simulink model "kinovaMicoSimscapeModel"  (R2021b)
settings: Solver=VariableStepAuto  StartTime=0.0  StopTime=0.3  FixedStep=0.01  RelTol=1e-3
PostLoadFcn:
  | micoRigidBodyTreeCreation;
  | IC=deg2rad([-90,180,180,0,0,0]);
  | interactiveHomePosition=deg2rad([-90 90 177.5 90 0 0]');
  | load("./KinovaMicoSimscapeVariantConfigurations.mat");
values from neighbouring files (symbols this model uses):
  micoCandlePosition = deg2rad([0,180,180,0,0,0])    [KinovaMicoSimscapeInitializeScript.m]    (also in generatingRandomTrajectory.m)
  ViaPointsTaskSpace = [ViaPointsTaskSpace;[[pi;0;pi],[pi;0;pi],[pi;0;pi],[pi;0;pi],[0;0;0],[0;0;0],[pi;0;pi]]]    [KinovaMicoSimscapeInitializeScript.m]    (also in generatingRandomTrajectory.m = [ViaPointsTaskSpace;zeros(3,7)])
undefined symbols (not defined in the file or in its folder): Mico, ViaPointsJointSpace, X, Y, Z
libraries: sm_lib x26, nesl_utility x19, robotcorelib x4, robotmaniplib x3, pid_lib x2
(part 35 of 50)

== matlab function kinovaMicoSimscapeModel/Variant Subsystem/TaskSpaceController/Sliding Adaptive Control/RegressorComputation ==
  data: dqr input; ddqr input; Y output; dq input; q input
function Y = RegressorComputation(dqr,ddqr,dq,q)
%% Unpacking terms
ddqr1=ddqr(1);
ddqr2=ddqr(2);
ddqr3=ddqr(3);
ddqr4=ddqr(4);
ddqr5=ddqr(5);
ddqr6=ddqr(6);

dqr1=dqr(1);
dqr2=dqr(2);
dqr3=dqr(3);
dqr4=dqr(4);
dqr5=dqr(5);
dqr6=dqr(6);

dq1=dq(1);
dq2=dq(2);
dq3=dq(3);
dq4=dq(4);
dq5=dq(5);
dq6=dq(6);

q1=q(1);
q2=q(2);
q3=q(3);
q4=q(4);
q5=q(5);
q6=q(6);

%% All the terms are below
Y1_1_1=ddqr1/390625;
Y1_2_1=(525657*ddqr1)/12500000 + (29*ddqr2*cos(q2))/62500 - (841*ddqr1*cos(2*q2))/20000 - (29*dq2*dqr2*sin(q2))/62500 + (841*dq1*dqr2*sin(2*q2))/20000 + (841*dq2*dqr1*sin(2*q2))/20000;
Y1_3_1=(9935161*ddqr1)/200000000 - (35699*ddqr1*cos(q3))/1000000 - (203*ddqr2*cos(q2))/100000 - (841*ddqr1*cos(2*q2))/20000 + (203*dq2*dqr2*sin(q2))/100000 + (35699*dq1*dqr3*sin(q3))/2000000 + (35699*dq3*dqr1*sin(q3))/2000000 - (1515361*ddqr1*cos(2*q2)*cos(2*q3))/200000000 - (1515361*ddqr1*sin(2*q2)*sin(2*q3))/200000000 + (841*dq1*dqr2*sin(2*q2))/20000 + (841*dq2*dqr1*sin(2*q2))/20000 + (8617*ddqr2*cos(q2)*cos(q3))/10000000 - (8617*ddqr3*cos(q2)*cos(q3))/10000000 + (8617*ddqr2*sin(q2)*sin(q3))/10000000 - (8617*ddqr3*sin(q2)*sin(q3))/10000000 + (35699*ddqr1*cos(2*q2)*cos(q3))/1000000 + (35699*ddqr1*sin(2*q2)*sin(q3))/1000000 + (35699*dq1*dqr2*cos(2*q2)*sin(q3))/1000000 - (35699*dq1*dqr2*sin(2*q2)*cos(q3))/1000000 + (35699*dq2*dqr1*cos(2*q2)*sin(q3))/1000000 - (35699*dq2*dqr1*sin(2*q2)*cos(q3))/1000000 - (35699*dq1*dqr3*cos(2*q2)*sin(q3))/2000000 + (35699*dq1*dqr3*sin(2*q2)*cos(q3))/2000000 - (35699*dq3*dqr1*cos(2*q2)*sin(q3))/2000000 + (35699*dq3*dqr1*sin(2*q2)*cos(q3))/2000000 - (1515361*dq1*dqr2*cos(2*q2)*sin(2*q3))/200000000 + (1515361*dq1*dqr2*cos(2*q3)*sin(2*q2))/200000000 - (1515361*dq2*dqr1*cos(2*q2)*sin(2*q3))/200000000 + (1515361*dq2*dqr1*cos(2*q3)*sin(2*q2))/200000000 + (1515361*dq1*dqr3*cos(2*q2)*sin(2*q3))/200000000 - (1515361*dq1*dqr3*cos(2*q3)*sin(2*q2))/200000000 + (1515361*dq3*dqr1*cos(2*q2)*sin(2*q3))/200000000 - (1515361*dq3*dqr1*cos(2*q3)*sin(2*q2))/200000000 + (8617*dq2*dqr2*cos(q2)*sin(q3))/10000000 - (8617*dq2*dqr2*cos(q3)*sin(q2))/10000000 - (8617*dq2*dqr3*cos(q2)*sin(q3))/10000000 + (8617*dq2*dqr3*cos(q3)*sin(q2))/10000000 - (8617*dq3*dqr2*cos(q2)*sin(q3))/10000000 + (8617*dq3*dqr2*cos(q3)*sin(q2))/10000000 + (8617*dq3*dqr3*cos(q2)*sin(q3))/10000000 - (8617*dq3*dqr3*cos(q3)*sin(q2))/10000000;
Y1_4_1=(203*dq2*dqr2*sin(q2))/100000 + (3393*dq1*dqr3*sin(q3))/125000 + (3393*dq3*dqr1*sin(q3))/125000 + (259*dq4*dqr1*sin(q4))/1000000 + (841*dq1*dqr2*sin(2*q2))/20000 + (841*dq2*dqr1*sin(2*q2))/20000 - (1369*dq4*dqr1*sin(2*q4))/4000000 + (3393*dq1*dqr2*cos(2*q2)*sin(q3))/62500 - (3393*dq1*dqr2*sin(2*q2)*cos(q3))/62500 + (3393*dq2*dqr1*cos(2*q2)*sin(q3))/62500 - (3393*dq2*dqr1*sin(2*q2)*cos(q3))/62500 - (3393*dq1*dqr3*cos(2*q2)*sin(q3))/125000 + (3393*dq1*dqr3*sin(2*q2)*cos(q3))/125000 - (3393*dq3*dqr1*cos(2*q2)*sin(q3))/125000 + (3393*dq3*dqr1*sin(2*q2)*cos(q3))/125000 - (1717967*dq1*dqr2*cos(2*q2)*sin(2*q3))/100000000 + (1717967*dq1*dqr2*cos(2*q3)*sin(2*q2))/100000000 - (1717967*dq2*dqr1*cos(2*q2)*sin(2*q3))/100000000 + (1717967*dq2*dqr1*cos(2*q3)*sin(2*q2))/100000000 - (1717967*dq1*dqr3*cos(2*q3)*sin(2*q2))/100000000 + (1717967*dq3*dqr1*cos(2*q2)*sin(2*q3))/100000000 - (1717967*dq3*dqr1*cos(2*q3)*sin(2*q2))/100000000 + (819*dq2*dqr2*cos(q2)*sin(q3))/625000 - (819*dq2*dqr2*cos(q3)*sin(q2))/625000 - (1073*dq2*dqr2*cos(q4)*sin(q2))/100000 - (819*dq2*dqr3*cos(q2)*sin(q3))/625000 + (819*dq2*dqr3*cos(q3)*sin(q2))/625000 - (819*dq3*dqr2*cos(q2)*sin(q3))/625000 + (819*dq3*dqr2*cos(q3)*sin(q2))/625000 + (1073*dq1*dqr3*cos(q3)*sin(q4))/200000 + (1073*dq3*dqr1*cos(q3)*sin(q4))/200000 + (819*dq3*dqr3*cos(q2)*sin(q3))/625000 - (819*dq3*dqr3*cos(q3)*sin(q2))/625000 + (1369*dq4*dqr2*cos(q2)*sin(q3))/2000000 - (1369*dq4*dqr2*cos(q3)*sin(q2))/2000000 + (1073*dq4*dqr1*cos(q4)*sin(q3))/200000 - (1369*dq4*dqr3*cos(q2)*sin(q3))/2000000 + (1369*dq4*dqr3*cos(q3)*sin(q2))/2000000 + (1073*dq1*dqr2*cos(2*q2)*cos(q3)*sin(q4))/100000 + (1073*dq2*dqr1*cos(2*q2)*cos(q3)*sin(q4))/100000 - (1073*dq1*dqr3*cos(2*q2)*cos(q3)*sin(q4))/200000 - (1369*dq2*dqr2*sin(2*q4)*cos(q2)*cos(q3))/2000000 - (1073*dq3*dqr1*cos(2*q2)*cos(q3)*sin(q4))/200000 + (1369*dq2*dqr3*sin(2*q4)*cos(q2)*cos(q3))/2000000 + (1369*dq3*dqr2*sin(2*q4)*cos(q2)*cos(q3))/2000000 - (1073*dq4*dqr1*cos(2*q2)*cos(q4)*sin(q3))/200000 + (1073*dq4*dqr1*sin(2*q2)*cos(q3)*cos(q4))/200000 - (1369*dq3*dqr3*sin(2*q4)*cos(q2)*cos(q3))/2000000 + (1369*dq4*dqr2*cos(2*q4)*cos(q2)*sin(q3))/2000000 - (1369*dq4*dqr2*cos(2*q4)*cos(q3)*sin(q2))/2000000 - (1369*dq4*dqr3*cos(2*q4)*cos(q2)*sin(q3))/2000000 + (1369*dq4*dqr3*cos(2*q4)*cos(q3)*sin(q2))/2000000 + (1073*dq1*dqr2*sin(2*q2)*sin(q3)*sin(q4))/100000 + (1073*dq2*dqr1*sin(2*q2)*sin(q3)*sin(q4))/100000 - (1073*dq1*dqr3*sin(2*q2)*sin(q3)*sin(q4))/200000 - (1369*dq2*dqr2*sin(2*q4)*sin(q2)*sin(q3))/2000000 - (1073*dq3*dqr1*sin(2*q2)*sin(q3)*sin(q4))/200000 + (1369*dq2*dqr3*sin(2*q4)*sin(q2)*sin(q3))/2000000 + (1369*dq3*dqr2*sin(2*q4)*sin(q2)*sin(q3))/2000000 - (1369*dq3*dqr3*sin(2*q4)*sin(q2)*sin(q3))/2000000 - (4329*dq1*dqr2*cos(2*q2)*cos(2*q3)*sin(q4))/625000 - (4329*dq2*dqr1*cos(2*q2)*cos(2*q3)*sin(q4))/625000 + (4329*dq1*dqr3*cos(2*q2)*cos(2*q3)*sin(q4))/625000 + (4329*dq3*dqr1*cos(2*q2)*cos(2*q3)*sin(q4))/625000 + (4329*dq4*dqr1*cos(2*q2)*sin(2*q3)*cos(q4))/1250000 - (4329*dq4*dqr1*cos(2*q3)*sin(2*q2)*cos(q4))/1250000 - (4329*dq1*dqr2*sin(2*q2)*sin(2*q3)*sin(q4))/625000 - (4329*dq2*dqr1*sin(2*q2)*sin(2*q3)*sin(q4))/625000 + (4329*dq1*dqr3*sin(2*q2)*sin(2*q3)*sin(q4))/625000 + (4329*dq3*dqr1*sin(2*q2)*sin(2*q3)*sin(q4))/625000 + (259*dq2*dqr2*cos(q2)*cos(q3)*sin(q4))/1000000 - (4329*dq2*dqr2*cos(q2)*cos(q4)*sin(q3))/625000 + (4329*dq2*dqr2*cos(q3)*cos(q4)*sin(q2))/625000 - (259*dq2*dqr3*cos(q2)*cos(q3)*sin(q4))/1000000 + (4329*dq2*dqr3*cos(q2)*cos(q4)*sin(q3))/625000 - (4329*dq2*dqr3*cos(q3)*cos(q4)*sin(q2))/625000 - (259*dq3*dqr2*cos(q2)*cos(q3)*sin(q4))/1000000 + (4329*dq3*dqr2*cos(q2)*cos(q4)*sin(q3))/625000 - (4329*dq3*dqr2*cos(q3)*cos(q4)*sin(q2))/625000 + (259*dq3*dqr3*cos(q2)*cos(q3)*sin(q4))/1000000 - (4329*dq3*dqr3*cos(q2)*cos(q4)*sin(q3))/625000 + (4329*dq3*dqr3*cos(q3)*cos(q4)*sin(q2))/625000 - (259*dq4*dqr2*cos(q2)*cos(q4)*sin(q3))/1000000 + (259*dq4*dqr2*cos(q3)*cos(q4)*sin(q2))/1000000 + (259*dq4*dqr3*cos(q2)*cos(q4)*sin(q3))/1000000 - (259*dq4*dqr3*cos(q3)*cos(q4)*sin(q2))/1000000 - (1369*dq1*dqr2*cos(2*q2)*cos(2*q4)*sin(2*q3))/4000000 + (1369*dq1*dqr2*cos(2*q3)*cos(2*q4)*sin(2*q2))/4000000 - (1369*dq2*dqr1*cos(2*q2)*cos(2*q4)*sin(2*q3))/4000000 + (1369*dq2*dqr1*cos(2*q3)*cos(2*q4)*sin(2*q2))/4000000 + (1369*dq1*dqr3*cos(2*q2)*cos(2*q4)*sin(2*q3))/4000000 - (1369*dq1*dqr3*cos(2*q3)*cos(2*q4)*sin(2*q2))/4000000 + (1369*dq3*dqr1*cos(2*q2)*cos(2*q4)*sin(2*q3))/4000000 - (1369*dq3*dqr1*cos(2*q3)*cos(2*q4)*sin(2*q2))/4000000 + (1369*dq4*dqr1*cos(2*q2)*cos(2*q3)*sin(2*q4))/4000000 + (259*dq2*dqr2*sin(q2)*sin(q3)*sin(q4))/1000000 - (259*dq2*dqr3*sin(q2)*sin(q3)*sin(q4))/1000000 - (259*dq3*dqr2*sin(q2)*sin(q3)*sin(q4))/1000000 + (259*dq3*dqr3*sin(q2)*sin(q3)*sin(q4))/1000000 + (1369*dq4*dqr1*sin(2*q2)*sin(2*q3)*sin(2*q4))/4000000;
Y1_4_2=(6064767*ddqr1)/100000000 - (3393*ddqr1*cos(q3))/62500 - (203*ddqr2*cos(q2))/100000 - (259*ddqr1*cos(q4))/500000 - (841*ddqr1*cos(2*q2))/20000 + (1369*ddqr1*cos(2*q4))/4000000 + (259*dq1*dqr4*sin(q4))/1000000 - (1717967*ddqr1*cos(2*q2)*cos(2*q3))/100000000 - (1717967*ddqr1*sin(2*q2)*sin(2*q3))/100000000 - (1369*dq1*dqr4*sin(2*q4))/4000000 + (819*ddqr2*cos(q2)*cos(q3))/625000 + (1073*ddqr2*cos(q2)*cos(q4))/100000 - (819*ddqr3*cos(q2)*cos(q3))/625000 + (1369*ddqr4*cos(q2)*cos(q3))/1000000 + (819*ddqr2*sin(q2)*sin(q3))/625000 + (1073*ddqr1*sin(q3)*sin(q4))/100000 - (819*ddqr3*sin(q2)*sin(q3))/625000 + (1369*ddqr4*sin(q2)*sin(q3))/1000000 + (1073*ddqr4*sin(q2)*sin(q4))/100000 + (3393*ddqr1*cos(2*q2)*cos(q3))/62500 + (3393*ddqr1*sin(2*q2)*sin(q3))/62500 + (4329*ddqr1*cos(2*q2)*sin(2*q3)*sin(q4))/625000 - (4329*ddqr1*cos(2*q3)*sin(2*q2)*sin(q4))/625000 - (4329*ddqr2*cos(q2)*cos(q3)*cos(q4))/625000 + (4329*ddqr3*cos(q2)*cos(q3)*cos(q4))/625000 - (259*ddqr4*cos(q2)*cos(q3)*cos(q4))/1000000 - (1369*ddqr1*cos(2*q2)*cos(2*q3)*cos(2*q4))/4000000 - (259*ddqr2*cos(q2)*sin(q3)*sin(q4))/1000000 + (259*ddqr2*cos(q3)*sin(q2)*sin(q4))/1000000 - (4329*ddqr2*cos(q4)*sin(q2)*sin(q3))/625000 + (259*ddqr3*cos(q2)*sin(q3)*sin(q4))/1000000 - (259*ddqr3*cos(q3)*sin(q2)*sin(q4))/1000000 + (4329*ddqr3*cos(q4)*sin(q2)*sin(q3))/625000 + (4329*ddqr4*cos(q2)*sin(q3)*sin(q4))/625000 - (4329*ddqr4*cos(q3)*sin(q2)*sin(q4))/625000 - (259*ddqr4*cos(q4)*sin(q2)*sin(q3))/1000000 - (1369*ddqr1*cos(2*q4)*sin(2*q2)*sin(2*q3))/4000000 + (1717967*dq1*dqr3*cos(2*q2)*sin(2*q3))/100000000 - (1073*ddqr1*cos(2*q2)*sin(q3)*sin(q4))/100000 + (1073*ddqr1*sin(2*q2)*cos(q3)*sin(q4))/100000 + (1369*ddqr2*sin(2*q4)*cos(q2)*sin(q3))/2000000 - (1369*ddqr2*sin(2*q4)*cos(q3)*sin(q2))/2000000 - (1369*ddqr3*sin(2*q4)*cos(q2)*sin(q3))/2000000 + (1369*ddqr3*sin(2*q4)*cos(q3)*sin(q2))/2000000 + (1369*dq2*dqr4*cos(q2)*sin(q3))/2000000 - (1369*dq2*dqr4*cos(q3)*sin(q2))/2000000 + (1073*dq1*dqr4*cos(q4)*sin(q3))/200000 - (1369*dq3*dqr4*cos(q2)*sin(q3))/2000000 + (1369*dq3*dqr4*cos(q3)*sin(q2))/2000000 + (1073*dq4*dqr4*cos(q4)*sin(q2))/100000 - (1073*dq1*dqr4*cos(2*q2)*cos(q4)*sin(q3))/200000 + (1073*dq1*dqr4*sin(2*q2)*cos(q3)*cos(q4))/200000 + (1369*dq2*dqr4*cos(2*q4)*cos(q2)*sin(q3))/2000000 - (1369*dq2*dqr4*cos(2*q4)*cos(q3)*sin(q2))/2000000 - (1369*dq3*dqr4*cos(2*q4)*cos(q2)*sin(q3))/2000000 + (1369*dq3*dqr4*cos(2*q4)*cos(q3)*sin(q2))/2000000 + (4329*dq1*dqr4*cos(2*q2)*sin(2*q3)*cos(q4))/1250000 - (4329*dq1*dqr4*cos(2*q3)*sin(2*q2)*cos(q4))/1250000 - (259*dq2*dqr4*cos(q2)*cos(q4)*sin(q3))/1000000 + (259*dq2*dqr4*cos(q3)*cos(q4)*sin(q2))/1000000 + (259*dq3*dqr4*cos(q2)*cos(q4)*sin(q3))/1000000 - (259*dq3*dqr4*cos(q3)*cos(q4)*sin(q2))/1000000 + (259*dq4*dqr4*cos(q2)*cos(q3)*sin(q4))/1000000 + (4329*dq4*dqr4*cos(q2)*cos(q4)*sin(q3))/625000 - (4329*dq4*dqr4*cos(q3)*cos(q4)*sin(q2))/625000 + (1369*dq1*dqr4*cos(2*q2)*cos(2*q3)*sin(2*q4))/4000000 + (259*dq4*dqr4*sin(q2)*sin(q3)*sin(q4))/1000000 + (1369*dq1*dqr4*sin(2*q2)*sin(2*q3)*sin(2*q4))/4000000;
Y1_5_1=(25433*dq3*dqr1*sin(q3))/800000 + dq4*dqr1*sin(q4)*((4487*3^(1/2))/20000000 + 259/1000000) - dq5*dqr1*sin(q5)*((253339*3^(1/2))/160000000 - 4107/8000000) + (25433*dq2*dqr1*cos(2*q2)*sin(q3))/400000 - (25433*dq2*dqr1*sin(2*q2)*cos(q3))/400000 - (25433*dq3*dqr1*cos(2*q2)*sin(q3))/800000 + (25433*dq3*dqr1*sin(2*q2)*cos(q3))/800000 - (259*dq4*dqr1*cos(q4)*sin(q5))/1000000 - (259*dq4*dqr1*cos(q5)*sin(q4))/2000000 - (259*dq5*dqr1*cos(q4)*sin(q5))/2000000 - (259*dq5*dqr1*cos(q5)*sin(q4))/1000000 + (1073*3^(1/2)*dq3*dqr1*cos(q5)*sin(q3))/400000 + (1073*3^(1/2)*dq5*dqr1*cos(q3)*sin(q5))/400000 + dq4*dqr1*cos(2*q4)*sin(q5)*((23717*3^(1/2))/40000000 + 1369/2000000) + dq5*dqr1*cos(2*q4)*sin(q5)*((23717*3^(1/2))/160000000 + 1369/8000000) - (1073*dq3*dqr1*cos(q3)*cos(q4)*sin(q5))/200000 - (1073*dq3*dqr1*cos(q3)*cos(q5)*sin(q4))/400000 - (1073*dq4*dqr1*cos(q4)*cos(q5)*sin(q3))/400000 - (1073*dq5*dqr1*cos(q4)*cos(q5)*sin(q3))/200000 + (1073*dq4*dqr1*sin(q3)*sin(q4)*sin(q5))/200000 + (1073*dq5*dqr1*sin(q3)*sin(q4)*sin(q5))/400000 + dq3*dqr1*cos(q3)*sin(q4)*((18589*3^(1/2))/4000000 + 1073/200000) + dq4*dqr1*cos(q4)*sin(q3)*((18589*3^(1/2))/4000000 + 1073/200000) - (1073*dq2*dqr1*sin(2*q2)*cos(q4)*sin(q3)*sin(q5))/100000 - (1073*dq2*dqr1*sin(2*q2)*cos(q5)*sin(q3)*sin(q4))/200000 + (1073*dq3*dqr1*sin(2*q2)*cos(q4)*sin(q3)*sin(q5))/200000 + (1073*dq3*dqr1*sin(2*q2)*cos(q5)*sin(q3)*sin(q4))/400000 - (1073*dq4*dqr1*cos(2*q2)*sin(q3)*sin(q4)*sin(q5))/200000 + (1073*dq4*dqr1*sin(2*q2)*cos(q3)*sin(q4)*sin(q5))/200000 - (1073*dq5*dqr1*cos(2*q2)*sin(q3)*sin(q4)*sin(q5))/400000 + (1073*dq5*dqr1*sin(2*q2)*cos(q3)*sin(q4)*sin(q5))/400000 + dq2*dqr1*cos(2*q2)*cos(q3)*sin(q4)*((18589*3^(1/2))/2000000 + 1073/100000) - dq3*dqr1*cos(2*q2)*cos(q3)*sin(q4)*((18589*3^(1/2))/4000000 + 1073/200000) - dq4*dqr1*cos(2*q2)*cos(q4)*sin(q3)*((18589*3^(1/2))/4000000 + 1073/200000) + dq4*dqr1*sin(2*q2)*cos(q3)*cos(q4)*((18589*3^(1/2))/4000000 + 1073/200000) + (32449*dq2*dqr1*cos(2*q2)*cos(2*q3)*cos(q4)*sin(q5))/4000000 - (32449*dq3*dqr1*cos(2*q2)*cos(2*q3)*cos(q4)*sin(q5))/4000000 - (32449*dq5*dqr1*cos(2*q2)*sin(2*q3)*cos(q4)*cos(q5))/8000000 + (32449*dq5*dqr1*cos(2*q3)*sin(2*q2)*cos(q4)*cos(q5))/8000000 + dq2*dqr1*sin(2*q2)*sin(q3)*sin(q4)*((18589*3^(1/2))/2000000 + 1073/100000) - dq3*dqr1*sin(2*q2)*sin(q3)*sin(q4)*((18589*3^(1/2))/4000000 + 1073/200000) + (32449*dq2*dqr1*sin(2*q2)*sin(2*q3)*cos(q4)*sin(q5))/4000000 - (32449*dq3*dqr1*sin(2*q2)*sin(2*q3)*cos(q4)*sin(q5))/4000000 + (32449*dq4*dqr1*cos(2*q2)*sin(2*q3)*sin(q4)*sin(q5))/8000000 - (32449*dq4*dqr1*cos(2*q3)*sin(2*q2)*sin(q4)*sin(q5))/8000000 + (1073*3^(1/2)*dq2*dqr1*cos(2*q2)*cos(q5)*sin(q3))/200000 - (1073*3^(1/2)*dq2*dqr1*sin(2*q2)*cos(q3)*cos(q5))/200000 - (1073*3^(1/2)*dq3*dqr1*cos(2*q2)*cos(q5)*sin(q3))/400000 + (1073*3^(1/2)*dq3*dqr1*sin(2*q2)*cos(q3)*cos(q5))/400000 - (1073*3^(1/2)*dq5*dqr1*cos(2*q2)*cos(q3)*sin(q5))/400000 - (1073*3^(1/2)*dq5*dqr1*sin(2*q2)*sin(q3)*sin(q5))/400000 - dq2*dqr1*cos(2*q2)*cos(2*q3)*sin(q4)*((548467*3^(1/2))/80000000 + 32449/4000000) + dq3*dqr1*cos(2*q2)*cos(2*q3)*sin(q4)*((548467*3^(1/2))/80000000 + 32449/4000000) + dq5*dqr1*cos(2*q2)*cos(2*q3)*sin(q5)*((348207*3^(1/2))/160000000 + 1369/8000000) + dq4*dqr1*cos(2*q2)*sin(2*q3)*cos(q4)*((548467*3^(1/2))/160000000 + 32449/8000000) - dq4*dqr1*cos(2*q3)*sin(2*q2)*cos(q4)*((548467*3^(1/2))/160000000 + 32449/8000000) - dq2*dqr1*sin(2*q2)*sin(2*q3)*sin(q4)*((548467*3^(1/2))/80000000 + 32449/4000000) + dq3*dqr1*sin(2*q2)*sin(2*q3)*sin(q4)*((548467*3^(1/2))/80000000 + 32449/4000000) + dq5*dqr1*sin(2*q2)*sin(2*q3)*sin(q5)*((348207*3^(1/2))/160000000 + 1369/8000000) - (1073*dq2*dqr1*cos(2*q2)*cos(q3)*cos(q4)*sin(q5))/100000 - (1073*dq2*dqr1*cos(2*q2)*cos(q3)*cos(q5)*sin(q4))/200000 + (1073*dq3*dqr1*cos(2*q2)*cos(q3)*cos(q4)*sin(q5))/200000 + (1073*dq3*dqr1*cos(2*q2)*cos(q3)*cos(q5)*sin(q4))/400000 + (1073*dq4*dqr1*cos(2*q2)*cos(q4)*cos(q5)*sin(q3))/400000 - (1073*dq4*dqr1*sin(2*q2)*cos(q3)*cos(q4)*cos(q5))/400000 + (1073*dq5*dqr1*cos(2*q2)*cos(q4)*cos(q5)*sin(q3))/200000 - (1073*dq5*dqr1*sin(2*q2)*cos(q3)*cos(q4)*cos(q5))/200000 + (1369*3^(1/2)*dq2*dqr1*cos(2*q2)*cos(2*q3)*cos(2*q5)*sin(q4))/8000000 + (1369*3^(1/2)*dq2*dqr1*cos(2*q2)*cos(2*q3)*sin(2*q5)*cos(q4))/4000000 - (1369*3^(1/2)*dq3*dqr1*cos(2*q2)*cos(2*q3)*cos(2*q5)*sin(q4))/8000000 - (1369*3^(1/2)*dq3*dqr1*cos(2*q2)*cos(2*q3)*sin(2*q5)*cos(q4))/4000000 - (1369*3^(1/2)*dq4*dqr1*cos(2*q2)*cos(2*q5)*sin(2*q3)*cos(q4))/16000000 + (1369*3^(1/2)*dq4*dqr1*cos(2*q3)*cos(2*q5)*sin(2*q2)*cos(q4))/16000000 - (1369*3^(1/2)*dq5*dqr1*cos(2*q2)*cos(2*q5)*sin(2*q3)*cos(q4))/4000000 + (1369*3^(1/2)*dq5*dqr1*cos(2*q3)*cos(2*q5)*sin(2*q2)*cos(q4))/4000000 + (1369*3^(1/2)*dq2*dqr1*cos(2*q5)*sin(2*q2)*sin(2*q3)*sin(q4))/8000000 + (1369*3^(1/2)*dq2*dqr1*sin(2*q2)*sin(2*q3)*sin(2*q5)*cos(q4))/4000000 - (1369*3^(1/2)*dq3*dqr1*cos(2*q5)*sin(2*q2)*sin(2*q3)*sin(q4))/8000000 - (1369*3^(1/2)*dq3*dqr1*sin(2*q2)*sin(2*q3)*sin(2*q5)*cos(q4))/4000000 + (1369*3^(1/2)*dq4*dqr1*cos(2*q2)*sin(2*q3)*sin(2*q5)*sin(q4))/8000000 - (1369*3^(1/2)*dq4*dqr1*cos(2*q3)*sin(2*q2)*sin(2*q5)*sin(q4))/8000000 + (1369*3^(1/2)*dq5*dqr1*cos(2*q2)*sin(2*q3)*sin(2*q5)*sin(q4))/8000000 - (1369*3^(1/2)*dq5*dqr1*cos(2*q3)*sin(2*q2)*sin(2*q5)*sin(q4))/8000000 - dq2*dqr1*cos(2*q2)*cos(2*q3)*cos(q5)*sin(q4)*((1369*3^(1/2))/2000000 - 45547/20000000) + dq3*dqr1*cos(2*q2)*cos(2*q3)*cos(q5)*sin(q4)*((1369*3^(1/2))/2000000 - 45547/20000000) + dq4*dqr1*cos(2*q2)*sin(2*q3)*cos(q4)*cos(q5)*((1369*3^(1/2))/4000000 - 45547/40000000) - dq4*dqr1*cos(2*q3)*sin(2*q2)*cos(q4)*cos(q5)*((1369*3^(1/2))/4000000 - 45547/40000000) - dq2*dqr1*sin(2*q2)*sin(2*q3)*cos(q5)*sin(q4)*((1369*3^(1/2))/2000000 - 45547/20000000) + dq3*dqr1*sin(2*q2)*sin(2*q3)*cos(q5)*sin(q4)*((1369*3^(1/2))/2000000 - 45547/20000000) - dq5*dqr1*cos(2*q2)*sin(2*q3)*sin(q4)*sin(q5)*((1369*3^(1/2))/4000000 - 45547/40000000) + dq5*dqr1*cos(2*q3)*sin(2*q2)*sin(q4)*sin(q5)*((1369*3^(1/2))/4000000 - 45547/40000000) - dq4*dqr1*cos(2*q2)*cos(2*q3)*cos(2*q4)*sin(q5)*((23717*3^(1/2))/40000000 + 1369/2000000) - dq2*dqr1*cos(2*q3)*cos(2*q4)*sin(2*q2)*cos(q5)*((23717*3^(1/2))/80000000 + 1369/4000000) - dq5*dqr1*cos(2*q2)*cos(2*q3)*cos(2*q4)*sin(q5)*((23717*3^(1/2))/160000000 + 1369/8000000) - dq2*dqr1*cos(2*q2)*sin(2*q3)*sin(2*q4)*sin(q5)*((23717*3^(1/2))/40000000 + 1369/2000000) + dq2*dqr1*cos(2*q3)*sin(2*q2)*sin(2*q4)*sin(q5)*((23717*3^(1/2))/40000000 + 1369/2000000) + dq3*dqr1*cos(2*q2)*sin(2*q3)*sin(2*q4)*sin(q5)*((23717*3^(1/2))/40000000 + 1369/2000000) - dq3*dqr1*cos(2*q3)*sin(2*q2)*sin(2*q4)*sin(q5)*((23717*3^(1/2))/40000000 + 1369/2000000) - dq4*dqr1*cos(2*q4)*sin(2*q2)*sin(2*q3)*sin(q5)*((23717*3^(1/2))/40000000 + 1369/2000000) - dq5*dqr1*cos(2*q4)*sin(2*q2)*sin(2*q3)*sin(q5)*((23717*3^(1/2))/160000000 + 1369/8000000);
Y1_5_2=(841*dq2*dqr1*sin(2*q2))/20000 + (4107*dq5*dqr1*sin(2*q5))/32000000 - (1369*dq4*dqr1*cos(2*q4)*sin(2*q5))/8000000 - (1369*dq4*dqr1*cos(2*q5)*sin(2*q4))/6400000 - (1369*dq5*dqr1*cos(2*q4)*sin(2*q5))/6400000 - (1369*dq5*dqr1*cos(2*q5)*sin(2*q4))/8000000 - (6139*dq2*dqr2*cos(q3)*sin(q2))/4000000 + (6139*dq3*dqr2*cos(q3)*sin(q2))/4000000 - dq4*dqr1*sin(2*q4)*((23717*3^(1/2))/40000000 + 1574893/1600000000) + dq2*dqr1*cos(2*q2)*sin(2*q3)*((23717*3^(1/2))/40000000 - 36744657/1600000000) - dq2*dqr1*cos(2*q3)*sin(2*q2)*((23717*3^(1/2))/40000000 - 36744657/1600000000) - dq3*dqr1*cos(2*q2)*sin(2*q3)*((23717*3^(1/2))/40000000 - 36744657/1600000000) + dq3*dqr1*cos(2*q3)*sin(2*q2)*((23717*3^(1/2))/40000000 - 36744657/1600000000) + dq4*dqr1*sin(2*q4)*cos(q5)*((23717*3^(1/2))/80000000 + 1369/4000000) + dq5*dqr1*sin(2*q4)*cos(q5)*((23717*3^(1/2))/80000000 + 1369/4000000) - (12321*dq2*dqr1*cos(2*q2)*cos(2*q5)*sin(2*q3))/32000000 + (12321*dq2*dqr1*cos(2*q3)*cos(2*q5)*sin(2*q2))/32000000 + (12321*dq3*dqr1*cos(2*q2)*cos(2*q5)*sin(2*q3))/32000000 - (12321*dq3*dqr1*cos(2*q3)*cos(2*q5)*sin(2*q2))/32000000 + (12321*dq5*dqr1*cos(2*q2)*cos(2*q3)*sin(2*q5))/32000000 - (1073*dq2*dqr2*sin(q2)*sin(q4)*sin(q5))/100000 + (12321*dq5*dqr1*sin(2*q2)*sin(2*q3)*sin(2*q5))/32000000 - (1369*dq2*dqr1*cos(2*q2)*cos(2*q4)*cos(2*q5)*sin(2*q3))/6400000 + (1369*dq2*dqr1*cos(2*q3)*cos(2*q4)*cos(2*q5)*sin(2*q2))/6400000 + (1369*dq3*dqr1*cos(2*q2)*cos(2*q4)*cos(2*q5)*sin(2*q3))/6400000 - (1369*dq3*dqr1*cos(2*q3)*cos(2*q4)*cos(2*q5)*sin(2*q2))/6400000 + (1369*dq4*dqr1*cos(2*q2)*cos(2*q3)*cos(2*q4)*sin(2*q5))/8000000 + (1369*dq4*dqr1*cos(2*q2)*cos(2*q3)*cos(2*q5)*sin(2*q4))/6400000 + (1369*dq5*dqr1*cos(2*q2)*cos(2*q3)*cos(2*q4)*sin(2*q5))/6400000 + (1369*dq5*dqr1*cos(2*q2)*cos(2*q3)*cos(2*q5)*sin(2*q4))/8000000 - (259*3^(1/2)*dq2*dqr2*cos(q3)*cos(q5)*sin(q2))/2000000 + (259*3^(1/2)*dq3*dqr2*cos(q3)*cos(q5)*sin(q2))/2000000 + (1369*dq2*dqr1*cos(2*q2)*sin(2*q3)*sin(2*q4)*sin(2*q5))/8000000 - (1369*dq2*dqr1*cos(2*q3)*sin(2*q2)*sin(2*q4)*sin(2*q5))/8000000 - (1369*dq3*dqr1*cos(2*q2)*sin(2*q3)*sin(2*q4)*sin(2*q5))/8000000 + (1369*dq3*dqr1*cos(2*q3)*sin(2*q2)*sin(2*q4)*sin(2*q5))/8000000 + (1369*dq4*dqr1*cos(2*q4)*sin(2*q2)*sin(2*q3)*sin(2*q5))/8000000 + (1369*dq4*dqr1*cos(2*q5)*sin(2*q2)*sin(2*q3)*sin(2*q4))/6400000 + (1369*dq5*dqr1*cos(2*q4)*sin(2*q2)*sin(2*q3)*sin(2*q5))/6400000 + (1369*dq5*dqr1*cos(2*q5)*sin(2*q2)*sin(2*q3)*sin(2*q4))/8000000 + (1369*3^(1/2)*dq5*dqr2*sin(q2)*sin(q3)*sin(q4))/4000000 - (259*3^(1/2)*dq5*dqr2*sin(q2)*sin(q3)*sin(q5))/2000000 - dq2*dqr1*cos(2*q2)*cos(2*q4)*sin(2*q3)*((23717*3^(1/2))/40000000 + 1574893/1600000000) + dq2*dqr1*cos(2*q3)*cos(2*q4)*sin(2*q2)*((23717*3^(1/2))/40000000 + 1574893/1600000000) + dq3*dqr1*cos(2*q2)*cos(2*q4)*sin(2*q3)*((23717*3^(1/2))/40000000 + 1574893/1600000000) - dq3*dqr1*cos(2*q3)*cos(2*q4)*sin(2*q2)*((23717*3^(1/2))/40000000 + 1574893/1600000000) + dq4*dqr1*cos(2*q2)*cos(2*q3)*sin(2*q4)*((23717*3^(1/2))/40000000 + 1574893/1600000000) - (1369*dq2*dqr2*cos(2*q4)*sin(2*q5)*sin(q2)*sin(q3))/4000000 - (1369*dq2*dqr2*cos(2*q5)*sin(2*q4)*sin(q2)*sin(q3))/3200000 + (1369*dq3*dqr2*cos(2*q4)*sin(2*q5)*sin(q2)*sin(q3))/4000000 + (1369*dq3*dqr2*cos(2*q5)*sin(2*q4)*sin(q2)*sin(q3))/3200000 + (1369*dq4*dqr2*sin(2*q4)*sin(2*q5)*cos(q3)*sin(q2))/4000000 + dq4*dqr1*sin(2*q2)*sin(2*q3)*sin(2*q4)*((23717*3^(1/2))/40000000 + 1574893/1600000000) - dq2*dqr2*sin(2*q4)*sin(q2)*sin(q3)*((23717*3^(1/2))/20000000 + 1574893/800000000) + dq3*dqr2*sin(2*q4)*sin(q2)*sin(q3)*((23717*3^(1/2))/20000000 + 1574893/800000000) - (259*dq4*dqr2*cos(q3)*cos(q4)*cos(q5)*sin(q2))/2000000 - (259*dq5*dqr2*cos(q3)*cos(q4)*cos(q5)*sin(q2))/1000000 - dq2*dqr1*cos(2*q2)*sin(2*q3)*cos(q5)*((348207*3^(1/2))/80000000 + 1369/4000000) + dq2*dqr1*cos(2*q3)*sin(2*q2)*cos(q5)*((348207*3^(1/2))/80000000 + 1369/4000000) + dq3*dqr1*cos(2*q2)*sin(2*q3)*cos(q5)*((348207*3^(1/2))/80000000 + 1369/4000000) - dq3*dqr1*cos(2*q3)*sin(2*q2)*cos(q5)*((348207*3^(1/2))/80000000 + 1369/4000000) + (32449*dq2*dqr2*cos(q3)*sin(q2)*sin(q4)*sin(q5))/4000000 - (259*dq2*dqr2*cos(q4)*sin(q2)*sin(q3)*sin(q5))/1000000 - (259*dq2*dqr2*cos(q5)*sin(q2)*sin(q3)*sin(q4))/2000000 - (32449*dq3*dqr2*cos(q3)*sin(q2)*sin(q4)*sin(q5))/4000000 + (259*dq3*dqr2*cos(q4)*sin(q2)*sin(q3)*sin(q5))/1000000 + (259*dq3*dqr2*cos(q5)*sin(q2)*sin(q3)*sin(q4))/2000000 + (259*dq4*dqr2*cos(q3)*sin(q2)*sin(q4)*sin(q5))/1000000 + (259*dq5*dqr2*cos(q3)*sin(q2)*sin(q4)*sin(q5))/2000000 + dq4*dqr2*cos(q3)*cos(q4)*sin(q2)*((4487*3^(1/2))/20000000 + 259/1000000) + dq4*dqr2*cos(q3)*cos(q5)*sin(q2)*((23717*3^(1/2))/40000000 + 1369/2000000) + dq5*dqr2*cos(q3)*cos(q5)*sin(q2)*((23717*3^(1/2))/40000000 + 1369/2000000) + dq2*dqr2*cos(q3)*cos(q4)*sin(q2)*((548467*3^(1/2))/80000000 + 32449/4000000) - dq3*dqr2*cos(q3)*cos(q4)*sin(q2)*((548467*3^(1/2))/80000000 + 32449/4000000) + dq2*dqr2*sin(q2)*sin(q3)*sin(q4)*((4487*3^(1/2))/20000000 + 259/1000000) - dq3*dqr2*sin(q2)*sin(q3)*sin(q4)*((4487*3^(1/2))/20000000 + 259/1000000) + dq4*dqr2*cos(2*q4)*cos(q3)*cos(q5)*sin(q2)*((23717*3^(1/2))/40000000 + 1369/2000000) + dq5*dqr2*cos(2*q4)*cos(q3)*cos(q5)*sin(q2)*((23717*3^(1/2))/40000000 + 1369/2000000) + dq2*dqr2*cos(2*q4)*sin(q2)*sin(q3)*sin(q5)*((23717*3^(1/2))/20000000 + 1369/1000000) - dq3*dqr2*cos(2*q4)*sin(q2)*sin(q3)*sin(q5)*((23717*3^(1/2))/20000000 + 1369/1000000) - dq4*dqr2*sin(2*q4)*cos(q3)*sin(q2)*sin(q5)*((23717*3^(1/2))/20000000 + 1369/1000000) + dq2*dqr2*sin(2*q4)*cos(q5)*sin(q2)*sin(q3)*((23717*3^(1/2))/40000000 + 1369/2000000) - dq3*dqr2*sin(2*q4)*cos(q5)*sin(q2)*sin(q3)*((23717*3^(1/2))/40000000 + 1369/2000000) - dq5*dqr2*sin(2*q4)*cos(q3)*sin(q2)*sin(q5)*((23717*3^(1/2))/80000000 + 1369/4000000) - (1369*3^(1/2)*dq2*dqr2*cos(2*q5)*cos(q3)*cos(q4)*sin(q2))/8000000 + (1369*3^(1/2)*dq3*dqr2*cos(2*q5)*cos(q3)*cos(q4)*sin(q2))/8000000 + (1369*3^(1/2)*dq2*dqr2*sin(2*q5)*cos(q3)*sin(q2)*sin(q4))/4000000 - (1369*3^(1/2)*dq3*dqr2*sin(2*q5)*cos(q3)*sin(q2)*sin(q4))/4000000 - (1369*3^(1/2)*dq5*dqr2*cos(2*q5)*sin(q2)*sin(q3)*sin(q4))/4000000 - (1369*3^(1/2)*dq5*dqr2*sin(2*q5)*cos(q4)*sin(q2)*sin(q3))/8000000 + dq2*dqr2*cos(q3)*cos(q4)*cos(q5)*sin(q2)*((1369*3^(1/2))/2000000 - 45547/20000000) - dq3*dqr2*cos(q3)*cos(q4)*cos(q5)*sin(q2)*((1369*3^(1/2))/2000000 - 45547/20000000) + dq5*dqr2*cos(q4)*sin(q2)*sin(q3)*sin(q5)*((1369*3^(1/2))/2000000 + 71151/40000000) + dq2*dqr1*cos(2*q2)*cos(2*q4)*sin(2*q3)*cos(q5)*((23717*3^(1/2))/80000000 + 1369/4000000) - dq3*dqr1*cos(2*q2)*cos(2*q4)*sin(2*q3)*cos(q5)*((23717*3^(1/2))/80000000 + 1369/4000000) + dq3*dqr1*cos(2*q3)*cos(2*q4)*sin(2*q2)*cos(q5)*((23717*3^(1/2))/80000000 + 1369/4000000) - dq4*dqr1*cos(2*q2)*cos(2*q3)*sin(2*q4)*cos(q5)*((23717*3^(1/2))/80000000 + 1369/4000000) - dq5*dqr1*cos(2*q2)*cos(2*q3)*sin(2*q4)*cos(q5)*((23717*3^(1/2))/80000000 + 1369/4000000) - dq4*dqr1*sin(2*q2)*sin(2*q3)*sin(2*q4)*cos(q5)*((23717*3^(1/2))/80000000 + 1369/4000000) - dq5*dqr1*sin(2*q2)*sin(2*q3)*sin(2*q4)*cos(q5)*((23717*3^(1/2))/80000000 + 1369/4000000);
Y1_5_3=(203*dq2*dqr2*sin(q2))/100000 + (841*dq1*dqr2*sin(2*q2))/20000 + (25433*dq1*dqr2*cos(2*q2)*sin(q3))/400000 - (25433*dq1*dqr2*sin(2*q2)*cos(q3))/400000 + (6139*dq2*dqr2*cos(q2)*sin(q3))/4000000 - (6139*dq3*dqr2*cos(q2)*sin(q3))/4000000 + (1369*dq5*dqr2*cos(q2)*sin(q3))/4000000 - (1369*dq5*dqr2*cos(q3)*sin(q2))/4000000 - (4107*dq4*dqr2*cos(2*q5)*cos(q2)*sin(q3))/16000000 + (4107*dq4*dqr2*cos(2*q5)*cos(q3)*sin(q2))/16000000 - dq1*dqr2*cos(2*q3)*sin(2*q2)*((23717*3^(1/2))/40000000 - 36744657/1600000000) + dq4*dqr2*cos(q2)*sin(q3)*((23717*3^(1/2))/20000000 + 2122493/800000000) - dq4*dqr2*cos(q3)*sin(q2)*((23717*3^(1/2))/20000000 + 2122493/800000000) + (1073*dq2*dqr2*cos(q4)*cos(q5)*sin(q2))/200000 - (12321*dq1*dqr2*cos(2*q2)*cos(2*q5)*sin(2*q3))/32000000 + (12321*dq1*dqr2*cos(2*q3)*cos(2*q5)*sin(2*q2))/32000000 - dq2*dqr2*cos(q4)*sin(q2)*((18589*3^(1/2))/2000000 + 1073/100000) - (1369*dq1*dqr2*cos(2*q2)*cos(2*q4)*cos(2*q5)*sin(2*q3))/6400000 + (1369*dq1*dqr2*cos(2*q3)*cos(2*q4)*cos(2*q5)*sin(2*q2))/6400000 - (1073*dq1*dqr2*sin(2*q2)*cos(q4)*sin(q3)*sin(q5))/100000 - (1073*dq1*dqr2*sin(2*q2)*cos(q5)*sin(q3)*sin(q4))/200000 + (259*3^(1/2)*dq2*dqr2*cos(q2)*cos(q5)*sin(q3))/2000000 - (259*3^(1/2)*dq3*dqr2*cos(q2)*cos(q5)*sin(q3))/2000000 + (1369*3^(1/2)*dq5*dqr2*cos(q2)*cos(q3)*sin(q4))/4000000 - (259*3^(1/2)*dq5*dqr2*cos(q2)*cos(q3)*sin(q5))/2000000 + (1369*dq1*dqr2*cos(2*q2)*sin(2*q3)*sin(2*q4)*sin(2*q5))/8000000 - (1369*dq1*dqr2*cos(2*q3)*sin(2*q2)*sin(2*q4)*sin(2*q5))/8000000 + dq1*dqr2*cos(2*q2)*cos(q3)*sin(q4)*((18589*3^(1/2))/2000000 + 1073/100000) + (32449*dq1*dqr2*cos(2*q2)*cos(2*q3)*cos(q4)*sin(q5))/4000000 - (1369*dq2*dqr2*cos(2*q4)*sin(2*q5)*cos(q2)*cos(q3))/4000000 - (1369*dq2*dqr2*cos(2*q5)*sin(2*q4)*cos(q2)*cos(q3))/3200000 + (1369*dq3*dqr2*cos(2*q4)*sin(2*q5)*cos(q2)*cos(q3))/4000000 + (1369*dq3*dqr2*cos(2*q5)*sin(2*q4)*cos(q2)*cos(q3))/3200000 + (1369*dq4*dqr2*cos(2*q4)*cos(2*q5)*cos(q2)*sin(q3))/3200000 - (1369*dq4*dqr2*cos(2*q4)*cos(2*q5)*cos(q3)*sin(q2))/3200000 + (1369*dq5*dqr2*cos(2*q4)*cos(2*q5)*cos(q2)*sin(q3))/4000000 - (1369*dq5*dqr2*cos(2*q4)*cos(2*q5)*cos(q3)*sin(q2))/4000000 + dq1*dqr2*sin(2*q2)*sin(q3)*sin(q4)*((18589*3^(1/2))/2000000 + 1073/100000) - dq1*dqr2*cos(2*q2)*cos(2*q4)*sin(2*q3)*((23717*3^(1/2))/40000000 + 1574893/1600000000) + dq1*dqr2*cos(2*q3)*cos(2*q4)*sin(2*q2)*((23717*3^(1/2))/40000000 + 1574893/1600000000) - dq2*dqr2*sin(2*q4)*cos(q2)*cos(q3)*((23717*3^(1/2))/20000000 + 1574893/800000000) + dq3*dqr2*sin(2*q4)*cos(q2)*cos(q3)*((23717*3^(1/2))/20000000 + 1574893/800000000) + dq4*dqr2*cos(2*q4)*cos(q2)*sin(q3)*((23717*3^(1/2))/20000000 + 1574893/800000000) - dq4*dqr2*cos(2*q4)*cos(q3)*sin(q2)*((23717*3^(1/2))/20000000 + 1574893/800000000) + (32449*dq1*dqr2*sin(2*q2)*sin(2*q3)*cos(q4)*sin(q5))/4000000 - (1369*dq4*dqr2*sin(2*q4)*sin(2*q5)*cos(q2)*sin(q3))/4000000 - (1369*dq5*dqr2*sin(2*q4)*sin(2*q5)*cos(q2)*sin(q3))/3200000 + (1369*dq5*dqr2*sin(2*q4)*sin(2*q5)*cos(q3)*sin(q2))/3200000 + (1073*3^(1/2)*dq1*dqr2*cos(2*q2)*cos(q5)*sin(q3))/200000 - (1073*3^(1/2)*dq1*dqr2*sin(2*q2)*cos(q3)*cos(q5))/200000 - (259*dq2*dqr2*cos(q2)*cos(q3)*cos(q4)*sin(q5))/1000000 - (259*dq2*dqr2*cos(q2)*cos(q3)*cos(q5)*sin(q4))/2000000 + (259*dq3*dqr2*cos(q2)*cos(q3)*cos(q4)*sin(q5))/1000000 + (259*dq3*dqr2*cos(q2)*cos(q3)*cos(q5)*sin(q4))/2000000 + (259*dq4*dqr2*cos(q2)*cos(q4)*cos(q5)*sin(q3))/2000000 + (259*dq5*dqr2*cos(q2)*cos(q4)*cos(q5)*sin(q3))/1000000 - dq1*dqr2*cos(2*q2)*sin(2*q3)*cos(q5)*((348207*3^(1/2))/80000000 + 1369/4000000) + dq1*dqr2*cos(2*q3)*sin(2*q2)*cos(q5)*((348207*3^(1/2))/80000000 + 1369/4000000) - dq1*dqr2*cos(2*q2)*cos(2*q3)*sin(q4)*((548467*3^(1/2))/80000000 + 32449/4000000) - (32449*dq2*dqr2*cos(q2)*sin(q3)*sin(q4)*sin(q5))/4000000 + (32449*dq3*dqr2*cos(q2)*sin(q3)*sin(q4)*sin(q5))/4000000 - (259*dq4*dqr2*cos(q2)*sin(q3)*sin(q4)*sin(q5))/1000000 - (259*dq5*dqr2*cos(q2)*sin(q3)*sin(q4)*sin(q5))/2000000 - dq1*dqr2*sin(2*q2)*sin(2*q3)*sin(q4)*((548467*3^(1/2))/80000000 + 32449/4000000) + dq2*dqr2*cos(q2)*cos(q3)*sin(q4)*((4487*3^(1/2))/20000000 + 259/1000000) - dq3*dqr2*cos(q2)*cos(q3)*sin(q4)*((4487*3^(1/2))/20000000 + 259/1000000) - dq4*dqr2*cos(q2)*cos(q4)*sin(q3)*((4487*3^(1/2))/20000000 + 259/1000000) - dq4*dqr2*cos(q2)*cos(q5)*sin(q3)*((23717*3^(1/2))/40000000 + 1369/2000000) - dq5*dqr2*cos(q2)*cos(q5)*sin(q3)*((23717*3^(1/2))/40000000 + 1369/2000000) - dq2*dqr2*cos(q2)*cos(q4)*sin(q3)*((548467*3^(1/2))/80000000 + 32449/4000000) + dq3*dqr2*cos(q2)*cos(q4)*sin(q3)*((548467*3^(1/2))/80000000 + 32449/4000000) - (1073*dq1*dqr2*cos(2*q2)*cos(q3)*cos(q4)*sin(q5))/100000 - (1073*dq1*dqr2*cos(2*q2)*cos(q3)*cos(q5)*sin(q4))/200000 + (1369*3^(1/2)*dq1*dqr2*cos(2*q2)*cos(2*q3)*cos(2*q5)*sin(q4))/8000000 + (1369*3^(1/2)*dq1*dqr2*cos(2*q2)*cos(2*q3)*sin(2*q5)*cos(q4))/4000000 + dq2*dqr2*cos(2*q4)*cos(q2)*cos(q3)*sin(q5)*((23717*3^(1/2))/20000000 + 1369/1000000) - dq3*dqr2*cos(2*q4)*cos(q2)*cos(q3)*sin(q5)*((23717*3^(1/2))/20000000 + 1369/1000000) + dq2*dqr2*sin(2*q4)*cos(q2)*cos(q3)*cos(q5)*((23717*3^(1/2))/40000000 + 1369/2000000) - dq3*dqr2*sin(2*q4)*cos(q2)*cos(q3)*cos(q5)*((23717*3^(1/2))/40000000 + 1369/2000000) - dq4*dqr2*cos(2*q4)*cos(q2)*cos(q5)*sin(q3)*((23717*3^(1/2))/40000000 + 1369/2000000) - dq5*dqr2*cos(2*q4)*cos(q2)*cos(q5)*sin(q3)*((23717*3^(1/2))/40000000 + 1369/2000000) + (1369*3^(1/2)*dq1*dqr2*cos(2*q5)*sin(2*q2)*sin(2*q3)*sin(q4))/8000000 + (1369*3^(1/2)*dq1*dqr2*sin(2*q2)*sin(2*q3)*sin(2*q5)*cos(q4))/4000000 + dq4*dqr2*sin(2*q4)*cos(q2)*sin(q3)*sin(q5)*((23717*3^(1/2))/20000000 + 1369/1000000) + dq5*dqr2*sin(2*q4)*cos(q2)*sin(q3)*sin(q5)*((23717*3^(1/2))/80000000 + 1369/4000000) + (1369*3^(1/2)*dq2*dqr2*cos(2*q5)*cos(q2)*cos(q4)*sin(q3))/8000000 - (1369*3^(1/2)*dq3*dqr2*cos(2*q5)*cos(q2)*cos(q4)*sin(q3))/8000000 - (1369*3^(1/2)*dq5*dqr2*cos(2*q5)*cos(q2)*cos(q3)*sin(q4))/4000000 - (1369*3^(1/2)*dq5*dqr2*sin(2*q5)*cos(q2)*cos(q3)*cos(q4))/8000000 - dq1*dqr2*cos(2*q2)*cos(2*q3)*cos(q5)*sin(q4)*((1369*3^(1/2))/2000000 - 45547/20000000) - (1369*3^(1/2)*dq2*dqr2*sin(2*q5)*cos(q2)*sin(q3)*sin(q4))/4000000 + (1369*3^(1/2)*dq3*dqr2*sin(2*q5)*cos(q2)*sin(q3)*sin(q4))/4000000 - dq1*dqr2*sin(2*q2)*sin(2*q3)*cos(q5)*sin(q4)*((1369*3^(1/2))/2000000 - 45547/20000000) - dq2*dqr2*cos(q2)*cos(q4)*cos(q5)*sin(q3)*((1369*3^(1/2))/2000000 - 45547/20000000) + dq3*dqr2*cos(q2)*cos(q4)*cos(q5)*sin(q3)*((1369*3^(1/2))/2000000 - 45547/20000000) + dq5*dqr2*cos(q2)*cos(q3)*cos(q4)*sin(q5)*((1369*3^(1/2))/2000000 + 71151/40000000) + dq1*dqr2*cos(2*q2)*cos(2*q4)*sin(2*q3)*cos(q5)*((23717*3^(1/2))/80000000 + 1369/4000000) - dq1*dqr2*cos(2*q3)*cos(2*q4)*sin(2*q2)*cos(q5)*((23717*3^(1/2))/80000000 + 1369/4000000) - dq1*dqr2*cos(2*q2)*sin(2*q3)*sin(2*q4)*sin(q5)*((23717*3^(1/2))/40000000 + 1369/2000000) + dq1*dqr2*cos(2*q3)*sin(2*q2)*sin(2*q4)*sin(q5)*((23717*3^(1/2))/40000000 + 1369/2000000);
Y1_5_4=(25433*dq1*dqr3*sin(q3))/800000 - (25433*dq1*dqr3*cos(2*q2)*sin(q3))/800000 - (6139*dq2*dqr3*cos(q2)*sin(q3))/4000000 + (6139*dq2*dqr3*cos(q3)*sin(q2))/4000000 + (6139*dq3*dqr3*cos(q2)*sin(q3))/4000000 - (6139*dq3*dqr3*cos(q3)*sin(q2))/4000000 - (1369*dq5*dqr3*cos(q2)*sin(q3))/4000000 + (1369*dq5*dqr3*cos(q3)*sin(q2))/4000000 + (4107*dq4*dqr3*cos(2*q5)*cos(q2)*sin(q3))/16000000 - (4107*dq4*dqr3*cos(2*q5)*cos(q3)*sin(q2))/16000000 + dq1*dqr2*cos(2*q2)*sin(2*q3)*((23717*3^(1/2))/40000000 - 36744657/1600000000) - dq4*dqr3*cos(q2)*sin(q3)*((23717*3^(1/2))/20000000 + 2122493/800000000) + dq4*dqr3*cos(q3)*sin(q2)*((23717*3^(1/2))/20000000 + 2122493/800000000) + (1073*3^(1/2)*dq1*dqr3*cos(q5)*sin(q3))/400000 + (1073*dq1*dqr3*sin(2*q2)*cos(q4)*sin(q3)*sin(q5))/200000 + (1073*dq1*dqr3*sin(2*q2)*cos(q5)*sin(q3)*sin(q4))/400000 - (259*3^(1/2)*dq2*dqr3*cos(q2)*cos(q5)*sin(q3))/2000000 + (259*3^(1/2)*dq2*dqr3*cos(q3)*cos(q5)*sin(q2))/2000000 + (259*3^(1/2)*dq3*dqr3*cos(q2)*cos(q5)*sin(q3))/2000000 - (259*3^(1/2)*dq3*dqr3*cos(q3)*cos(q5)*sin(q2))/2000000 - (1369*3^(1/2)*dq5*dqr3*sin(q2)*sin(q3)*sin(q4))/4000000 + (259*3^(1/2)*dq5*dqr3*sin(q2)*sin(q3)*sin(q5))/2000000 - (1369*dq4*dqr3*cos(2*q4)*cos(2*q5)*cos(q2)*sin(q3))/3200000 + (1369*dq4*dqr3*cos(2*q4)*cos(2*q5)*cos(q3)*sin(q2))/3200000 - (1369*dq5*dqr3*cos(2*q4)*cos(2*q5)*cos(q2)*sin(q3))/4000000 + (1369*dq5*dqr3*cos(2*q4)*cos(2*q5)*cos(q3)*sin(q2))/4000000 - dq1*dqr3*sin(2*q2)*sin(q3)*sin(q4)*((18589*3^(1/2))/4000000 + 1073/200000) - dq4*dqr3*cos(2*q4)*cos(q2)*sin(q3)*((23717*3^(1/2))/20000000 + 1574893/800000000) + dq4*dqr3*cos(2*q4)*cos(q3)*sin(q2)*((23717*3^(1/2))/20000000 + 1574893/800000000) + (1369*dq2*dqr3*cos(2*q4)*sin(2*q5)*sin(q2)*sin(q3))/4000000 + (1369*dq2*dqr3*cos(2*q5)*sin(2*q4)*sin(q2)*sin(q3))/3200000 - (1369*dq3*dqr3*cos(2*q4)*sin(2*q5)*sin(q2)*sin(q3))/4000000 - (1369*dq3*dqr3*cos(2*q5)*sin(2*q4)*sin(q2)*sin(q3))/3200000 + (1369*dq4*dqr3*sin(2*q4)*sin(2*q5)*cos(q2)*sin(q3))/4000000 - (1369*dq4*dqr3*sin(2*q4)*sin(2*q5)*cos(q3)*sin(q2))/4000000 + (1369*dq5*dqr3*sin(2*q4)*sin(2*q5)*cos(q2)*sin(q3))/3200000 - (1369*dq5*dqr3*sin(2*q4)*sin(2*q5)*cos(q3)*sin(q2))/3200000 - (1073*3^(1/2)*dq1*dqr3*cos(2*q2)*cos(q5)*sin(q3))/400000 + dq2*dqr3*sin(2*q4)*sin(q2)*sin(q3)*((23717*3^(1/2))/20000000 + 1574893/800000000) - dq3*dqr3*sin(2*q4)*sin(q2)*sin(q3)*((23717*3^(1/2))/20000000 + 1574893/800000000) + (259*dq2*dqr3*cos(q2)*cos(q3)*cos(q5)*sin(q4))/2000000 - (259*dq3*dqr3*cos(q2)*cos(q3)*cos(q5)*sin(q4))/2000000 - (259*dq4*dqr3*cos(q2)*cos(q4)*cos(q5)*sin(q3))/2000000 + (259*dq4*dqr3*cos(q3)*cos(q4)*cos(q5)*sin(q2))/2000000 - (259*dq5*dqr3*cos(q2)*cos(q4)*cos(q5)*sin(q3))/1000000 + (259*dq5*dqr3*cos(q3)*cos(q4)*cos(q5)*sin(q2))/1000000 + (32449*dq2*dqr3*cos(q2)*sin(q3)*sin(q4)*sin(q5))/4000000 - (32449*dq2*dqr3*cos(q3)*sin(q2)*sin(q4)*sin(q5))/4000000 + (259*dq2*dqr3*cos(q4)*sin(q2)*sin(q3)*sin(q5))/1000000 + (259*dq2*dqr3*cos(q5)*sin(q2)*sin(q3)*sin(q4))/2000000 - (32449*dq3*dqr3*cos(q2)*sin(q3)*sin(q4)*sin(q5))/4000000 + (32449*dq3*dqr3*cos(q3)*sin(q2)*sin(q4)*sin(q5))/4000000 - (259*dq3*dqr3*cos(q4)*sin(q2)*sin(q3)*sin(q5))/1000000 - (259*dq3*dqr3*cos(q5)*sin(q2)*sin(q3)*sin(q4))/2000000 + (259*dq4*dqr3*cos(q2)*sin(q3)*sin(q4)*sin(q5))/1000000 - (259*dq4*dqr3*cos(q3)*sin(q2)*sin(q4)*sin(q5))/1000000 + (259*dq5*dqr3*cos(q2)*sin(q3)*sin(q4)*sin(q5))/2000000 - (259*dq5*dqr3*cos(q3)*sin(q2)*sin(q4)*sin(q5))/2000000 - dq2*dqr3*cos(q2)*cos(q3)*sin(q4)*((4487*3^(1/2))/20000000 + 259/1000000) + dq3*dqr3*cos(q2)*cos(q3)*sin(q4)*((4487*3^(1/2))/20000000 + 259/1000000) + dq4*dqr3*cos(q2)*cos(q4)*sin(q3)*((4487*3^(1/2))/20000000 + 259/1000000) - dq4*dqr3*cos(q3)*cos(q4)*sin(q2)*((4487*3^(1/2))/20000000 + 259/1000000) + dq4*dqr3*cos(q2)*cos(q5)*sin(q3)*((23717*3^(1/2))/40000000 + 1369/2000000) - dq4*dqr3*cos(q3)*cos(q5)*sin(q2)*((23717*3^(1/2))/40000000 + 1369/2000000) + dq5*dqr3*cos(q2)*cos(q5)*sin(q3)*((23717*3^(1/2))/40000000 + 1369/2000000) - dq5*dqr3*cos(q3)*cos(q5)*sin(q2)*((23717*3^(1/2))/40000000 + 1369/2000000) + dq2*dqr3*cos(q2)*cos(q4)*sin(q3)*((548467*3^(1/2))/80000000 + 32449/4000000) - dq2*dqr3*cos(q3)*cos(q4)*sin(q2)*((548467*3^(1/2))/80000000 + 32449/4000000) - dq3*dqr3*cos(q2)*cos(q4)*sin(q3)*((548467*3^(1/2))/80000000 + 32449/4000000) + dq3*dqr3*cos(q3)*cos(q4)*sin(q2)*((548467*3^(1/2))/80000000 + 32449/4000000) - dq2*dqr3*sin(q2)*sin(q3)*sin(q4)*((4487*3^(1/2))/20000000 + 259/1000000) + dq3*dqr3*sin(q2)*sin(q3)*sin(q4)*((4487*3^(1/2))/20000000 + 259/1000000) + dq4*dqr3*cos(2*q4)*cos(q2)*cos(q5)*sin(q3)*((23717*3^(1/2))/40000000 + 1369/2000000) - dq4*dqr3*cos(2*q4)*cos(q3)*cos(q5)*sin(q2)*((23717*3^(1/2))/40000000 + 1369/2000000) + dq5*dqr3*cos(2*q4)*cos(q2)*cos(q5)*sin(q3)*((23717*3^(1/2))/40000000 + 1369/2000000) - dq5*dqr3*cos(2*q4)*cos(q3)*cos(q5)*sin(q2)*((23717*3^(1/2))/40000000 + 1369/2000000) - dq2*dqr3*cos(2*q4)*sin(q2)*sin(q3)*sin(q5)*((23717*3^(1/2))/20000000 + 1369/1000000) + dq3*dqr3*cos(2*q4)*sin(q2)*sin(q3)*sin(q5)*((23717*3^(1/2))/20000000 + 1369/1000000) - dq4*dqr3*sin(2*q4)*cos(q2)*sin(q3)*sin(q5)*((23717*3^(1/2))/20000000 + 1369/1000000) + dq4*dqr3*sin(2*q4)*cos(q3)*sin(q2)*sin(q5)*((23717*3^(1/2))/20000000 + 1369/1000000) - dq2*dqr3*sin(2*q4)*cos(q5)*sin(q2)*sin(q3)*((23717*3^(1/2))/40000000 + 1369/2000000) + dq3*dqr3*sin(2*q4)*cos(q5)*sin(q2)*sin(q3)*((23717*3^(1/2))/40000000 + 1369/2000000) - dq5*dqr3*sin(2*q4)*cos(q2)*sin(q3)*sin(q5)*((23717*3^(1/2))/80000000 + 1369/4000000) + dq5*dqr3*sin(2*q4)*cos(q3)*sin(q2)*sin(q5)*((23717*3^(1/2))/80000000 + 1369/4000000) - (1369*3^(1/2)*dq2*dqr3*cos(2*q5)*cos(q2)*cos(q4)*sin(q3))/8000000 + (1369*3^(1/2)*dq2*dqr3*cos(2*q5)*cos(q3)*cos(q4)*sin(q2))/8000000 + (1369*3^(1/2)*dq3*dqr3*cos(2*q5)*cos(q2)*cos(q4)*sin(q3))/8000000 - (1369*3^(1/2)*dq3*dqr3*cos(2*q5)*cos(q3)*cos(q4)*sin(q2))/8000000 + (1369*3^(1/2)*dq5*dqr3*cos(2*q5)*cos(q2)*cos(q3)*sin(q4))/4000000 + (1369*3^(1/2)*dq2*dqr3*sin(2*q5)*cos(q2)*sin(q3)*sin(q4))/4000000 - (1369*3^(1/2)*dq2*dqr3*sin(2*q5)*cos(q3)*sin(q2)*sin(q4))/4000000 - (1369*3^(1/2)*dq3*dqr3*sin(2*q5)*cos(q2)*sin(q3)*sin(q4))/4000000 + (1369*3^(1/2)*dq3*dqr3*sin(2*q5)*cos(q3)*sin(q2)*sin(q4))/4000000 + (1369*3^(1/2)*dq5*dqr3*cos(2*q5)*sin(q2)*sin(q3)*sin(q4))/4000000 + (1369*3^(1/2)*dq5*dqr3*sin(2*q5)*cos(q4)*sin(q2)*sin(q3))/8000000 + dq2*dqr3*cos(q2)*cos(q4)*cos(q5)*sin(q3)*((1369*3^(1/2))/2000000 - 45547/20000000) - dq2*dqr3*cos(q3)*cos(q4)*cos(q5)*sin(q2)*((1369*3^(1/2))/2000000 - 45547/20000000) - dq3*dqr3*cos(q2)*cos(q4)*cos(q5)*sin(q3)*((1369*3^(1/2))/2000000 - 45547/20000000) + dq3*dqr3*cos(q3)*cos(q4)*cos(q5)*sin(q2)*((1369*3^(1/2))/2000000 - 45547/20000000) - dq5*dqr3*cos(q4)*sin(q2)*sin(q3)*sin(q5)*((1369*3^(1/2))/2000000 + 71151/40000000);
Y1_5_5=(25433*dq1*dqr3*sin(2*q2)*cos(q3))/800000 + (4107*dq2*dqr4*cos(2*q5)*cos(q3)*sin(q2))/16000000 - (4107*dq3*dqr4*cos(2*q5)*cos(q3)*sin(q2))/16000000 - dq1*dqr3*cos(2*q2)*sin(2*q3)*((23717*3^(1/2))/40000000 - 36744657/1600000000) + dq1*dqr3*cos(2*q3)*sin(2*q2)*((23717*3^(1/2))/40000000 - 36744657/1600000000) - dq2*dqr4*cos(q3)*sin(q2)*((23717*3^(1/2))/20000000 + 2122493/800000000) + dq3*dqr4*cos(q3)*sin(q2)*((23717*3^(1/2))/20000000 + 2122493/800000000) + (4107*dq5*dqr4*sin(2*q5)*sin(q2)*sin(q3))/8000000 - (1073*dq1*dqr3*cos(q3)*cos(q4)*sin(q5))/200000 - (1073*dq1*dqr3*cos(q3)*cos(q5)*sin(q4))/400000 - (1073*dq4*dqr4*cos(q4)*cos(q5)*sin(q2))/200000 - (1073*dq5*dqr4*cos(q4)*cos(q5)*sin(q2))/100000 + (12321*dq1*dqr3*cos(2*q2)*cos(2*q5)*sin(2*q3))/32000000 - (12321*dq1*dqr3*cos(2*q3)*cos(2*q5)*sin(2*q2))/32000000 + (1073*dq1*dqr4*sin(q3)*sin(q4)*sin(q5))/200000 + (1073*dq4*dqr4*sin(q2)*sin(q4)*sin(q5))/100000 + (1073*dq5*dqr4*sin(q2)*sin(q4)*sin(q5))/200000 + dq4*dqr4*cos(q4)*sin(q2)*((18589*3^(1/2))/2000000 + 1073/100000) + dq1*dqr3*cos(q3)*sin(q4)*((18589*3^(1/2))/4000000 + 1073/200000) + (1369*dq1*dqr3*cos(2*q2)*cos(2*q4)*cos(2*q5)*sin(2*q3))/6400000 - (1369*dq1*dqr3*cos(2*q3)*cos(2*q4)*cos(2*q5)*sin(2*q2))/6400000 - (1073*dq1*dqr4*cos(2*q2)*sin(q3)*sin(q4)*sin(q5))/200000 - (1369*3^(1/2)*dq5*dqr3*cos(q2)*cos(q3)*sin(q4))/4000000 + (259*3^(1/2)*dq5*dqr3*cos(q2)*cos(q3)*sin(q5))/2000000 + (1369*3^(1/2)*dq5*dqr4*cos(q3)*cos(q4)*sin(q2))/4000000 - (1369*dq1*dqr3*cos(2*q2)*sin(2*q3)*sin(2*q4)*sin(2*q5))/8000000 + (1369*dq1*dqr3*cos(2*q3)*sin(2*q2)*sin(2*q4)*sin(2*q5))/8000000 - dq1*dqr3*cos(2*q2)*cos(q3)*sin(q4)*((18589*3^(1/2))/4000000 + 1073/200000) - (32449*dq1*dqr3*cos(2*q2)*cos(2*q3)*cos(q4)*sin(q5))/4000000 + (1369*dq2*dqr3*cos(2*q4)*sin(2*q5)*cos(q2)*cos(q3))/4000000 + (1369*dq2*dqr3*cos(2*q5)*sin(2*q4)*cos(q2)*cos(q3))/3200000 - (1369*dq2*dqr4*cos(2*q4)*cos(2*q5)*cos(q3)*sin(q2))/3200000 - (1369*dq3*dqr3*cos(2*q4)*sin(2*q5)*cos(q2)*cos(q3))/4000000 - (1369*dq3*dqr3*cos(2*q5)*sin(2*q4)*cos(q2)*cos(q3))/3200000 + (1369*dq3*dqr4*cos(2*q4)*cos(2*q5)*cos(q3)*sin(q2))/3200000 + dq1*dqr3*cos(2*q2)*cos(2*q4)*sin(2*q3)*((23717*3^(1/2))/40000000 + 1574893/1600000000) - dq1*dqr3*cos(2*q3)*cos(2*q4)*sin(2*q2)*((23717*3^(1/2))/40000000 + 1574893/1600000000) + dq2*dqr3*sin(2*q4)*cos(q2)*cos(q3)*((23717*3^(1/2))/20000000 + 1574893/800000000) - dq2*dqr4*cos(2*q4)*cos(q3)*sin(q2)*((23717*3^(1/2))/20000000 + 1574893/800000000) - dq3*dqr3*sin(2*q4)*cos(q2)*cos(q3)*((23717*3^(1/2))/20000000 + 1574893/800000000) + dq3*dqr4*cos(2*q4)*cos(q3)*sin(q2)*((23717*3^(1/2))/20000000 + 1574893/800000000) - (32449*dq1*dqr3*sin(2*q2)*sin(2*q3)*cos(q4)*sin(q5))/4000000 + (1369*dq2*dqr4*sin(2*q4)*sin(2*q5)*cos(q3)*sin(q2))/4000000 - (1369*dq3*dqr4*sin(2*q4)*sin(2*q5)*cos(q3)*sin(q2))/4000000 + (1073*3^(1/2)*dq1*dqr3*sin(2*q2)*cos(q3)*cos(q5))/400000 + (259*dq2*dqr3*cos(q2)*cos(q3)*cos(q4)*sin(q5))/1000000 - (259*dq2*dqr4*cos(q3)*cos(q4)*cos(q5)*sin(q2))/2000000 - (259*dq3*dqr3*cos(q2)*cos(q3)*cos(q4)*sin(q5))/1000000 + (259*dq3*dqr4*cos(q3)*cos(q4)*cos(q5)*sin(q2))/2000000 + (32449*dq5*dqr4*cos(q3)*cos(q4)*cos(q5)*sin(q2))/4000000 + dq1*dqr3*cos(2*q2)*sin(2*q3)*cos(q5)*((348207*3^(1/2))/80000000 + 1369/4000000) - dq1*dqr3*cos(2*q3)*sin(2*q2)*cos(q5)*((348207*3^(1/2))/80000000 + 1369/4000000) + dq1*dqr3*cos(2*q2)*cos(2*q3)*sin(q4)*((548467*3^(1/2))/80000000 + 32449/4000000) - (259*dq2*dqr4*cos(q2)*sin(q3)*sin(q4)*sin(q5))/1000000 + (259*dq2*dqr4*cos(q3)*sin(q2)*sin(q4)*sin(q5))/1000000 + (259*dq3*dqr4*cos(q2)*sin(q3)*sin(q4)*sin(q5))/1000000 - (259*dq3*dqr4*cos(q3)*sin(q2)*sin(q4)*sin(q5))/1000000 + (32449*dq4*dqr4*cos(q2)*sin(q3)*sin(q4)*sin(q5))/4000000 - (32449*dq4*dqr4*cos(q3)*sin(q2)*sin(q4)*sin(q5))/4000000 - (259*dq4*dqr4*cos(q4)*sin(q2)*sin(q3)*sin(q5))/1000000 - (259*dq4*dqr4*cos(q5)*sin(q2)*sin(q3)*sin(q4))/2000000 + (32449*dq5*dqr4*cos(q2)*sin(q3)*sin(q4)*sin(q5))/8000000 - (32449*dq5*dqr4*cos(q3)*sin(q2)*sin(q4)*sin(q5))/8000000 - (259*dq5*dqr4*cos(q4)*sin(q2)*sin(q3)*sin(q5))/2000000 - (259*dq5*dqr4*cos(q5)*sin(q2)*sin(q3)*sin(q4))/1000000 + dq1*dqr3*sin(2*q2)*sin(2*q3)*sin(q4)*((548467*3^(1/2))/80000000 + 32449/4000000) + dq2*dqr4*cos(q3)*cos(q4)*sin(q2)*((4487*3^(1/2))/20000000 + 259/1000000) - dq3*dqr4*cos(q3)*cos(q4)*sin(q2)*((4487*3^(1/2))/20000000 + 259/1000000) + dq2*dqr4*cos(q3)*cos(q5)*sin(q2)*((23717*3^(1/2))/40000000 + 1369/2000000) - dq3*dqr4*cos(q3)*cos(q5)*sin(q2)*((23717*3^(1/2))/40000000 + 1369/2000000) - dq4*dqr4*cos(q3)*cos(q4)*sin(q2)*((548467*3^(1/2))/80000000 + 32449/4000000) + (1073*dq1*dqr3*cos(2*q2)*cos(q3)*cos(q4)*sin(q5))/200000 + (1073*dq1*dqr3*cos(2*q2)*cos(q3)*cos(q5)*sin(q4))/400000 + dq4*dqr4*sin(q2)*sin(q3)*sin(q4)*((4487*3^(1/2))/20000000 + 259/1000000) + dq5*dqr4*sin(q2)*sin(q3)*sin(q5)*((23717*3^(1/2))/40000000 + 1369/2000000) - (1369*3^(1/2)*dq1*dqr3*cos(2*q2)*cos(2*q3)*cos(2*q5)*sin(q4))/8000000 - (1369*3^(1/2)*dq1*dqr3*cos(2*q2)*cos(2*q3)*sin(2*q5)*cos(q4))/4000000 - dq2*dqr3*cos(2*q4)*cos(q2)*cos(q3)*sin(q5)*((23717*3^(1/2))/20000000 + 1369/1000000) + dq3*dqr3*cos(2*q4)*cos(q2)*cos(q3)*sin(q5)*((23717*3^(1/2))/20000000 + 1369/1000000) - dq2*dqr3*sin(2*q4)*cos(q2)*cos(q3)*cos(q5)*((23717*3^(1/2))/40000000 + 1369/2000000) + dq2*dqr4*cos(2*q4)*cos(q3)*cos(q5)*sin(q2)*((23717*3^(1/2))/40000000 + 1369/2000000) + dq3*dqr3*sin(2*q4)*cos(q2)*cos(q3)*cos(q5)*((23717*3^(1/2))/40000000 + 1369/2000000) - dq3*dqr4*cos(2*q4)*cos(q3)*cos(q5)*sin(q2)*((23717*3^(1/2))/40000000 + 1369/2000000) - (1369*3^(1/2)*dq1*dqr3*cos(2*q5)*sin(2*q2)*sin(2*q3)*sin(q4))/8000000 - (1369*3^(1/2)*dq1*dqr3*sin(2*q2)*sin(2*q3)*sin(2*q5)*cos(q4))/4000000 - dq2*dqr4*sin(2*q4)*cos(q3)*sin(q2)*sin(q5)*((23717*3^(1/2))/20000000 + 1369/1000000) + dq3*dqr4*sin(2*q4)*cos(q3)*sin(q2)*sin(q5)*((23717*3^(1/2))/20000000 + 1369/1000000) + (1369*3^(1/2)*dq4*dqr4*cos(2*q5)*cos(q3)*cos(q4)*sin(q2))/8000000 + (1369*3^(1/2)*dq5*dqr3*sin(2*q5)*cos(q2)*cos(q3)*cos(q4))/8000000 + (1369*3^(1/2)*dq5*dqr4*cos(2*q5)*cos(q3)*cos(q4)*sin(q2))/4000000 + dq1*dqr3*cos(2*q2)*cos(2*q3)*cos(q5)*sin(q4)*((1369*3^(1/2))/2000000 - 45547/20000000) - (1369*3^(1/2)*dq4*dqr4*sin(2*q5)*cos(q3)*sin(q2)*sin(q4))/4000000 - (1369*3^(1/2)*dq5*dqr4*sin(2*q5)*cos(q3)*sin(q2)*sin(q4))/8000000 + dq1*dqr3*sin(2*q2)*sin(2*q3)*cos(q5)*sin(q4)*((1369*3^(1/2))/2000000 - 45547/20000000) - dq4*dqr4*cos(q3)*cos(q4)*cos(q5)*sin(q2)*((1369*3^(1/2))/2000000 - 45547/20000000) - dq5*dqr3*cos(q2)*cos(q3)*cos(q4)*sin(q5)*((1369*3^(1/2))/2000000 + 71151/40000000) - dq1*dqr3*cos(2*q2)*cos(2*q4)*sin(2*q3)*cos(q5)*((23717*3^(1/2))/80000000 + 1369/4000000) + dq1*dqr3*cos(2*q3)*cos(2*q4)*sin(2*q2)*cos(q5)*((23717*3^(1/2))/80000000 + 1369/4000000) + dq1*dqr3*cos(2*q2)*sin(2*q3)*sin(2*q4)*sin(q5)*((23717*3^(1/2))/40000000 + 1369/2000000) - dq1*dqr3*cos(2*q3)*sin(2*q2)*sin(2*q4)*sin(q5)*((23717*3^(1/2))/40000000 + 1369/2000000);
Y1_5_6=dq1*dqr4*sin(q4)*((4487*3^(1/2))/20000000 + 259/1000000) - (1369*dq1*dqr4*cos(2*q4)*sin(2*q5))/8000000 - (1369*dq1*dqr4*cos(2*q5)*sin(2*q4))/6400000 - (259*dq1*dqr4*cos(q4)*sin(q5))/1000000 - (259*dq1*dqr4*cos(q5)*sin(q4))/2000000 - dq1*dqr4*sin(2*q4)*((23717*3^(1/2))/40000000 + 1574893/1600000000) - (4107*dq2*dqr4*cos(2*q5)*cos(q2)*sin(q3))/16000000 + (4107*dq3*dqr4*cos(2*q5)*cos(q2)*sin(q3))/16000000 + (4107*dq5*dqr4*sin(2*q5)*cos(q2)*cos(q3))/8000000 + dq2*dqr4*cos(q2)*sin(q3)*((23717*3^(1/2))/20000000 + 2122493/800000000) - dq3*dqr4*cos(q2)*sin(q3)*((23717*3^(1/2))/20000000 + 2122493/800000000) + (4107*dq4*dqr5*sin(2*q5)*sin(q2)*sin(q3))/8000000 + dq1*dqr4*cos(2*q4)*sin(q5)*((23717*3^(1/2))/40000000 + 1369/2000000) + dq1*dqr4*sin(2*q4)*cos(q5)*((23717*3^(1/2))/80000000 + 1369/4000000) - (1073*dq1*dqr4*cos(q4)*cos(q5)*sin(q3))/400000 + (1073*dq4*dqr5*sin(q2)*sin(q4)*sin(q5))/200000 + (1073*dq5*dqr5*sin(q2)*sin(q4)*sin(q5))/100000 + dq1*dqr4*cos(q4)*sin(q3)*((18589*3^(1/2))/4000000 + 1073/200000) + (1369*dq1*dqr4*cos(2*q2)*cos(2*q3)*cos(2*q4)*sin(2*q5))/8000000 + (1369*dq1*dqr4*cos(2*q2)*cos(2*q3)*cos(2*q5)*sin(2*q4))/6400000 + (1073*dq1*dqr4*sin(2*q2)*cos(q3)*sin(q4)*sin(q5))/200000 - (1369*3^(1/2)*dq5*dqr4*cos(q2)*cos(q4)*sin(q3))/4000000 + (1369*dq1*dqr4*cos(2*q4)*sin(2*q2)*sin(2*q3)*sin(2*q5))/8000000 + (1369*dq1*dqr4*cos(2*q5)*sin(2*q2)*sin(2*q3)*sin(2*q4))/6400000 - dq1*dqr4*cos(2*q2)*cos(q4)*sin(q3)*((18589*3^(1/2))/4000000 + 1073/200000) + dq1*dqr4*sin(2*q2)*cos(q3)*cos(q4)*((18589*3^(1/2))/4000000 + 1073/200000) + (1369*3^(1/2)*dq2*dqr5*sin(q2)*sin(q3)*sin(q4))/4000000 - (259*3^(1/2)*dq2*dqr5*sin(q2)*sin(q3)*sin(q5))/2000000 - (1369*3^(1/2)*dq3*dqr5*sin(q2)*sin(q3)*sin(q4))/4000000 + (259*3^(1/2)*dq3*dqr5*sin(q2)*sin(q3)*sin(q5))/2000000 + (1369*dq2*dqr4*cos(2*q4)*cos(2*q5)*cos(q2)*sin(q3))/3200000 - (1369*dq3*dqr4*cos(2*q4)*cos(2*q5)*cos(q2)*sin(q3))/3200000 + dq1*dqr4*cos(2*q2)*cos(2*q3)*sin(2*q4)*((23717*3^(1/2))/40000000 + 1574893/1600000000) + dq2*dqr4*cos(2*q4)*cos(q2)*sin(q3)*((23717*3^(1/2))/20000000 + 1574893/800000000) - dq3*dqr4*cos(2*q4)*cos(q2)*sin(q3)*((23717*3^(1/2))/20000000 + 1574893/800000000) + (32449*dq1*dqr4*cos(2*q2)*sin(2*q3)*sin(q4)*sin(q5))/8000000 - (32449*dq1*dqr4*cos(2*q3)*sin(2*q2)*sin(q4)*sin(q5))/8000000 - (1369*dq2*dqr4*sin(2*q4)*sin(2*q5)*cos(q2)*sin(q3))/4000000 + (1369*dq3*dqr4*sin(2*q4)*sin(2*q5)*cos(q2)*sin(q3))/4000000 + dq1*dqr4*sin(2*q2)*sin(2*q3)*sin(2*q4)*((23717*3^(1/2))/40000000 + 1574893/1600000000) + (259*dq2*dqr4*cos(q2)*cos(q4)*cos(q5)*sin(q3))/2000000 - (259*dq2*dqr5*cos(q3)*cos(q4)*cos(q5)*sin(q2))/1000000 - (259*dq3*dqr4*cos(q2)*cos(q4)*cos(q5)*sin(q3))/2000000 + (259*dq3*dqr5*cos(q3)*cos(q4)*cos(q5)*sin(q2))/1000000 - (259*dq4*dqr4*cos(q2)*cos(q3)*cos(q4)*sin(q5))/1000000 - (259*dq4*dqr4*cos(q2)*cos(q3)*cos(q5)*sin(q4))/2000000 + (32449*dq4*dqr5*cos(q3)*cos(q4)*cos(q5)*sin(q2))/4000000 - (259*dq5*dqr4*cos(q2)*cos(q3)*cos(q4)*sin(q5))/2000000 - (259*dq5*dqr4*cos(q2)*cos(q3)*cos(q5)*sin(q4))/1000000 - (32449*dq5*dqr4*cos(q2)*cos(q4)*cos(q5)*sin(q3))/4000000 + dq1*dqr4*cos(2*q2)*sin(2*q3)*cos(q4)*((548467*3^(1/2))/160000000 + 32449/8000000) - dq1*dqr4*cos(2*q3)*sin(2*q2)*cos(q4)*((548467*3^(1/2))/160000000 + 32449/8000000) + (259*dq2*dqr5*cos(q3)*sin(q2)*sin(q4)*sin(q5))/2000000 - (259*dq3*dqr5*cos(q3)*sin(q2)*sin(q4)*sin(q5))/2000000 - (32449*dq4*dqr5*cos(q3)*sin(q2)*sin(q4)*sin(q5))/8000000 - (259*dq4*dqr5*cos(q4)*sin(q2)*sin(q3)*sin(q5))/2000000 - (259*dq4*dqr5*cos(q5)*sin(q2)*sin(q3)*sin(q4))/1000000 - (32449*dq5*dqr5*cos(q3)*sin(q2)*sin(q4)*sin(q5))/4000000 - (259*dq5*dqr5*cos(q4)*sin(q2)*sin(q3)*sin(q5))/1000000 - (259*dq5*dqr5*cos(q5)*sin(q2)*sin(q3)*sin(q4))/2000000 - dq2*dqr4*cos(q2)*cos(q4)*sin(q3)*((4487*3^(1/2))/20000000 + 259/1000000) + dq3*dqr4*cos(q2)*cos(q4)*sin(q3)*((4487*3^(1/2))/20000000 + 259/1000000) + dq4*dqr4*cos(q2)*cos(q3)*sin(q4)*((4487*3^(1/2))/20000000 + 259/1000000) - dq2*dqr4*cos(q2)*cos(q5)*sin(q3)*((23717*3^(1/2))/40000000 + 1369/2000000) + dq3*dqr4*cos(q2)*cos(q5)*sin(q3)*((23717*3^(1/2))/40000000 + 1369/2000000) + dq5*dqr4*cos(q2)*cos(q3)*sin(q5)*((23717*3^(1/2))/40000000 + 1369/2000000) + dq4*dqr4*cos(q2)*cos(q4)*sin(q3)*((548467*3^(1/2))/80000000 + 32449/4000000) + (1073*dq1*dqr4*cos(2*q2)*cos(q4)*cos(q5)*sin(q3))/400000 - (1073*dq1*dqr4*sin(2*q2)*cos(q3)*cos(q4)*cos(q5))/400000 + dq5*dqr5*sin(q2)*sin(q3)*sin(q5)*((23717*3^(1/2))/20000000 + 1369/1000000) + dq4*dqr5*sin(q2)*sin(q3)*sin(q5)*((23717*3^(1/2))/40000000 + 1369/2000000) - (1369*3^(1/2)*dq1*dqr4*cos(2*q2)*cos(2*q5)*sin(2*q3)*cos(q4))/16000000 + (1369*3^(1/2)*dq1*dqr4*cos(2*q3)*cos(2*q5)*sin(2*q2)*cos(q4))/16000000 - dq2*dqr4*cos(2*q4)*cos(q2)*cos(q5)*sin(q3)*((23717*3^(1/2))/40000000 + 1369/2000000) + dq3*dqr4*cos(2*q4)*cos(q2)*cos(q5)*sin(q3)*((23717*3^(1/2))/40000000 + 1369/2000000) + (1369*3^(1/2)*dq1*dqr4*cos(2*q2)*sin(2*q3)*sin(2*q5)*sin(q4))/8000000 - (1369*3^(1/2)*dq1*dqr4*cos(2*q3)*sin(2*q2)*sin(2*q5)*sin(q4))/8000000 + dq2*dqr4*sin(2*q4)*cos(q2)*sin(q3)*sin(q5)*((23717*3^(1/2))/20000000 + 1369/1000000) - dq3*dqr4*sin(2*q4)*cos(q2)*sin(q3)*sin(q5)*((23717*3^(1/2))/20000000 + 1369/1000000) - dq2*dqr5*sin(2*q4)*cos(q3)*sin(q2)*sin(q5)*((23717*3^(1/2))/80000000 + 1369/4000000) + dq3*dqr5*sin(2*q4)*cos(q3)*sin(q2)*sin(q5)*((23717*3^(1/2))/80000000 + 1369/4000000) - (1369*3^(1/2)*dq4*dqr4*cos(2*q5)*cos(q2)*cos(q4)*sin(q3))/8000000 - (1369*3^(1/2)*dq5*dqr4*cos(2*q5)*cos(q2)*cos(q4)*sin(q3))/4000000 - (1369*3^(1/2)*dq2*dqr5*cos(2*q5)*sin(q2)*sin(q3)*sin(q4))/4000000 - (1369*3^(1/2)*dq2*dqr5*sin(2*q5)*cos(q4)*sin(q2)*sin(q3))/8000000 + (1369*3^(1/2)*dq3*dqr5*cos(2*q5)*sin(q2)*sin(q3)*sin(q4))/4000000 + (1369*3^(1/2)*dq3*dqr5*sin(2*q5)*cos(q4)*sin(q2)*sin(q3))/8000000 + (1369*3^(1/2)*dq4*dqr4*sin(2*q5)*cos(q2)*sin(q3)*sin(q4))/4000000 - (1369*3^(1/2)*dq4*dqr5*sin(2*q5)*cos(q3)*sin(q2)*sin(q4))/8000000 + (1369*3^(1/2)*dq5*dqr4*sin(2*q5)*cos(q2)*sin(q3)*sin(q4))/8000000 + dq1*dqr4*cos(2*q2)*sin(2*q3)*cos(q4)*cos(q5)*((1369*3^(1/2))/4000000 - 45547/40000000) - dq1*dqr4*cos(2*q3)*sin(2*q2)*cos(q4)*cos(q5)*((1369*3^(1/2))/4000000 - 45547/40000000) + dq5*dqr5*cos(q3)*cos(q4)*cos(q5)*sin(q2)*((1369*3^(1/2))/2000000 + 58349/10000000) + dq4*dqr4*cos(q2)*cos(q4)*cos(q5)*sin(q3)*((1369*3^(1/2))/2000000 - 45547/20000000) - dq1*dqr4*cos(2*q2)*cos(2*q3)*cos(2*q4)*sin(q5)*((23717*3^(1/2))/40000000 + 1369/2000000) + dq2*dqr5*cos(q4)*sin(q2)*sin(q3)*sin(q5)*((1369*3^(1/2))/2000000 + 71151/40000000) - dq3*dqr5*cos(q4)*sin(q2)*sin(q3)*sin(q5)*((1369*3^(1/2))/2000000 + 71151/40000000) - dq1*dqr4*cos(2*q2)*cos(2*q3)*sin(2*q4)*cos(q5)*((23717*3^(1/2))/80000000 + 1369/4000000) - dq1*dqr4*cos(2*q4)*sin(2*q2)*sin(2*q3)*sin(q5)*((23717*3^(1/2))/40000000 + 1369/2000000) - dq1*dqr4*sin(2*q2)*sin(2*q3)*sin(2*q4)*cos(q5)*((23717*3^(1/2))/80000000 + 1369/4000000);
Y1_5_7=(4107*dq1*dqr5*sin(2*q5))/32000000 - dq1*dqr5*sin(q5)*((253339*3^(1/2))/160000000 - 4107/8000000) - (1369*dq1*dqr5*cos(2*q4)*sin(2*q5))/6400000 - (1369*dq1*dqr5*cos(2*q5)*sin(2*q4))/8000000 + (1369*dq2*dqr5*cos(q2)*sin(q3))/4000000 - (1369*dq2*dqr5*cos(q3)*sin(q2))/4000000 - (1369*dq3*dqr5*cos(q2)*sin(q3))/4000000 + (1369*dq3*dqr5*cos(q3)*sin(q2))/4000000 - (259*dq1*dqr5*cos(q4)*sin(q5))/2000000 - (259*dq1*dqr5*cos(q5)*sin(q4))/1000000 + (4107*dq4*dqr5*sin(2*q5)*cos(q2)*cos(q3))/8000000 + (1073*3^(1/2)*dq1*dqr5*cos(q3)*sin(q5))/400000 - (32449*ddqr2*sin(q2)*sin(q3)*sin(q4)*sin(q5))/4000000 + (32449*ddqr3*sin(q2)*sin(q3)*sin(q4)*sin(q5))/4000000 - (259*ddqr4*sin(q2)*sin(q3)*sin(q4)*sin(q5))/1000000 - (259*ddqr5*sin(q2)*sin(q3)*sin(q4)*sin(q5))/2000000 + dq1*dqr5*sin(2*q4)*cos(q5)*((23717*3^(1/2))/80000000 + 1369/4000000) + dq1*dqr5*cos(2*q4)*sin(q5)*((23717*3^(1/2))/160000000 + 1369/8000000) - (1073*dq1*dqr5*cos(q4)*cos(q5)*sin(q3))/200000 - (1073*dq4*dqr5*cos(q4)*cos(q5)*sin(q2))/100000 - (1073*dq5*dqr5*cos(q4)*cos(q5)*sin(q2))/200000 + (12321*dq1*dqr5*cos(2*q2)*cos(2*q3)*sin(2*q5))/32000000 + (1073*dq1*dqr5*sin(q3)*sin(q4)*sin(q5))/400000 + (12321*dq1*dqr5*sin(2*q2)*sin(2*q3)*sin(2*q5))/32000000 + (1369*dq1*dqr5*cos(2*q2)*cos(2*q3)*cos(2*q4)*sin(2*q5))/6400000 + (1369*dq1*dqr5*cos(2*q2)*cos(2*q3)*cos(2*q5)*sin(2*q4))/8000000 - (1073*dq1*dqr5*cos(2*q2)*sin(q3)*sin(q4)*sin(q5))/400000 + (1073*dq1*dqr5*sin(2*q2)*cos(q3)*sin(q4)*sin(q5))/400000 - (1369*3^(1/2)*ddqr2*sin(2*q5)*sin(q2)*sin(q3)*sin(q4))/4000000 + (1369*3^(1/2)*ddqr3*sin(2*q5)*sin(q2)*sin(q3)*sin(q4))/4000000 + (1369*3^(1/2)*dq2*dqr5*cos(q2)*cos(q3)*sin(q4))/4000000 - (259*3^(1/2)*dq2*dqr5*cos(q2)*cos(q3)*sin(q5))/2000000 - (1369*3^(1/2)*dq3*dqr5*cos(q2)*cos(q3)*sin(q4))/4000000 + (259*3^(1/2)*dq3*dqr5*cos(q2)*cos(q3)*sin(q5))/2000000 - (1369*3^(1/2)*dq4*dqr5*cos(q2)*cos(q4)*sin(q3))/4000000 + (1369*3^(1/2)*dq4*dqr5*cos(q3)*cos(q4)*sin(q2))/4000000 + (259*3^(1/2)*dq5*dqr5*cos(q2)*cos(q5)*sin(q3))/2000000 - (259*3^(1/2)*dq5*dqr5*cos(q3)*cos(q5)*sin(q2))/2000000 + (1369*dq1*dqr5*cos(2*q4)*sin(2*q2)*sin(2*q3)*sin(2*q5))/6400000 + (1369*dq1*dqr5*cos(2*q5)*sin(2*q2)*sin(2*q3)*sin(2*q4))/8000000 - (32449*dq1*dqr5*cos(2*q2)*sin(2*q3)*cos(q4)*cos(q5))/8000000 + (32449*dq1*dqr5*cos(2*q3)*sin(2*q2)*cos(q4)*cos(q5))/8000000 + (1369*dq2*dqr5*cos(2*q4)*cos(2*q5)*cos(q2)*sin(q3))/4000000 - (1369*dq2*dqr5*cos(2*q4)*cos(2*q5)*cos(q3)*sin(q2))/4000000 - (1369*dq3*dqr5*cos(2*q4)*cos(2*q5)*cos(q2)*sin(q3))/4000000 + (1369*dq3*dqr5*cos(2*q4)*cos(2*q5)*cos(q3)*sin(q2))/4000000 - ddqr2*cos(q4)*cos(q5)*sin(q2)*sin(q3)*((1369*3^(1/2))/2000000 - 45547/20000000) - (1369*dq2*dqr5*sin(2*q4)*sin(2*q5)*cos(q2)*sin(q3))/3200000 + (1369*dq2*dqr5*sin(2*q4)*sin(2*q5)*cos(q3)*sin(q2))/3200000 + (1369*dq3*dqr5*sin(2*q4)*sin(2*q5)*cos(q2)*sin(q3))/3200000 - (1369*dq3*dqr5*sin(2*q4)*sin(2*q5)*cos(q3)*sin(q2))/3200000 - (1073*3^(1/2)*dq1*dqr5*cos(2*q2)*cos(q3)*sin(q5))/400000 + (259*dq2*dqr5*cos(q2)*cos(q4)*cos(q5)*sin(q3))/1000000 - (259*dq3*dqr5*cos(q2)*cos(q4)*cos(q5)*sin(q3))/1000000 - (259*dq4*dqr5*cos(q2)*cos(q3)*cos(q4)*sin(q5))/2000000 - (259*dq4*dqr5*cos(q2)*cos(q3)*cos(q5)*sin(q4))/1000000 - (32449*dq4*dqr5*cos(q2)*cos(q4)*cos(q5)*sin(q3))/4000000 - (259*dq5*dqr5*cos(q2)*cos(q3)*cos(q4)*sin(q5))/1000000 - (259*dq5*dqr5*cos(q2)*cos(q3)*cos(q5)*sin(q4))/2000000 - (1073*3^(1/2)*dq1*dqr5*sin(2*q2)*sin(q3)*sin(q5))/400000 + dq1*dqr5*cos(2*q2)*cos(2*q3)*sin(q5)*((348207*3^(1/2))/160000000 + 1369/8000000) - (259*dq2*dqr5*cos(q2)*sin(q3)*sin(q4)*sin(q5))/2000000 + (259*dq3*dqr5*cos(q2)*sin(q3)*sin(q4)*sin(q5))/2000000 + (32449*dq4*dqr5*cos(q2)*sin(q3)*sin(q4)*sin(q5))/8000000 + (32449*dq5*dqr5*cos(q2)*sin(q3)*sin(q4)*sin(q5))/4000000 + dq1*dqr5*sin(2*q2)*sin(2*q3)*sin(q5)*((348207*3^(1/2))/160000000 + 1369/8000000) + dq5*dqr5*cos(q2)*cos(q3)*sin(q5)*((23717*3^(1/2))/20000000 + 1369/1000000) - dq2*dqr5*cos(q2)*cos(q5)*sin(q3)*((23717*3^(1/2))/40000000 + 1369/2000000) + dq2*dqr5*cos(q3)*cos(q5)*sin(q2)*((23717*3^(1/2))/40000000 + 1369/2000000) + dq3*dqr5*cos(q2)*cos(q5)*sin(q3)*((23717*3^(1/2))/40000000 + 1369/2000000) - dq3*dqr5*cos(q3)*cos(q5)*sin(q2)*((23717*3^(1/2))/40000000 + 1369/2000000) + dq4*dqr5*cos(q2)*cos(q3)*sin(q5)*((23717*3^(1/2))/40000000 + 1369/2000000) + (1073*dq1*dqr5*cos(2*q2)*cos(q4)*cos(q5)*sin(q3))/200000 - (1073*dq1*dqr5*sin(2*q2)*cos(q3)*cos(q4)*cos(q5))/200000 - (1369*3^(1/2)*dq1*dqr5*cos(2*q2)*cos(2*q5)*sin(2*q3)*cos(q4))/4000000 + (1369*3^(1/2)*dq1*dqr5*cos(2*q3)*cos(2*q5)*sin(2*q2)*cos(q4))/4000000 - dq2*dqr5*cos(2*q4)*cos(q2)*cos(q5)*sin(q3)*((23717*3^(1/2))/40000000 + 1369/2000000) + dq2*dqr5*cos(2*q4)*cos(q3)*cos(q5)*sin(q2)*((23717*3^(1/2))/40000000 + 1369/2000000) + dq3*dqr5*cos(2*q4)*cos(q2)*cos(q5)*sin(q3)*((23717*3^(1/2))/40000000 + 1369/2000000) - dq3*dqr5*cos(2*q4)*cos(q3)*cos(q5)*sin(q2)*((23717*3^(1/2))/40000000 + 1369/2000000) + (1369*3^(1/2)*dq1*dqr5*cos(2*q2)*sin(2*q3)*sin(2*q5)*sin(q4))/8000000 - (1369*3^(1/2)*dq1*dqr5*cos(2*q3)*sin(2*q2)*sin(2*q5)*sin(q4))/8000000 + dq2*dqr5*sin(2*q4)*cos(q2)*sin(q3)*sin(q5)*((23717*3^(1/2))/80000000 + 1369/4000000) - dq3*dqr5*sin(2*q4)*cos(q2)*sin(q3)*sin(q5)*((23717*3^(1/2))/80000000 + 1369/4000000) - (1369*3^(1/2)*dq2*dqr5*cos(2*q5)*cos(q2)*cos(q3)*sin(q4))/4000000 - (1369*3^(1/2)*dq2*dqr5*sin(2*q5)*cos(q2)*cos(q3)*cos(q4))/8000000 + (1369*3^(1/2)*dq3*dqr5*cos(2*q5)*cos(q2)*cos(q3)*sin(q4))/4000000 + (1369*3^(1/2)*dq3*dqr5*sin(2*q5)*cos(q2)*cos(q3)*cos(q4))/8000000 - (1369*3^(1/2)*dq4*dqr5*cos(2*q5)*cos(q2)*cos(q4)*sin(q3))/4000000 + (1369*3^(1/2)*dq4*dqr5*cos(2*q5)*cos(q3)*cos(q4)*sin(q2))/4000000 + (1369*3^(1/2)*dq4*dqr5*sin(2*q5)*cos(q2)*sin(q3)*sin(q4))/8000000 - dq1*dqr5*cos(2*q2)*sin(2*q3)*sin(q4)*sin(q5)*((1369*3^(1/2))/4000000 - 45547/40000000) + dq1*dqr5*cos(2*q3)*sin(2*q2)*sin(q4)*sin(q5)*((1369*3^(1/2))/4000000 - 45547/40000000) - dq5*dqr5*cos(q2)*cos(q4)*cos(q5)*sin(q3)*((1369*3^(1/2))/2000000 + 58349/10000000) + dq2*dqr5*cos(q2)*cos(q3)*cos(q4)*sin(q5)*((1369*3^(1/2))/2000000 + 71151/40000000) - dq3*dqr5*cos(q2)*cos(q3)*cos(q4)*sin(q5)*((1369*3^(1/2))/2000000 + 71151/40000000) - dq1*dqr5*cos(2*q2)*cos(2*q3)*sin(2*q4)*cos(q5)*((23717*3^(1/2))/80000000 + 1369/4000000) - dq1*dqr5*cos(2*q2)*cos(2*q3)*cos(2*q4)*sin(q5)*((23717*3^(1/2))/160000000 + 1369/8000000) - dq1*dqr5*sin(2*q2)*sin(2*q3)*sin(2*q4)*cos(q5)*((23717*3^(1/2))/80000000 + 1369/4000000) - dq1*dqr5*cos(2*q4)*sin(2*q2)*sin(2*q3)*sin(q5)*((23717*3^(1/2))/160000000 + 1369/8000000);
Y1_5_8=(6139*ddqr2*sin(q2)*sin(q3))/4000000 - (6139*ddqr3*sin(q2)*sin(q3))/4000000 - (259*ddqr1*sin(q4)*sin(q5))/500000 + (1369*ddqr5*sin(q2)*sin(q3))/2000000 + (25433*ddqr1*sin(2*q2)*sin(q3))/400000 - (1073*ddqr1*cos(q4)*sin(q3)*sin(q5))/100000 - (1073*ddqr1*cos(q5)*sin(q3)*sin(q4))/200000 + (1073*ddqr2*cos(q2)*sin(q4)*sin(q5))/100000 - (1073*ddqr4*cos(q4)*sin(q2)*sin(q5))/100000 - (1073*ddqr4*cos(q5)*sin(q2)*sin(q4))/200000 - (1073*ddqr5*cos(q4)*sin(q2)*sin(q5))/200000 - (1073*ddqr5*cos(q5)*sin(q2)*sin(q4))/100000 + ddqr1*sin(q3)*sin(q4)*((18589*3^(1/2))/2000000 + 1073/100000) + ddqr4*sin(q2)*sin(q4)*((18589*3^(1/2))/2000000 + 1073/100000) - (4107*ddqr4*cos(2*q5)*sin(q2)*sin(q3))/8000000 + ddqr4*sin(q2)*sin(q3)*((23717*3^(1/2))/10000000 + 2122493/400000000) + ddqr2*sin(2*q4)*cos(q2)*sin(q3)*((23717*3^(1/2))/20000000 + 1574893/800000000) - ddqr2*sin(2*q4)*cos(q3)*sin(q2)*((23717*3^(1/2))/20000000 + 1574893/800000000) - ddqr3*sin(2*q4)*cos(q2)*sin(q3)*((23717*3^(1/2))/20000000 + 1574893/800000000) + ddqr3*sin(2*q4)*cos(q3)*sin(q2)*((23717*3^(1/2))/20000000 + 1574893/800000000) + (1073*3^(1/2)*ddqr1*sin(2*q2)*cos(q5)*sin(q3))/200000 - (32449*ddqr2*cos(q2)*cos(q3)*sin(q4)*sin(q5))/4000000 + (259*ddqr2*cos(q2)*cos(q4)*sin(q3)*sin(q5))/1000000 + (259*ddqr2*cos(q2)*cos(q5)*sin(q3)*sin(q4))/2000000 - (259*ddqr2*cos(q3)*cos(q4)*sin(q2)*sin(q5))/1000000 - (259*ddqr2*cos(q3)*cos(q5)*sin(q2)*sin(q4))/2000000 + (32449*ddqr3*cos(q2)*cos(q3)*sin(q4)*sin(q5))/4000000 - (259*ddqr3*cos(q2)*cos(q4)*sin(q3)*sin(q5))/1000000 - (259*ddqr3*cos(q2)*cos(q5)*sin(q3)*sin(q4))/2000000 + (259*ddqr3*cos(q3)*cos(q4)*sin(q2)*sin(q5))/1000000 + (259*ddqr3*cos(q3)*cos(q5)*sin(q2)*sin(q4))/2000000 - (259*ddqr4*cos(q2)*cos(q3)*sin(q4)*sin(q5))/1000000 - (32449*ddqr4*cos(q2)*cos(q4)*sin(q3)*sin(q5))/4000000 + (32449*ddqr4*cos(q3)*cos(q4)*sin(q2)*sin(q5))/4000000 + (259*ddqr4*cos(q4)*cos(q5)*sin(q2)*sin(q3))/2000000 - (259*ddqr5*cos(q2)*cos(q3)*sin(q4)*sin(q5))/2000000 - (32449*ddqr5*cos(q2)*cos(q5)*sin(q3)*sin(q4))/4000000 + (32449*ddqr5*cos(q3)*cos(q5)*sin(q2)*sin(q4))/4000000 + (259*ddqr5*cos(q4)*cos(q5)*sin(q2)*sin(q3))/1000000 + ddqr1*cos(2*q2)*sin(2*q3)*sin(q4)*((548467*3^(1/2))/80000000 + 32449/4000000) - ddqr1*cos(2*q3)*sin(2*q2)*sin(q4)*((548467*3^(1/2))/80000000 + 32449/4000000) - ddqr2*cos(q2)*sin(q3)*sin(q4)*((4487*3^(1/2))/20000000 + 259/1000000) + ddqr2*cos(q3)*sin(q2)*sin(q4)*((4487*3^(1/2))/20000000 + 259/1000000) + ddqr3*cos(q2)*sin(q3)*sin(q4)*((4487*3^(1/2))/20000000 + 259/1000000) - ddqr3*cos(q3)*sin(q2)*sin(q4)*((4487*3^(1/2))/20000000 + 259/1000000) - ddqr4*cos(q4)*sin(q2)*sin(q3)*((4487*3^(1/2))/20000000 + 259/1000000) - ddqr4*cos(q5)*sin(q2)*sin(q3)*((23717*3^(1/2))/20000000 + 1369/1000000) - ddqr5*cos(q5)*sin(q2)*sin(q3)*((23717*3^(1/2))/20000000 + 1369/1000000) - ddqr2*cos(q4)*sin(q2)*sin(q3)*((548467*3^(1/2))/80000000 + 32449/4000000) + ddqr3*cos(q4)*sin(q2)*sin(q3)*((548467*3^(1/2))/80000000 + 32449/4000000) + ddqr4*cos(q2)*sin(q3)*sin(q4)*((548467*3^(1/2))/80000000 + 32449/4000000) - ddqr4*cos(q3)*sin(q2)*sin(q4)*((548467*3^(1/2))/80000000 + 32449/4000000) + (1073*ddqr1*cos(2*q2)*cos(q4)*sin(q3)*sin(q5))/100000 + (1073*ddqr1*cos(2*q2)*cos(q5)*sin(q3)*sin(q4))/200000 - (1073*ddqr1*sin(2*q2)*cos(q3)*cos(q4)*sin(q5))/100000 - (1073*ddqr1*sin(2*q2)*cos(q3)*cos(q5)*sin(q4))/200000 + (259*3^(1/2)*ddqr2*cos(q5)*sin(q2)*sin(q3))/2000000 - (259*3^(1/2)*ddqr3*cos(q5)*sin(q2)*sin(q3))/2000000 - (1369*3^(1/2)*ddqr5*cos(q2)*sin(q3)*sin(q4))/2000000 + (1369*3^(1/2)*ddqr5*cos(q3)*sin(q2)*sin(q4))/2000000 + (259*3^(1/2)*ddqr5*cos(q2)*sin(q3)*sin(q5))/2000000 - (259*3^(1/2)*ddqr5*cos(q3)*sin(q2)*sin(q5))/2000000 - ddqr1*cos(2*q2)*sin(q3)*sin(q4)*((18589*3^(1/2))/2000000 + 1073/100000) + ddqr1*sin(2*q2)*cos(q3)*sin(q4)*((18589*3^(1/2))/2000000 + 1073/100000) - (32449*ddqr1*cos(2*q2)*sin(2*q3)*cos(q4)*sin(q5))/4000000 + (32449*ddqr1*cos(2*q3)*sin(2*q2)*cos(q4)*sin(q5))/4000000 + (1369*ddqr2*cos(2*q4)*sin(2*q5)*cos(q2)*sin(q3))/4000000 - (1369*ddqr2*cos(2*q4)*sin(2*q5)*cos(q3)*sin(q2))/4000000 + (1369*ddqr2*cos(2*q5)*sin(2*q4)*cos(q2)*sin(q3))/3200000 - (1369*ddqr2*cos(2*q5)*sin(2*q4)*cos(q3)*sin(q2))/3200000 - (1369*ddqr3*cos(2*q4)*sin(2*q5)*cos(q2)*sin(q3))/4000000 + (1369*ddqr3*cos(2*q4)*sin(2*q5)*cos(q3)*sin(q2))/4000000 - (1369*ddqr3*cos(2*q5)*sin(2*q4)*cos(q2)*sin(q3))/3200000 + (1369*ddqr3*cos(2*q5)*sin(2*q4)*cos(q3)*sin(q2))/3200000 + ddqr1*cos(2*q2)*sin(2*q3)*cos(q5)*sin(q4)*((1369*3^(1/2))/2000000 - 45547/20000000) - ddqr1*cos(2*q3)*sin(2*q2)*cos(q5)*sin(q4)*((1369*3^(1/2))/2000000 - 45547/20000000) - ddqr5*cos(q2)*cos(q4)*sin(q3)*sin(q5)*((1369*3^(1/2))/2000000 + 58349/10000000) + ddqr5*cos(q3)*cos(q4)*sin(q2)*sin(q5)*((1369*3^(1/2))/2000000 + 58349/10000000) + ddqr3*cos(q4)*cos(q5)*sin(q2)*sin(q3)*((1369*3^(1/2))/2000000 - 45547/20000000) + ddqr4*cos(q2)*cos(q5)*sin(q3)*sin(q4)*((1369*3^(1/2))/2000000 - 45547/20000000) - ddqr4*cos(q3)*cos(q5)*sin(q2)*sin(q4)*((1369*3^(1/2))/2000000 - 45547/20000000) - ddqr1*sin(2*q2)*sin(2*q3)*sin(2*q4)*sin(q5)*((23717*3^(1/2))/40000000 + 1369/2000000) - (1369*3^(1/2)*ddqr1*cos(2*q2)*cos(2*q5)*sin(2*q3)*sin(q4))/8000000 + (1369*3^(1/2)*ddqr1*cos(2*q3)*cos(2*q5)*sin(2*q2)*sin(q4))/8000000 - ddqr2*cos(2*q4)*cos(q2)*sin(q3)*sin(q5)*((23717*3^(1/2))/20000000 + 1369/1000000) + ddqr2*cos(2*q4)*cos(q3)*sin(q2)*sin(q5)*((23717*3^(1/2))/20000000 + 1369/1000000) + ddqr3*cos(2*q4)*cos(q2)*sin(q3)*sin(q5)*((23717*3^(1/2))/20000000 + 1369/1000000) - ddqr3*cos(2*q4)*cos(q3)*sin(q2)*sin(q5)*((23717*3^(1/2))/20000000 + 1369/1000000) - ddqr2*sin(2*q4)*cos(q2)*cos(q5)*sin(q3)*((23717*3^(1/2))/40000000 + 1369/2000000) + ddqr2*sin(2*q4)*cos(q3)*cos(q5)*sin(q2)*((23717*3^(1/2))/40000000 + 1369/2000000) + ddqr3*sin(2*q4)*cos(q2)*cos(q5)*sin(q3)*((23717*3^(1/2))/40000000 + 1369/2000000) - ddqr3*sin(2*q4)*cos(q3)*cos(q5)*sin(q2)*((23717*3^(1/2))/40000000 + 1369/2000000) + (1369*3^(1/2)*ddqr2*cos(2*q5)*cos(q4)*sin(q2)*sin(q3))/8000000 - (1369*3^(1/2)*ddqr2*sin(2*q5)*cos(q2)*cos(q3)*sin(q4))/4000000 - (1369*3^(1/2)*ddqr3*cos(2*q5)*cos(q4)*sin(q2)*sin(q3))/8000000 + (1369*3^(1/2)*ddqr3*sin(2*q5)*cos(q2)*cos(q3)*sin(q4))/4000000 - (1369*3^(1/2)*ddqr4*cos(2*q5)*cos(q2)*sin(q3)*sin(q4))/8000000 + (1369*3^(1/2)*ddqr4*cos(2*q5)*cos(q3)*sin(q2)*sin(q4))/8000000 - (1369*3^(1/2)*ddqr4*sin(2*q5)*cos(q2)*cos(q4)*sin(q3))/4000000 + (1369*3^(1/2)*ddqr4*sin(2*q5)*cos(q3)*cos(q4)*sin(q2))/4000000;
Y1_5_9=ddqr1*((71151*3^(1/2))/40000000 + 112593029/1600000000) - (25433*ddqr1*cos(q3))/400000 - (203*ddqr2*cos(q2))/100000 - (841*ddqr1*cos(2*q2))/20000 - (4107*ddqr1*cos(2*q5))/32000000 + (1369*ddqr1*cos(2*q4)*cos(2*q5))/6400000 - (1369*ddqr1*sin(2*q4)*sin(2*q5))/8000000 + (6139*ddqr2*cos(q2)*cos(q3))/4000000 - (6139*ddqr3*cos(q2)*cos(q3))/4000000 + (259*ddqr1*cos(q4)*cos(q5))/1000000 + (1369*ddqr5*cos(q2)*cos(q3))/2000000 + ddqr1*cos(2*q4)*((23717*3^(1/2))/40000000 + 1574893/1600000000) - ddqr1*cos(q4)*((4487*3^(1/2))/10000000 + 259/500000) + ddqr1*cos(q5)*((253339*3^(1/2))/80000000 - 4107/4000000) + (25433*ddqr1*cos(2*q2)*cos(q3))/400000 + ddqr1*sin(2*q4)*sin(q5)*((23717*3^(1/2))/40000000 + 1369/2000000) - (1073*ddqr2*cos(q2)*cos(q4)*cos(q5))/200000 - (12321*ddqr1*cos(2*q2)*cos(2*q3)*cos(2*q5))/32000000 - (12321*ddqr1*cos(2*q5)*sin(2*q2)*sin(2*q3))/32000000 + ddqr2*cos(q2)*cos(q4)*((18589*3^(1/2))/2000000 + 1073/100000) - (4107*ddqr4*cos(2*q5)*cos(q2)*cos(q3))/8000000 + ddqr4*cos(q2)*cos(q3)*((23717*3^(1/2))/10000000 + 2122493/400000000) + ddqr1*cos(2*q2)*cos(2*q3)*((23717*3^(1/2))/40000000 - 36744657/1600000000) - (1073*3^(1/2)*ddqr1*cos(q3)*cos(q5))/200000 + ddqr1*sin(2*q2)*sin(2*q3)*((23717*3^(1/2))/40000000 - 36744657/1600000000) - ddqr1*cos(2*q4)*cos(q5)*((23717*3^(1/2))/80000000 + 1369/4000000) + (259*ddqr4*cos(q2)*cos(q3)*cos(q4)*cos(q5))/2000000 + (259*ddqr5*cos(q2)*cos(q3)*cos(q4)*cos(q5))/1000000 - ddqr1*cos(2*q2)*cos(2*q3)*cos(q5)*((348207*3^(1/2))/80000000 + 1369/4000000) - ddqr1*sin(2*q2)*sin(2*q3)*cos(q5)*((348207*3^(1/2))/80000000 + 1369/4000000) - ddqr4*cos(q2)*cos(q3)*cos(q4)*((4487*3^(1/2))/20000000 + 259/1000000) - ddqr4*cos(q2)*cos(q3)*cos(q5)*((23717*3^(1/2))/20000000 + 1369/1000000) - ddqr5*cos(q2)*cos(q3)*cos(q5)*((23717*3^(1/2))/20000000 + 1369/1000000) - ddqr2*cos(q2)*cos(q3)*cos(q4)*((548467*3^(1/2))/80000000 + 32449/4000000) + ddqr3*cos(q2)*cos(q3)*cos(q4)*((548467*3^(1/2))/80000000 + 32449/4000000) - (1369*ddqr1*cos(2*q2)*cos(2*q3)*cos(2*q4)*cos(2*q5))/6400000 + (259*3^(1/2)*ddqr2*cos(q2)*cos(q3)*cos(q5))/2000000 - (259*3^(1/2)*ddqr3*cos(q2)*cos(q3)*cos(q5))/2000000 + (1369*ddqr1*cos(2*q2)*cos(2*q3)*sin(2*q4)*sin(2*q5))/8000000 - (1369*ddqr1*cos(2*q4)*cos(2*q5)*sin(2*q2)*sin(2*q3))/6400000 + (1369*ddqr1*sin(2*q2)*sin(2*q3)*sin(2*q4)*sin(2*q5))/8000000 - ddqr1*cos(2*q2)*cos(2*q3)*cos(2*q4)*((23717*3^(1/2))/40000000 + 1574893/1600000000) - ddqr1*cos(2*q4)*sin(2*q2)*sin(2*q3)*((23717*3^(1/2))/40000000 + 1574893/1600000000) + (1073*3^(1/2)*ddqr1*cos(2*q2)*cos(q3)*cos(q5))/200000 - ddqr2*cos(q2)*cos(q3)*cos(q4)*cos(q5)*((1369*3^(1/2))/2000000 - 45547/20000000) + ddqr3*cos(q2)*cos(q3)*cos(q4)*cos(q5)*((1369*3^(1/2))/2000000 - 45547/20000000) + ddqr1*cos(2*q2)*cos(2*q3)*cos(2*q4)*cos(q5)*((23717*3^(1/2))/80000000 + 1369/4000000) - ddqr1*cos(2*q2)*cos(2*q3)*sin(2*q4)*sin(q5)*((23717*3^(1/2))/40000000 + 1369/2000000) + ddqr1*cos(2*q4)*sin(2*q2)*sin(2*q3)*cos(q5)*((23717*3^(1/2))/80000000 + 1369/4000000) - (1369*3^(1/2)*ddqr1*cos(2*q2)*sin(2*q3)*sin(2*q5)*cos(q4))/4000000 + (1369*3^(1/2)*ddqr1*cos(2*q3)*sin(2*q2)*sin(2*q5)*cos(q4))/4000000 + (1369*3^(1/2)*ddqr2*cos(2*q5)*cos(q2)*cos(q3)*cos(q4))/8000000 - (1369*3^(1/2)*ddqr3*cos(2*q5)*cos(q2)*cos(q3)*cos(q4))/8000000;
Y1_6_1=(dq2*dqr2*sin(q2))/625 - (ddqr2*cos(q2))/625;
Y1_7_1=(29*dq1*dqr3*sin(q3))/200 - (29*ddqr1*cos(q3))/100 + (29*dq3*dqr1*sin(q3))/200 - (ddqr2*cos(q2)*cos(q3))/625 + (ddqr3*cos(q2)*cos(q3))/625 - (ddqr2*sin(q2)*sin(q3))/625 + (ddqr3*sin(q2)*sin(q3))/625 + (29*ddqr1*cos(2*q2)*cos(q3))/100 + (29*ddqr1*sin(2*q2)*sin(q3))/100 + (29*dq1*dqr2*cos(2*q2)*sin(q3))/100 - (29*dq1*dqr2*sin(2*q2)*cos(q3))/100 + (29*dq2*dqr1*cos(2*q2)*sin(q3))/100 - (29*dq2*dqr1*sin(2*q2)*cos(q3))/100 - (29*dq1*dqr3*cos(2*q2)*sin(q3))/200 + (29*dq1*dqr3*sin(2*q2)*cos(q3))/200 - (29*dq3*dqr1*cos(2*q2)*sin(q3))/200 + (29*dq3*dqr1*sin(2*q2)*cos(q3))/200 - (dq2*dqr2*cos(q2)*sin(q3))/625 + (dq2*dqr2*cos(q3)*sin(q2))/625 + (dq2*dqr3*cos(q2)*sin(q3))/625 - (dq2*dqr3*cos(q3)*sin(q2))/625 + (dq3*dqr2*cos(q2)*sin(q3))/625 - (dq3*dqr2*cos(q3)*sin(q2))/625 - (dq3*dqr3*cos(q2)*sin(q3))/625 + (dq3*dqr3*cos(q3)*sin(q2))/625;
Y1_8_1=(7*ddqr1*cos(q4))/500 - (7*dq1*dqr4*sin(q4))/1000 - (7*dq4*dqr1*sin(q4))/1000 - (29*ddqr2*cos(q2)*cos(q4))/100 - (29*ddqr1*sin(q3)*sin(q4))/100 - (29*ddqr4*sin(q2)*sin(q4))/100 - (1231*ddqr1*cos(2*q2)*sin(2*q3)*sin(q4))/10000 + (1231*ddqr1*cos(2*q3)*sin(2*q2)*sin(q4))/10000 + (1231*ddqr2*cos(q2)*cos(q3)*cos(q4))/10000 - (1231*ddqr3*cos(q2)*cos(q3)*cos(q4))/10000 + (7*ddqr4*cos(q2)*cos(q3)*cos(q4))/1000 + (7*ddqr2*cos(q2)*sin(q3)*sin(q4))/1000 - (7*ddqr2*cos(q3)*sin(q2)*sin(q4))/1000 + (1231*ddqr2*cos(q4)*sin(q2)*sin(q3))/10000 - (7*ddqr3*cos(q2)*sin(q3)*sin(q4))/1000 + (7*ddqr3*cos(q3)*sin(q2)*sin(q4))/1000 - (1231*ddqr3*cos(q4)*sin(q2)*sin(q3))/10000 - (1231*ddqr4*cos(q2)*sin(q3)*sin(q4))/10000 + (1231*ddqr4*cos(q3)*sin(q2)*sin(q4))/10000 + (7*ddqr4*cos(q4)*sin(q2)*sin(q3))/1000 + (29*ddqr1*cos(2*q2)*sin(q3)*sin(q4))/100 - (29*ddqr1*sin(2*q2)*cos(q3)*sin(q4))/100 + (29*dq2*dqr2*cos(q4)*sin(q2))/100 - (29*dq1*dqr3*cos(q3)*sin(q4))/200 - (29*dq3*dqr1*cos(q3)*sin(q4))/200 - (29*dq1*dqr4*cos(q4)*sin(q3))/200 - (29*dq4*dqr1*cos(q4)*sin(q3))/200 - (29*dq4*dqr4*cos(q4)*sin(q2))/100 - (29*dq1*dqr2*cos(2*q2)*cos(q3)*sin(q4))/100 - (29*dq2*dqr1*cos(2*q2)*cos(q3)*sin(q4))/100 + (29*dq1*dqr3*cos(2*q2)*cos(q3)*sin(q4))/200 + (29*dq3*dqr1*cos(2*q2)*cos(q3)*sin(q4))/200 + (29*dq1*dqr4*cos(2*q2)*cos(q4)*sin(q3))/200 - (29*dq1*dqr4*sin(2*q2)*cos(q3)*cos(q4))/200 + (29*dq4*dqr1*cos(2*q2)*cos(q4)*sin(q3))/200 - (29*dq4*dqr1*sin(2*q2)*cos(q3)*cos(q4))/200 - (29*dq1*dqr2*sin(2*q2)*sin(q3)*sin(q4))/100 - (29*dq2*dqr1*sin(2*q2)*sin(q3)*sin(q4))/100 + (29*dq1*dqr3*sin(2*q2)*sin(q3)*sin(q4))/200 + (29*dq3*dqr1*sin(2*q2)*sin(q3)*sin(q4))/200 + (1231*dq1*dqr2*cos(2*q2)*cos(2*q3)*sin(q4))/10000 + (1231*dq2*dqr1*cos(2*q2)*cos(2*q3)*sin(q4))/10000 - (1231*dq1*dqr3*cos(2*q2)*cos(2*q3)*sin(q4))/10000 - (1231*dq3*dqr1*cos(2*q2)*cos(2*q3)*sin(q4))/10000 - (1231*dq1*dqr4*cos(2*q2)*sin(2*q3)*cos(q4))/20000 + (1231*dq1*dqr4*cos(2*q3)*sin(2*q2)*cos(q4))/20000 - (1231*dq4*dqr1*cos(2*q2)*sin(2*q3)*cos(q4))/20000 + (1231*dq4*dqr1*cos(2*q3)*sin(2*q2)*cos(q4))/20000 + (1231*dq1*dqr2*sin(2*q2)*sin(2*q3)*sin(q4))/10000 + (1231*dq2*dqr1*sin(2*q2)*sin(2*q3)*sin(q4))/10000 - (1231*dq1*dqr3*sin(2*q2)*sin(2*q3)*sin(q4))/10000 - (1231*dq3*dqr1*sin(2*q2)*sin(2*q3)*sin(q4))/10000 - (7*dq2*dqr2*cos(q2)*cos(q3)*sin(q4))/1000 + (1231*dq2*dqr2*cos(q2)*cos(q4)*sin(q3))/10000 - (1231*dq2*dqr2*cos(q3)*cos(q4)*sin(q2))/10000 + (7*dq2*dqr3*cos(q2)*cos(q3)*sin(q4))/1000 - (1231*dq2*dqr3*cos(q2)*cos(q4)*sin(q3))/10000 + (1231*dq2*dqr3*cos(q3)*cos(q4)*sin(q2))/10000 + (7*dq3*dqr2*cos(q2)*cos(q3)*sin(q4))/1000 - (1231*dq3*dqr2*cos(q2)*cos(q4)*sin(q3))/10000 + (1231*dq3*dqr2*cos(q3)*cos(q4)*sin(q2))/10000 + (7*dq2*dqr4*cos(q2)*cos(q4)*sin(q3))/1000 - (7*dq2*dqr4*cos(q3)*cos(q4)*sin(q2))/1000 - (7*dq3*dqr3*cos(q2)*cos(q3)*sin(q4))/1000 + (1231*dq3*dqr3*cos(q2)*cos(q4)*sin(q3))/10000 - (1231*dq3*dqr3*cos(q3)*cos(q4)*sin(q2))/10000 + (7*dq4*dqr2*cos(q2)*cos(q4)*sin(q3))/1000 - (7*dq4*dqr2*cos(q3)*cos(q4)*sin(q2))/1000 - (7*dq3*dqr4*cos(q2)*cos(q4)*sin(q3))/1000 + (7*dq3*dqr4*cos(q3)*cos(q4)*sin(q2))/1000 - (7*dq4*dqr3*cos(q2)*cos(q4)*sin(q3))/1000 + (7*dq4*dqr3*cos(q3)*cos(q4)*sin(q2))/1000 - (7*dq4*dqr4*cos(q2)*cos(q3)*sin(q4))/1000 - (1231*dq4*dqr4*cos(q2)*cos(q4)*sin(q3))/10000 + (1231*dq4*dqr4*cos(q3)*cos(q4)*sin(q2))/10000 - (7*dq2*dqr2*sin(q2)*sin(q3)*sin(q4))/1000 + (7*dq2*dqr3*sin(q2)*sin(q3)*sin(q4))/1000 + (7*dq3*dqr2*sin(q2)*sin(q3)*sin(q4))/1000 - (7*dq3*dqr3*sin(q2)*sin(q3)*sin(q4))/1000 - (7*dq4*dqr4*sin(q2)*sin(q3)*sin(q4))/1000;
Y1_9_1=dq5*dqr1*sin(q5)*((117*3^(1/2))/2500 - 111/8000) - (37*dq4*dqr1*cos(2*q4)*sin(q5))/2000 - (37*dq4*dqr1*sin(2*q4)*cos(q5))/4000 - (37*dq5*dqr1*cos(2*q4)*sin(q5))/8000 - (37*dq5*dqr1*sin(2*q4)*cos(q5))/4000 + (7*dq4*dqr1*cos(q4)*sin(q5))/1000 + (7*dq4*dqr1*cos(q5)*sin(q4))/2000 + (7*dq5*dqr1*cos(q4)*sin(q5))/2000 + (7*dq5*dqr1*cos(q5)*sin(q4))/1000 - (29*3^(1/2)*dq3*dqr1*cos(q5)*sin(q3))/400 - (29*3^(1/2)*dq5*dqr1*cos(q3)*sin(q5))/400 + (29*dq3*dqr1*cos(q3)*cos(q4)*sin(q5))/200 + (29*dq3*dqr1*cos(q3)*cos(q5)*sin(q4))/400 + (29*dq4*dqr1*cos(q4)*cos(q5)*sin(q3))/400 + (29*dq5*dqr1*cos(q4)*cos(q5)*sin(q3))/200 + (29*dq2*dqr2*sin(q2)*sin(q4)*sin(q5))/100 - (29*dq4*dqr1*sin(q3)*sin(q4)*sin(q5))/200 - (29*dq5*dqr1*sin(q3)*sin(q4)*sin(q5))/400 + (29*dq2*dqr1*sin(2*q2)*cos(q4)*sin(q3)*sin(q5))/100 + (29*dq2*dqr1*sin(2*q2)*cos(q5)*sin(q3)*sin(q4))/200 - (37*dq2*dqr2*cos(2*q4)*sin(q2)*sin(q3)*sin(q5))/1000 - (37*dq2*dqr2*sin(2*q4)*cos(q5)*sin(q2)*sin(q3))/2000 - (29*dq3*dqr1*sin(2*q2)*cos(q4)*sin(q3)*sin(q5))/200 - (29*dq3*dqr1*sin(2*q2)*cos(q5)*sin(q3)*sin(q4))/400 + (37*dq3*dqr2*cos(2*q4)*sin(q2)*sin(q3)*sin(q5))/1000 + (37*dq3*dqr2*sin(2*q4)*cos(q5)*sin(q2)*sin(q3))/2000 + (29*dq4*dqr1*cos(2*q2)*sin(q3)*sin(q4)*sin(q5))/200 - (29*dq4*dqr1*sin(2*q2)*cos(q3)*sin(q4)*sin(q5))/200 + (37*dq4*dqr2*sin(2*q4)*cos(q3)*sin(q2)*sin(q5))/1000 + (29*dq5*dqr1*cos(2*q2)*sin(q3)*sin(q4)*sin(q5))/400 - (29*dq5*dqr1*sin(2*q2)*cos(q3)*sin(q4)*sin(q5))/400 + (37*dq5*dqr2*sin(2*q4)*cos(q3)*sin(q2)*sin(q5))/4000 + (7*3^(1/2)*dq2*dqr2*cos(q3)*cos(q5)*sin(q2))/2000 - (7*3^(1/2)*dq3*dqr2*cos(q3)*cos(q5)*sin(q2))/2000 + (7*3^(1/2)*dq5*dqr2*sin(q2)*sin(q3)*sin(q5))/2000 - (117*dq2*dqr1*cos(2*q2)*cos(2*q3)*cos(q4)*sin(q5))/625 + (117*dq3*dqr1*cos(2*q2)*cos(2*q3)*cos(q4)*sin(q5))/625 + (117*dq5*dqr1*cos(2*q2)*sin(2*q3)*cos(q4)*cos(q5))/1250 - (117*dq5*dqr1*cos(2*q3)*sin(2*q2)*cos(q4)*cos(q5))/1250 - (117*dq2*dqr1*sin(2*q2)*sin(2*q3)*cos(q4)*sin(q5))/625 + (117*dq3*dqr1*sin(2*q2)*sin(2*q3)*cos(q4)*sin(q5))/625 - (117*dq4*dqr1*cos(2*q2)*sin(2*q3)*sin(q4)*sin(q5))/1250 + (117*dq4*dqr1*cos(2*q3)*sin(2*q2)*sin(q4)*sin(q5))/1250 - (29*3^(1/2)*dq2*dqr1*cos(2*q2)*cos(q5)*sin(q3))/200 + (29*3^(1/2)*dq2*dqr1*sin(2*q2)*cos(q3)*cos(q5))/200 + (29*3^(1/2)*dq3*dqr1*cos(2*q2)*cos(q5)*sin(q3))/400 - (29*3^(1/2)*dq3*dqr1*sin(2*q2)*cos(q3)*cos(q5))/400 + (29*3^(1/2)*dq5*dqr1*cos(2*q2)*cos(q3)*sin(q5))/400 + (7*dq4*dqr2*cos(q3)*cos(q4)*cos(q5)*sin(q2))/2000 + (7*dq5*dqr2*cos(q3)*cos(q4)*cos(q5)*sin(q2))/1000 + dq2*dqr1*cos(2*q2)*sin(2*q3)*cos(q5)*((117*3^(1/2))/1250 + 37/4000) - dq2*dqr1*cos(2*q3)*sin(2*q2)*cos(q5)*((117*3^(1/2))/1250 + 37/4000) - dq3*dqr1*cos(2*q2)*sin(2*q3)*cos(q5)*((117*3^(1/2))/1250 + 37/4000) + dq3*dqr1*cos(2*q3)*sin(2*q2)*cos(q5)*((117*3^(1/2))/1250 + 37/4000) - dq5*dqr1*cos(2*q2)*cos(2*q3)*sin(q5)*((117*3^(1/2))/2500 + 37/8000) + (29*3^(1/2)*dq5*dqr1*sin(2*q2)*sin(q3)*sin(q5))/400 - (37*dq2*dqr1*cos(2*q2)*cos(2*q4)*sin(2*q3)*cos(q5))/4000 + (37*dq2*dqr1*cos(2*q3)*cos(2*q4)*sin(2*q2)*cos(q5))/4000 + (37*dq3*dqr1*cos(2*q2)*cos(2*q4)*sin(2*q3)*cos(q5))/4000 - (37*dq3*dqr1*cos(2*q3)*cos(2*q4)*sin(2*q2)*cos(q5))/4000 + (37*dq4*dqr1*cos(2*q2)*cos(2*q3)*cos(2*q4)*sin(q5))/2000 + (37*dq4*dqr1*cos(2*q2)*cos(2*q3)*sin(2*q4)*cos(q5))/4000 + (37*dq5*dqr1*cos(2*q2)*cos(2*q3)*cos(2*q4)*sin(q5))/8000 + (37*dq5*dqr1*cos(2*q2)*cos(2*q3)*sin(2*q4)*cos(q5))/4000 - (117*dq2*dqr2*cos(q3)*sin(q2)*sin(q4)*sin(q5))/625 + (7*dq2*dqr2*cos(q4)*sin(q2)*sin(q3)*sin(q5))/1000 + (7*dq2*dqr2*cos(q5)*sin(q2)*sin(q3)*sin(q4))/2000 + (117*dq3*dqr2*cos(q3)*sin(q2)*sin(q4)*sin(q5))/625 - (7*dq3*dqr2*cos(q4)*sin(q2)*sin(q3)*sin(q5))/1000 - (7*dq3*dqr2*cos(q5)*sin(q2)*sin(q3)*sin(q4))/2000 - (7*dq4*dqr2*cos(q3)*sin(q2)*sin(q4)*sin(q5))/1000 - (7*dq5*dqr2*cos(q3)*sin(q2)*sin(q4)*sin(q5))/2000 - dq5*dqr1*sin(2*q2)*sin(2*q3)*sin(q5)*((117*3^(1/2))/2500 + 37/8000) + (37*dq2*dqr1*cos(2*q2)*sin(2*q3)*sin(2*q4)*sin(q5))/2000 - (37*dq2*dqr1*cos(2*q3)*sin(2*q2)*sin(2*q4)*sin(q5))/2000 - (37*dq3*dqr1*cos(2*q2)*sin(2*q3)*sin(2*q4)*sin(q5))/2000 + (37*dq3*dqr1*cos(2*q3)*sin(2*q2)*sin(2*q4)*sin(q5))/2000 + (37*dq4*dqr1*cos(2*q4)*sin(2*q2)*sin(2*q3)*sin(q5))/2000 + (37*dq4*dqr1*sin(2*q2)*sin(2*q3)*sin(2*q4)*cos(q5))/4000 + (37*dq5*dqr1*cos(2*q4)*sin(2*q2)*sin(2*q3)*sin(q5))/8000 + (37*dq5*dqr1*sin(2*q2)*sin(2*q3)*sin(2*q4)*cos(q5))/4000 + (29*dq2*dqr1*cos(2*q2)*cos(q3)*cos(q4)*sin(q5))/100 + (29*dq2*dqr1*cos(2*q2)*cos(q3)*cos(q5)*sin(q4))/200 - (29*dq3*dqr1*cos(2*q2)*cos(q3)*cos(q4)*sin(q5))/200 - (29*dq3*dqr1*cos(2*q2)*cos(q3)*cos(q5)*sin(q4))/400 - (29*dq4*dqr1*cos(2*q2)*cos(q4)*cos(q5)*sin(q3))/400 + (29*dq4*dqr1*sin(2*q2)*cos(q3)*cos(q4)*cos(q5))/400 - (29*dq5*dqr1*cos(2*q2)*cos(q4)*cos(q5)*sin(q3))/200 + (29*dq5*dqr1*sin(2*q2)*cos(q3)*cos(q4)*cos(q5))/200 - (37*3^(1/2)*dq5*dqr2*cos(q4)*sin(q2)*sin(q3)*sin(q5))/2000 + dq2*dqr1*cos(2*q2)*cos(2*q3)*cos(q5)*sin(q4)*((37*3^(1/2))/2000 - 117/1250) - dq3*dqr1*cos(2*q2)*cos(2*q3)*cos(q5)*sin(q4)*((37*3^(1/2))/2000 - 117/1250) - dq4*dqr1*cos(2*q2)*sin(2*q3)*cos(q4)*cos(q5)*((37*3^(1/2))/4000 - 117/2500) + dq4*dqr1*cos(2*q3)*sin(2*q2)*cos(q4)*cos(q5)*((37*3^(1/2))/4000 - 117/2500) + dq2*dqr1*sin(2*q2)*sin(2*q3)*cos(q5)*sin(q4)*((37*3^(1/2))/2000 - 117/1250) - dq3*dqr1*sin(2*q2)*sin(2*q3)*cos(q5)*sin(q4)*((37*3^(1/2))/2000 - 117/1250) + dq5*dqr1*cos(2*q2)*sin(2*q3)*sin(q4)*sin(q5)*((37*3^(1/2))/4000 - 117/2500) - dq5*dqr1*cos(2*q3)*sin(2*q2)*sin(q4)*sin(q5)*((37*3^(1/2))/4000 - 117/2500) - dq2*dqr2*cos(q3)*cos(q4)*cos(q5)*sin(q2)*((37*3^(1/2))/2000 - 117/1250) + dq3*dqr2*cos(q3)*cos(q4)*cos(q5)*sin(q2)*((37*3^(1/2))/2000 - 117/1250);
Y1_9_2=(29*dq1*dqr3*cos(q3)*cos(q5)*sin(q4))/400 - (29*dq2*dqr2*cos(q4)*cos(q5)*sin(q2))/200 - (29*3^(1/2)*dq1*dqr3*cos(q5)*sin(q3))/400 + (37*dq4*dqr2*cos(q2)*cos(q5)*sin(q3))/2000 - (37*dq4*dqr2*cos(q3)*cos(q5)*sin(q2))/2000 - (37*dq4*dqr3*cos(q2)*cos(q5)*sin(q3))/2000 + (37*dq4*dqr3*cos(q3)*cos(q5)*sin(q2))/2000 + (37*dq5*dqr2*cos(q2)*cos(q5)*sin(q3))/2000 - (37*dq5*dqr2*cos(q3)*cos(q5)*sin(q2))/2000 - (37*dq5*dqr3*cos(q2)*cos(q5)*sin(q3))/2000 + (37*dq5*dqr3*cos(q3)*cos(q5)*sin(q2))/2000 + (29*dq1*dqr2*sin(2*q2)*cos(q4)*sin(q3)*sin(q5))/100 + (29*dq1*dqr2*sin(2*q2)*cos(q5)*sin(q3)*sin(q4))/200 - (29*dq1*dqr3*sin(2*q2)*cos(q4)*sin(q3)*sin(q5))/200 - (29*dq1*dqr3*sin(2*q2)*cos(q5)*sin(q3)*sin(q4))/400 + (37*dq2*dqr3*cos(2*q4)*sin(q2)*sin(q3)*sin(q5))/1000 + (37*dq2*dqr3*sin(2*q4)*cos(q5)*sin(q2)*sin(q3))/2000 - (37*dq3*dqr3*cos(2*q4)*sin(q2)*sin(q3)*sin(q5))/1000 - (37*dq3*dqr3*sin(2*q4)*cos(q5)*sin(q2)*sin(q3))/2000 - (37*dq4*dqr2*sin(2*q4)*cos(q2)*sin(q3)*sin(q5))/1000 + (37*dq4*dqr3*sin(2*q4)*cos(q2)*sin(q3)*sin(q5))/1000 - (37*dq4*dqr3*sin(2*q4)*cos(q3)*sin(q2)*sin(q5))/1000 - (37*dq5*dqr2*sin(2*q4)*cos(q2)*sin(q3)*sin(q5))/4000 + (37*dq5*dqr3*sin(2*q4)*cos(q2)*sin(q3)*sin(q5))/4000 - (37*dq5*dqr3*sin(2*q4)*cos(q3)*sin(q2)*sin(q5))/4000 - (7*3^(1/2)*dq2*dqr2*cos(q2)*cos(q5)*sin(q3))/2000 + (7*3^(1/2)*dq2*dqr3*cos(q2)*cos(q5)*sin(q3))/2000 - (7*3^(1/2)*dq2*dqr3*cos(q3)*cos(q5)*sin(q2))/2000 + (7*3^(1/2)*dq3*dqr2*cos(q2)*cos(q5)*sin(q3))/2000 - (7*3^(1/2)*dq3*dqr3*cos(q2)*cos(q5)*sin(q3))/2000 + (7*3^(1/2)*dq3*dqr3*cos(q3)*cos(q5)*sin(q2))/2000 + (7*3^(1/2)*dq5*dqr2*cos(q2)*cos(q3)*sin(q5))/2000 - (7*3^(1/2)*dq5*dqr3*sin(q2)*sin(q3)*sin(q5))/2000 - (117*dq1*dqr2*cos(2*q2)*cos(2*q3)*cos(q4)*sin(q5))/625 - (117*dq1*dqr2*sin(2*q2)*sin(2*q3)*cos(q4)*sin(q5))/625 - (29*3^(1/2)*dq1*dqr2*cos(2*q2)*cos(q5)*sin(q3))/200 + (29*3^(1/2)*dq1*dqr2*sin(2*q2)*cos(q3)*cos(q5))/200 + (29*3^(1/2)*dq1*dqr3*cos(2*q2)*cos(q5)*sin(q3))/400 + (7*dq2*dqr2*cos(q2)*cos(q3)*cos(q4)*sin(q5))/1000 + (7*dq2*dqr2*cos(q2)*cos(q3)*cos(q5)*sin(q4))/2000 - (7*dq2*dqr3*cos(q2)*cos(q3)*cos(q4)*sin(q5))/1000 - (7*dq2*dqr3*cos(q2)*cos(q3)*cos(q5)*sin(q4))/2000 - (7*dq3*dqr2*cos(q2)*cos(q3)*cos(q4)*sin(q5))/1000 - (7*dq3*dqr2*cos(q2)*cos(q3)*cos(q5)*sin(q4))/2000 + (7*dq3*dqr3*cos(q2)*cos(q3)*cos(q5)*sin(q4))/2000 - (7*dq4*dqr2*cos(q2)*cos(q4)*cos(q5)*sin(q3))/2000 + (7*dq4*dqr3*cos(q2)*cos(q4)*cos(q5)*sin(q3))/2000 - (7*dq4*dqr3*cos(q3)*cos(q4)*cos(q5)*sin(q2))/2000 - (7*dq5*dqr2*cos(q2)*cos(q4)*cos(q5)*sin(q3))/1000 + (7*dq5*dqr3*cos(q2)*cos(q4)*cos(q5)*sin(q3))/1000 - (7*dq5*dqr3*cos(q3)*cos(q4)*cos(q5)*sin(q2))/1000 + dq1*dqr2*cos(2*q2)*sin(2*q3)*cos(q5)*((117*3^(1/2))/1250 + 37/4000) - dq1*dqr2*cos(2*q3)*sin(2*q2)*cos(q5)*((117*3^(1/2))/1250 + 37/4000) - (37*dq1*dqr2*cos(2*q2)*cos(2*q4)*sin(2*q3)*cos(q5))/4000 + (37*dq1*dqr2*cos(2*q3)*cos(2*q4)*sin(2*q2)*cos(q5))/4000 + (117*dq2*dqr2*cos(q2)*sin(q3)*sin(q4)*sin(q5))/625 - (117*dq2*dqr3*cos(q2)*sin(q3)*sin(q4)*sin(q5))/625 + (117*dq2*dqr3*cos(q3)*sin(q2)*sin(q4)*sin(q5))/625 - (7*dq2*dqr3*cos(q4)*sin(q2)*sin(q3)*sin(q5))/1000 - (7*dq2*dqr3*cos(q5)*sin(q2)*sin(q3)*sin(q4))/2000 - (117*dq3*dqr2*cos(q2)*sin(q3)*sin(q4)*sin(q5))/625 + (117*dq3*dqr3*cos(q2)*sin(q3)*sin(q4)*sin(q5))/625 - (117*dq3*dqr3*cos(q3)*sin(q2)*sin(q4)*sin(q5))/625 + (7*dq3*dqr3*cos(q4)*sin(q2)*sin(q3)*sin(q5))/1000 + (7*dq3*dqr3*cos(q5)*sin(q2)*sin(q3)*sin(q4))/2000 + (7*dq4*dqr2*cos(q2)*sin(q3)*sin(q4)*sin(q5))/1000 - (7*dq4*dqr3*cos(q2)*sin(q3)*sin(q4)*sin(q5))/1000 + (7*dq4*dqr3*cos(q3)*sin(q2)*sin(q4)*sin(q5))/1000 + (7*dq5*dqr2*cos(q2)*sin(q3)*sin(q4)*sin(q5))/2000 - (7*dq5*dqr3*cos(q2)*sin(q3)*sin(q4)*sin(q5))/2000 + (7*dq5*dqr3*cos(q3)*sin(q2)*sin(q4)*sin(q5))/2000 + (37*dq1*dqr2*cos(2*q2)*sin(2*q3)*sin(2*q4)*sin(q5))/2000 - (37*dq1*dqr2*cos(2*q3)*sin(2*q2)*sin(2*q4)*sin(q5))/2000 + (29*dq1*dqr2*cos(2*q2)*cos(q3)*cos(q4)*sin(q5))/100 + (29*dq1*dqr2*cos(2*q2)*cos(q3)*cos(q5)*sin(q4))/200 - (29*dq1*dqr3*cos(2*q2)*cos(q3)*cos(q5)*sin(q4))/400 - (37*dq2*dqr2*cos(2*q4)*cos(q2)*cos(q3)*sin(q5))/1000 - (37*dq2*dqr2*sin(2*q4)*cos(q2)*cos(q3)*cos(q5))/2000 + (37*dq3*dqr2*cos(2*q4)*cos(q2)*cos(q3)*sin(q5))/1000 + (37*dq3*dqr2*sin(2*q4)*cos(q2)*cos(q3)*cos(q5))/2000 + (37*dq4*dqr2*cos(2*q4)*cos(q2)*cos(q5)*sin(q3))/2000 - (37*dq4*dqr2*cos(2*q4)*cos(q3)*cos(q5)*sin(q2))/2000 - (37*dq4*dqr3*cos(2*q4)*cos(q2)*cos(q5)*sin(q3))/2000 + (37*dq4*dqr3*cos(2*q4)*cos(q3)*cos(q5)*sin(q2))/2000 + (37*dq5*dqr2*cos(2*q4)*cos(q2)*cos(q5)*sin(q3))/2000 - (37*dq5*dqr2*cos(2*q4)*cos(q3)*cos(q5)*sin(q2))/2000 - (37*dq5*dqr3*cos(2*q4)*cos(q2)*cos(q5)*sin(q3))/2000 + (37*dq5*dqr3*cos(2*q4)*cos(q3)*cos(q5)*sin(q2))/2000 + (37*3^(1/2)*dq5*dqr3*cos(q4)*sin(q2)*sin(q3)*sin(q5))/2000 + dq1*dqr2*cos(2*q2)*cos(2*q3)*cos(q5)*sin(q4)*((37*3^(1/2))/2000 - 117/1250) - dq1*dqr3*cos(2*q2)*cos(2*q3)*cos(q5)*sin(q4)*((37*3^(1/2))/2000 - 117/1250) + dq1*dqr2*sin(2*q2)*sin(2*q3)*cos(q5)*sin(q4)*((37*3^(1/2))/2000 - 117/1250) - dq1*dqr3*sin(2*q2)*sin(2*q3)*cos(q5)*sin(q4)*((37*3^(1/2))/2000 - 117/1250) + dq2*dqr2*cos(q2)*cos(q4)*cos(q5)*sin(q3)*((37*3^(1/2))/2000 - 117/1250) - dq2*dqr3*cos(q2)*cos(q4)*cos(q5)*sin(q3)*((37*3^(1/2))/2000 - 117/1250) + dq2*dqr3*cos(q3)*cos(q4)*cos(q5)*sin(q2)*((37*3^(1/2))/2000 - 117/1250) - dq3*dqr2*cos(q2)*cos(q4)*cos(q5)*sin(q3)*((37*3^(1/2))/2000 - 117/1250) + dq3*dqr3*cos(q2)*cos(q4)*cos(q5)*sin(q3)*((37*3^(1/2))/2000 - 117/1250) - dq3*dqr3*cos(q3)*cos(q4)*cos(q5)*sin(q2)*((37*3^(1/2))/2000 - 117/1250) - (37*3^(1/2)*dq5*dqr2*cos(q2)*cos(q3)*cos(q4)*sin(q5))/2000;
Y1_9_3=(7*dq1*dqr4*cos(q4)*sin(q5))/1000 - (37*dq1*dqr4*sin(2*q4)*cos(q5))/4000 - (37*dq1*dqr4*cos(2*q4)*sin(q5))/2000 + (7*dq1*dqr4*cos(q5)*sin(q4))/2000 + (29*dq1*dqr3*cos(q3)*cos(q4)*sin(q5))/200 + (37*dq2*dqr4*cos(q2)*cos(q5)*sin(q3))/2000 - (37*dq2*dqr4*cos(q3)*cos(q5)*sin(q2))/2000 + (29*dq1*dqr4*cos(q4)*cos(q5)*sin(q3))/400 - (37*dq3*dqr4*cos(q2)*cos(q5)*sin(q3))/2000 + (37*dq3*dqr4*cos(q3)*cos(q5)*sin(q2))/2000 + (29*dq4*dqr4*cos(q4)*cos(q5)*sin(q2))/200 - (37*dq5*dqr4*cos(q2)*cos(q3)*sin(q5))/2000 + (29*dq5*dqr4*cos(q4)*cos(q5)*sin(q2))/100 - (29*dq1*dqr4*sin(q3)*sin(q4)*sin(q5))/200 - (29*dq4*dqr4*sin(q2)*sin(q4)*sin(q5))/100 - (37*dq4*dqr5*sin(q2)*sin(q3)*sin(q5))/2000 - (37*dq5*dqr4*sin(q2)*sin(q3)*sin(q5))/2000 - (29*dq4*dqr5*sin(q2)*sin(q4)*sin(q5))/200 - (29*dq5*dqr4*sin(q2)*sin(q4)*sin(q5))/200 - (37*dq5*dqr5*sin(q2)*sin(q3)*sin(q5))/1000 - (29*dq5*dqr5*sin(q2)*sin(q4)*sin(q5))/100 + (29*dq1*dqr4*cos(2*q2)*sin(q3)*sin(q4)*sin(q5))/200 - (29*dq1*dqr4*sin(2*q2)*cos(q3)*sin(q4)*sin(q5))/200 - (37*dq2*dqr4*sin(2*q4)*cos(q2)*sin(q3)*sin(q5))/1000 + (37*dq2*dqr4*sin(2*q4)*cos(q3)*sin(q2)*sin(q5))/1000 + (37*dq2*dqr5*sin(2*q4)*cos(q3)*sin(q2)*sin(q5))/4000 + (37*dq3*dqr4*sin(2*q4)*cos(q2)*sin(q3)*sin(q5))/1000 - (37*dq3*dqr4*sin(2*q4)*cos(q3)*sin(q2)*sin(q5))/1000 - (37*dq3*dqr5*sin(2*q4)*cos(q3)*sin(q2)*sin(q5))/4000 - (7*3^(1/2)*dq5*dqr3*cos(q2)*cos(q3)*sin(q5))/2000 + (7*3^(1/2)*dq2*dqr5*sin(q2)*sin(q3)*sin(q5))/2000 - (7*3^(1/2)*dq3*dqr5*sin(q2)*sin(q3)*sin(q5))/2000 + (117*dq1*dqr3*cos(2*q2)*cos(2*q3)*cos(q4)*sin(q5))/625 + (117*dq1*dqr3*sin(2*q2)*sin(2*q3)*cos(q4)*sin(q5))/625 - (117*dq1*dqr4*cos(2*q2)*sin(2*q3)*sin(q4)*sin(q5))/1250 + (117*dq1*dqr4*cos(2*q3)*sin(2*q2)*sin(q4)*sin(q5))/1250 - (29*3^(1/2)*dq1*dqr3*sin(2*q2)*cos(q3)*cos(q5))/400 - (7*dq2*dqr4*cos(q2)*cos(q4)*cos(q5)*sin(q3))/2000 + (7*dq2*dqr4*cos(q3)*cos(q4)*cos(q5)*sin(q2))/2000 + (7*dq3*dqr3*cos(q2)*cos(q3)*cos(q4)*sin(q5))/1000 + (7*dq2*dqr5*cos(q3)*cos(q4)*cos(q5)*sin(q2))/1000 + (7*dq3*dqr4*cos(q2)*cos(q4)*cos(q5)*sin(q3))/2000 - (7*dq3*dqr4*cos(q3)*cos(q4)*cos(q5)*sin(q2))/2000 - (7*dq3*dqr5*cos(q3)*cos(q4)*cos(q5)*sin(q2))/1000 + (7*dq4*dqr4*cos(q2)*cos(q3)*cos(q4)*sin(q5))/1000 + (7*dq4*dqr4*cos(q2)*cos(q3)*cos(q5)*sin(q4))/2000 - (117*dq4*dqr5*cos(q3)*cos(q4)*cos(q5)*sin(q2))/625 + (7*dq5*dqr4*cos(q2)*cos(q3)*cos(q4)*sin(q5))/2000 + (7*dq5*dqr4*cos(q2)*cos(q3)*cos(q5)*sin(q4))/1000 + (117*dq5*dqr4*cos(q2)*cos(q4)*cos(q5)*sin(q3))/625 - (117*dq5*dqr4*cos(q3)*cos(q4)*cos(q5)*sin(q2))/625 - dq1*dqr3*cos(2*q2)*sin(2*q3)*cos(q5)*((117*3^(1/2))/1250 + 37/4000) + dq1*dqr3*cos(2*q3)*sin(2*q2)*cos(q5)*((117*3^(1/2))/1250 + 37/4000) + (37*dq1*dqr3*cos(2*q2)*cos(2*q4)*sin(2*q3)*cos(q5))/4000 - (37*dq1*dqr3*cos(2*q3)*cos(2*q4)*sin(2*q2)*cos(q5))/4000 + (37*dq1*dqr4*cos(2*q2)*cos(2*q3)*cos(2*q4)*sin(q5))/2000 + (37*dq1*dqr4*cos(2*q2)*cos(2*q3)*sin(2*q4)*cos(q5))/4000 + (7*dq2*dqr4*cos(q2)*sin(q3)*sin(q4)*sin(q5))/1000 - (7*dq2*dqr4*cos(q3)*sin(q2)*sin(q4)*sin(q5))/1000 - (7*dq2*dqr5*cos(q3)*sin(q2)*sin(q4)*sin(q5))/2000 - (7*dq3*dqr4*cos(q2)*sin(q3)*sin(q4)*sin(q5))/1000 + (7*dq3*dqr4*cos(q3)*sin(q2)*sin(q4)*sin(q5))/1000 + (7*dq3*dqr5*cos(q3)*sin(q2)*sin(q4)*sin(q5))/2000 - (117*dq4*dqr4*cos(q2)*sin(q3)*sin(q4)*sin(q5))/625 + (117*dq4*dqr4*cos(q3)*sin(q2)*sin(q4)*sin(q5))/625 + (7*dq4*dqr4*cos(q4)*sin(q2)*sin(q3)*sin(q5))/1000 + (7*dq4*dqr4*cos(q5)*sin(q2)*sin(q3)*sin(q4))/2000 + (117*dq4*dqr5*cos(q3)*sin(q2)*sin(q4)*sin(q5))/1250 + (7*dq4*dqr5*cos(q4)*sin(q2)*sin(q3)*sin(q5))/2000 + (7*dq4*dqr5*cos(q5)*sin(q2)*sin(q3)*sin(q4))/1000 - (117*dq5*dqr4*cos(q2)*sin(q3)*sin(q4)*sin(q5))/1250 + (117*dq5*dqr4*cos(q3)*sin(q2)*sin(q4)*sin(q5))/1250 + (7*dq5*dqr4*cos(q4)*sin(q2)*sin(q3)*sin(q5))/2000 + (7*dq5*dqr4*cos(q5)*sin(q2)*sin(q3)*sin(q4))/1000 + (117*dq5*dqr5*cos(q3)*sin(q2)*sin(q4)*sin(q5))/625 + (7*dq5*dqr5*cos(q4)*sin(q2)*sin(q3)*sin(q5))/1000 + (7*dq5*dqr5*cos(q5)*sin(q2)*sin(q3)*sin(q4))/2000 - (37*dq1*dqr3*cos(2*q2)*sin(2*q3)*sin(2*q4)*sin(q5))/2000 + (37*dq1*dqr3*cos(2*q3)*sin(2*q2)*sin(2*q4)*sin(q5))/2000 + (37*dq1*dqr4*cos(2*q4)*sin(2*q2)*sin(2*q3)*sin(q5))/2000 + (37*dq1*dqr4*sin(2*q2)*sin(2*q3)*sin(2*q4)*cos(q5))/4000 - (29*dq1*dqr3*cos(2*q2)*cos(q3)*cos(q4)*sin(q5))/200 - (29*dq1*dqr4*cos(2*q2)*cos(q4)*cos(q5)*sin(q3))/400 + (29*dq1*dqr4*sin(2*q2)*cos(q3)*cos(q4)*cos(q5))/400 + (37*dq2*dqr3*cos(2*q4)*cos(q2)*cos(q3)*sin(q5))/1000 + (37*dq2*dqr3*sin(2*q4)*cos(q2)*cos(q3)*cos(q5))/2000 + (37*dq2*dqr4*cos(2*q4)*cos(q2)*cos(q5)*sin(q3))/2000 - (37*dq2*dqr4*cos(2*q4)*cos(q3)*cos(q5)*sin(q2))/2000 - (37*dq3*dqr3*cos(2*q4)*cos(q2)*cos(q3)*sin(q5))/1000 - (37*dq3*dqr3*sin(2*q4)*cos(q2)*cos(q3)*cos(q5))/2000 - (37*dq3*dqr4*cos(2*q4)*cos(q2)*cos(q5)*sin(q3))/2000 + (37*dq3*dqr4*cos(2*q4)*cos(q3)*cos(q5)*sin(q2))/2000 - (37*3^(1/2)*dq2*dqr5*cos(q4)*sin(q2)*sin(q3)*sin(q5))/2000 + (37*3^(1/2)*dq3*dqr5*cos(q4)*sin(q2)*sin(q3)*sin(q5))/2000 - dq1*dqr4*cos(2*q2)*sin(2*q3)*cos(q4)*cos(q5)*((37*3^(1/2))/4000 - 117/2500) + dq1*dqr4*cos(2*q3)*sin(2*q2)*cos(q4)*cos(q5)*((37*3^(1/2))/4000 - 117/2500) - dq4*dqr4*cos(q2)*cos(q4)*cos(q5)*sin(q3)*((37*3^(1/2))/2000 - 117/1250) + dq4*dqr4*cos(q3)*cos(q4)*cos(q5)*sin(q2)*((37*3^(1/2))/2000 - 117/1250) - dq5*dqr5*cos(q3)*cos(q4)*cos(q5)*sin(q2)*((37*3^(1/2))/2000 + 117/1250) + (37*3^(1/2)*dq5*dqr3*cos(q2)*cos(q3)*cos(q4)*sin(q5))/2000;
Y1_9_4=dq1*dqr5*sin(q5)*((117*3^(1/2))/2500 - 111/8000) - (37*dq1*dqr5*cos(2*q4)*sin(q5))/8000 - (37*dq1*dqr5*sin(2*q4)*cos(q5))/4000 + (29*ddqr1*cos(q4)*sin(q3)*sin(q5))/100 + (29*ddqr1*cos(q5)*sin(q3)*sin(q4))/200 + (37*ddqr4*cos(q5)*sin(q2)*sin(q3))/1000 + (29*ddqr4*cos(q4)*sin(q2)*sin(q5))/100 + (29*ddqr4*cos(q5)*sin(q2)*sin(q4))/200 + (37*ddqr5*cos(q5)*sin(q2)*sin(q3))/1000 + (29*ddqr5*cos(q4)*sin(q2)*sin(q5))/200 + (29*ddqr5*cos(q5)*sin(q2)*sin(q4))/100 + (7*dq1*dqr5*cos(q4)*sin(q5))/2000 + (7*dq1*dqr5*cos(q5)*sin(q4))/1000 - (7*ddqr2*cos(q2)*cos(q4)*sin(q3)*sin(q5))/1000 - (7*ddqr2*cos(q2)*cos(q5)*sin(q3)*sin(q4))/2000 + (7*ddqr2*cos(q3)*cos(q4)*sin(q2)*sin(q5))/1000 + (7*ddqr2*cos(q3)*cos(q5)*sin(q2)*sin(q4))/2000 + (7*ddqr3*cos(q2)*cos(q4)*sin(q3)*sin(q5))/1000 + (7*ddqr3*cos(q2)*cos(q5)*sin(q3)*sin(q4))/2000 - (7*ddqr3*cos(q3)*cos(q4)*sin(q2)*sin(q5))/1000 - (7*ddqr3*cos(q3)*cos(q5)*sin(q2)*sin(q4))/2000 + (117*ddqr4*cos(q2)*cos(q4)*sin(q3)*sin(q5))/625 - (117*ddqr4*cos(q3)*cos(q4)*sin(q2)*sin(q5))/625 - (7*ddqr4*cos(q4)*cos(q5)*sin(q2)*sin(q3))/2000 + (117*ddqr5*cos(q2)*cos(q5)*sin(q3)*sin(q4))/625 - (117*ddqr5*cos(q3)*cos(q5)*sin(q2)*sin(q4))/625 - (7*ddqr5*cos(q4)*cos(q5)*sin(q2)*sin(q3))/1000 - (29*3^(1/2)*dq1*dqr5*cos(q3)*sin(q5))/400 + (117*ddqr2*sin(q2)*sin(q3)*sin(q4)*sin(q5))/625 - (117*ddqr3*sin(q2)*sin(q3)*sin(q4)*sin(q5))/625 + (7*ddqr4*sin(q2)*sin(q3)*sin(q4)*sin(q5))/1000 + (7*ddqr5*sin(q2)*sin(q3)*sin(q4)*sin(q5))/2000 - (29*ddqr1*cos(2*q2)*cos(q4)*sin(q3)*sin(q5))/100 - (29*ddqr1*cos(2*q2)*cos(q5)*sin(q3)*sin(q4))/200 + (37*ddqr2*cos(2*q4)*cos(q2)*sin(q3)*sin(q5))/1000 - (37*ddqr2*cos(2*q4)*cos(q3)*sin(q2)*sin(q5))/1000 - (37*ddqr2*sin(2*q4)*cos(q3)*cos(q5)*sin(q2))/2000 - (37*ddqr3*cos(2*q4)*cos(q2)*sin(q3)*sin(q5))/1000 + (37*ddqr3*cos(2*q4)*cos(q3)*sin(q2)*sin(q5))/1000 + (37*ddqr3*sin(2*q4)*cos(q3)*cos(q5)*sin(q2))/2000 + (37*dq2*dqr5*cos(q2)*cos(q5)*sin(q3))/2000 - (37*dq2*dqr5*cos(q3)*cos(q5)*sin(q2))/2000 + (29*dq1*dqr5*cos(q4)*cos(q5)*sin(q3))/200 - (37*dq3*dqr5*cos(q2)*cos(q5)*sin(q3))/2000 + (37*dq3*dqr5*cos(q3)*cos(q5)*sin(q2))/2000 - (37*dq4*dqr5*cos(q2)*cos(q3)*sin(q5))/2000 + (29*dq4*dqr5*cos(q4)*cos(q5)*sin(q2))/100 - (37*dq5*dqr5*cos(q2)*cos(q3)*sin(q5))/1000 + (29*dq5*dqr5*cos(q4)*cos(q5)*sin(q2))/200 - (7*3^(1/2)*ddqr2*cos(q5)*sin(q2)*sin(q3))/2000 + (7*3^(1/2)*ddqr3*cos(q5)*sin(q2)*sin(q3))/2000 - (7*3^(1/2)*ddqr5*cos(q2)*sin(q3)*sin(q5))/2000 + (7*3^(1/2)*ddqr5*cos(q3)*sin(q2)*sin(q5))/2000 - (29*dq1*dqr5*sin(q3)*sin(q4)*sin(q5))/400 + (29*dq1*dqr5*cos(2*q2)*sin(q3)*sin(q4)*sin(q5))/400 - (29*dq1*dqr5*sin(2*q2)*cos(q3)*sin(q4)*sin(q5))/400 - (37*dq2*dqr5*sin(2*q4)*cos(q2)*sin(q3)*sin(q5))/4000 + (37*dq3*dqr5*sin(2*q4)*cos(q2)*sin(q3)*sin(q5))/4000 + (7*3^(1/2)*dq2*dqr5*cos(q2)*cos(q3)*sin(q5))/2000 - (7*3^(1/2)*dq3*dqr5*cos(q2)*cos(q3)*sin(q5))/2000 - (7*3^(1/2)*dq5*dqr5*cos(q2)*cos(q5)*sin(q3))/2000 + (7*3^(1/2)*dq5*dqr5*cos(q3)*cos(q5)*sin(q2))/2000 + (117*dq1*dqr5*cos(2*q2)*sin(2*q3)*cos(q4)*cos(q5))/1250 - (117*dq1*dqr5*cos(2*q3)*sin(2*q2)*cos(q4)*cos(q5))/1250 + ddqr2*cos(q4)*cos(q5)*sin(q2)*sin(q3)*((37*3^(1/2))/2000 - 117/1250) - ddqr3*cos(q4)*cos(q5)*sin(q2)*sin(q3)*((37*3^(1/2))/2000 - 117/1250) - ddqr4*cos(q2)*cos(q5)*sin(q3)*sin(q4)*((37*3^(1/2))/2000 - 117/1250) + ddqr4*cos(q3)*cos(q5)*sin(q2)*sin(q4)*((37*3^(1/2))/2000 - 117/1250) + ddqr5*cos(q2)*cos(q4)*sin(q3)*sin(q5)*((37*3^(1/2))/2000 + 117/1250) - ddqr5*cos(q3)*cos(q4)*sin(q2)*sin(q5)*((37*3^(1/2))/2000 + 117/1250) + (29*3^(1/2)*dq1*dqr5*cos(2*q2)*cos(q3)*sin(q5))/400 - (7*dq2*dqr5*cos(q2)*cos(q4)*cos(q5)*sin(q3))/1000 + (7*dq3*dqr5*cos(q2)*cos(q4)*cos(q5)*sin(q3))/1000 + (7*dq4*dqr5*cos(q2)*cos(q3)*cos(q4)*sin(q5))/2000 + (7*dq4*dqr5*cos(q2)*cos(q3)*cos(q5)*sin(q4))/1000 + (117*dq4*dqr5*cos(q2)*cos(q4)*cos(q5)*sin(q3))/625 + (7*dq5*dqr5*cos(q2)*cos(q3)*cos(q4)*sin(q5))/1000 + (7*dq5*dqr5*cos(q2)*cos(q3)*cos(q5)*sin(q4))/2000 - dq1*dqr5*cos(2*q2)*cos(2*q3)*sin(q5)*((117*3^(1/2))/2500 + 37/8000) + (29*3^(1/2)*dq1*dqr5*sin(2*q2)*sin(q3)*sin(q5))/400 + (37*dq1*dqr5*cos(2*q2)*cos(2*q3)*cos(2*q4)*sin(q5))/8000 + (37*dq1*dqr5*cos(2*q2)*cos(2*q3)*sin(2*q4)*cos(q5))/4000 + (7*dq2*dqr5*cos(q2)*sin(q3)*sin(q4)*sin(q5))/2000 - (7*dq3*dqr5*cos(q2)*sin(q3)*sin(q4)*sin(q5))/2000 - (117*dq4*dqr5*cos(q2)*sin(q3)*sin(q4)*sin(q5))/1250 - (117*dq5*dqr5*cos(q2)*sin(q3)*sin(q4)*sin(q5))/625 - dq1*dqr5*sin(2*q2)*sin(2*q3)*sin(q5)*((117*3^(1/2))/2500 + 37/8000) + (37*dq1*dqr5*cos(2*q4)*sin(2*q2)*sin(2*q3)*sin(q5))/8000 + (37*dq1*dqr5*sin(2*q2)*sin(2*q3)*sin(2*q4)*cos(q5))/4000 - (29*dq1*dqr5*cos(2*q2)*cos(q4)*cos(q5)*sin(q3))/200 + (29*dq1*dqr5*sin(2*q2)*cos(q3)*cos(q4)*cos(q5))/200 + (37*dq2*dqr5*cos(2*q4)*cos(q2)*cos(q5)*sin(q3))/2000 - (37*dq2*dqr5*cos(2*q4)*cos(q3)*cos(q5)*sin(q2))/2000 - (37*dq3*dqr5*cos(2*q4)*cos(q2)*cos(q5)*sin(q3))/2000 + (37*dq3*dqr5*cos(2*q4)*cos(q3)*cos(q5)*sin(q2))/2000 + dq1*dqr5*cos(2*q2)*sin(2*q3)*sin(q4)*sin(q5)*((37*3^(1/2))/4000 - 117/2500) - dq1*dqr5*cos(2*q3)*sin(2*q2)*sin(q4)*sin(q5)*((37*3^(1/2))/4000 - 117/2500) + dq5*dqr5*cos(q2)*cos(q4)*cos(q5)*sin(q3)*((37*3^(1/2))/2000 + 117/1250) - (37*3^(1/2)*dq2*dqr5*cos(q2)*cos(q3)*cos(q4)*sin(q5))/2000 + (37*3^(1/2)*dq3*dqr5*cos(q2)*cos(q3)*cos(q4)*sin(q5))/2000;
Y1_9_5=(7*ddqr1*sin(q4)*sin(q5))/500 - (7*ddqr1*cos(q4)*cos(q5))/1000 - ddqr1*cos(q5)*((117*3^(1/2))/1250 - 111/4000) + (37*ddqr1*cos(2*q4)*cos(q5))/4000 - (37*ddqr1*sin(2*q4)*sin(q5))/2000 + (29*ddqr2*cos(q2)*cos(q4)*cos(q5))/200 + (37*ddqr4*cos(q2)*cos(q3)*cos(q5))/1000 + (37*ddqr5*cos(q2)*cos(q3)*cos(q5))/1000 - (29*ddqr2*cos(q2)*sin(q4)*sin(q5))/100 + (29*3^(1/2)*ddqr1*cos(q3)*cos(q5))/200 - (7*ddqr4*cos(q2)*cos(q3)*cos(q4)*cos(q5))/2000 - (7*ddqr5*cos(q2)*cos(q3)*cos(q4)*cos(q5))/1000 + ddqr1*cos(2*q2)*cos(2*q3)*cos(q5)*((117*3^(1/2))/1250 + 37/4000) - (29*3^(1/2)*ddqr1*sin(2*q2)*cos(q5)*sin(q3))/200 - (37*ddqr1*cos(2*q2)*cos(2*q3)*cos(2*q4)*cos(q5))/4000 + (117*ddqr2*cos(q2)*cos(q3)*sin(q4)*sin(q5))/625 - (117*ddqr3*cos(q2)*cos(q3)*sin(q4)*sin(q5))/625 + (7*ddqr4*cos(q2)*cos(q3)*sin(q4)*sin(q5))/1000 + (7*ddqr5*cos(q2)*cos(q3)*sin(q4)*sin(q5))/2000 + ddqr1*sin(2*q2)*sin(2*q3)*cos(q5)*((117*3^(1/2))/1250 + 37/4000) + (37*ddqr1*cos(2*q2)*cos(2*q3)*sin(2*q4)*sin(q5))/2000 - (37*ddqr1*cos(2*q4)*sin(2*q2)*sin(2*q3)*cos(q5))/4000 + (37*ddqr1*sin(2*q2)*sin(2*q3)*sin(2*q4)*sin(q5))/2000 + (29*ddqr1*sin(2*q2)*cos(q3)*cos(q4)*sin(q5))/100 + (29*ddqr1*sin(2*q2)*cos(q3)*cos(q5)*sin(q4))/200 + (37*ddqr2*sin(2*q4)*cos(q2)*cos(q5)*sin(q3))/2000 - (37*ddqr3*sin(2*q4)*cos(q2)*cos(q5)*sin(q3))/2000 - (7*3^(1/2)*ddqr2*cos(q2)*cos(q3)*cos(q5))/2000 + (7*3^(1/2)*ddqr3*cos(q2)*cos(q3)*cos(q5))/2000 + (117*ddqr1*cos(2*q2)*sin(2*q3)*cos(q4)*sin(q5))/625 - (117*ddqr1*cos(2*q3)*sin(2*q2)*cos(q4)*sin(q5))/625 - (29*3^(1/2)*ddqr1*cos(2*q2)*cos(q3)*cos(q5))/200 - ddqr1*cos(2*q2)*sin(2*q3)*cos(q5)*sin(q4)*((37*3^(1/2))/2000 - 117/1250) + ddqr1*cos(2*q3)*sin(2*q2)*cos(q5)*sin(q4)*((37*3^(1/2))/2000 - 117/1250) + ddqr2*cos(q2)*cos(q3)*cos(q4)*cos(q5)*((37*3^(1/2))/2000 - 117/1250) - ddqr3*cos(q2)*cos(q3)*cos(q4)*cos(q5)*((37*3^(1/2))/2000 - 117/1250);
Y1_10_1=(7*dq4*dqr1*sin(q4)*sin(q5)*sin(q6))/2000 - (87*dq3*dqr1*cos(q3)*cos(q6)*sin(q4))/800 - (87*dq4*dqr1*cos(q4)*cos(q6)*sin(q3))/800 - (29*3^(1/2)*dq3*dqr1*cos(q6)*sin(q3))/800 + (87*dq6*dqr1*sin(q3)*sin(q4)*sin(q6))/800 + (7*dq5*dqr1*sin(q4)*sin(q5)*sin(q6))/1000 + (7*dq6*dqr1*sin(q4)*sin(q5)*sin(q6))/2000 - (87*dq2*dqr1*sin(2*q2)*cos(q6)*sin(q3)*sin(q4))/400 + (87*dq3*dqr1*sin(2*q2)*cos(q6)*sin(q3)*sin(q4))/800 - (87*dq6*dqr1*cos(2*q2)*sin(q3)*sin(q4)*sin(q6))/800 + (87*dq6*dqr1*sin(2*q2)*cos(q3)*sin(q4)*sin(q6))/800 + (29*3^(1/2)*dq3*dqr1*cos(q5)*cos(q6)*sin(q3))/800 - (29*3^(1/2)*dq3*dqr1*sin(q3)*sin(q5)*sin(q6))/400 - (29*3^(1/2)*dq2*dqr1*cos(2*q2)*cos(q6)*sin(q3))/400 + (29*3^(1/2)*dq3*dqr1*cos(2*q2)*cos(q6)*sin(q3))/800 - (29*dq3*dqr1*cos(q3)*cos(q5)*cos(q6)*sin(q4))/800 - (29*dq4*dqr1*cos(q4)*cos(q5)*cos(q6)*sin(q3))/800 - (29*dq5*dqr1*cos(q4)*cos(q5)*cos(q6)*sin(q3))/400 - (29*dq6*dqr1*cos(q4)*cos(q5)*cos(q6)*sin(q3))/200 + (29*3^(1/2)*dq6*dqr1*sin(2*q2)*sin(q3)*sin(q6))/800 + (29*dq3*dqr1*cos(q3)*sin(q4)*sin(q5)*sin(q6))/400 + (29*dq4*dqr1*cos(q4)*sin(q3)*sin(q5)*sin(q6))/400 + (29*dq4*dqr1*cos(q5)*sin(q3)*sin(q4)*sin(q6))/200 + (29*dq4*dqr1*cos(q6)*sin(q3)*sin(q4)*sin(q5))/400 + (29*dq5*dqr1*cos(q4)*sin(q3)*sin(q5)*sin(q6))/200 + (29*dq5*dqr1*cos(q5)*sin(q3)*sin(q4)*sin(q6))/400 + (29*dq5*dqr1*cos(q6)*sin(q3)*sin(q4)*sin(q5))/800 + (29*dq6*dqr1*cos(q4)*sin(q3)*sin(q5)*sin(q6))/400 + (29*dq6*dqr1*cos(q5)*sin(q3)*sin(q4)*sin(q6))/800 + (29*dq6*dqr1*cos(q6)*sin(q3)*sin(q4)*sin(q5))/400 - (87*dq2*dqr1*cos(2*q2)*cos(q3)*cos(q6)*sin(q4))/400 + (87*dq3*dqr1*cos(2*q2)*cos(q3)*cos(q6)*sin(q4))/800 + (87*dq4*dqr1*cos(2*q2)*cos(q4)*cos(q6)*sin(q3))/800 + (1231*dq2*dqr1*sin(2*q2)*sin(2*q3)*cos(q5)*cos(q6)*sin(q4))/40000 + (877*dq4*dqr1*cos(2*q2)*sin(2*q3)*cos(q5)*sin(q4)*sin(q6))/8000 - (877*dq4*dqr1*cos(2*q3)*sin(2*q2)*cos(q5)*sin(q4)*sin(q6))/8000 + (1231*dq5*dqr1*cos(2*q2)*sin(2*q3)*cos(q6)*sin(q4)*sin(q5))/80000 - (1231*dq5*dqr1*cos(2*q3)*sin(2*q2)*cos(q6)*sin(q4)*sin(q5))/80000 + (1231*dq6*dqr1*cos(2*q2)*sin(2*q3)*cos(q5)*sin(q4)*sin(q6))/80000 - (1231*dq6*dqr1*cos(2*q3)*sin(2*q2)*cos(q5)*sin(q4)*sin(q6))/80000 + (29*3^(1/2)*dq2*dqr1*cos(2*q2)*cos(q5)*cos(q6)*sin(q3))/400 - (29*3^(1/2)*dq3*dqr1*cos(2*q2)*cos(q5)*cos(q6)*sin(q3))/800 - (29*3^(1/2)*dq2*dqr1*cos(2*q2)*sin(q3)*sin(q5)*sin(q6))/200 + (29*3^(1/2)*dq3*dqr1*cos(2*q2)*sin(q3)*sin(q5)*sin(q6))/400 - (29*3^(1/2)*dq5*dqr1*sin(2*q2)*cos(q5)*sin(q3)*sin(q6))/400 - (29*3^(1/2)*dq5*dqr1*sin(2*q2)*cos(q6)*sin(q3)*sin(q5))/800 - (29*3^(1/2)*dq6*dqr1*sin(2*q2)*cos(q5)*sin(q3)*sin(q6))/800 - (29*3^(1/2)*dq6*dqr1*sin(2*q2)*cos(q6)*sin(q3)*sin(q5))/400 + dq6*dqr1*cos(2*q2)*sin(2*q3)*sin(q4)*sin(q6)*((111*3^(1/2))/16000 + 7539/80000) - dq6*dqr1*cos(2*q3)*sin(2*q2)*sin(q4)*sin(q6)*((111*3^(1/2))/16000 + 7539/80000) - (29*dq2*dqr1*cos(2*q2)*cos(q3)*cos(q5)*cos(q6)*sin(q4))/400 + (29*dq3*dqr1*cos(2*q2)*cos(q3)*cos(q5)*cos(q6)*sin(q4))/800 + (29*dq4*dqr1*cos(2*q2)*cos(q4)*cos(q5)*cos(q6)*sin(q3))/800 + (29*dq5*dqr1*cos(2*q2)*cos(q4)*cos(q5)*cos(q6)*sin(q3))/400 + (29*dq6*dqr1*cos(2*q2)*cos(q4)*cos(q5)*cos(q6)*sin(q3))/200 + (29*dq2*dqr1*cos(2*q2)*cos(q3)*sin(q4)*sin(q5)*sin(q6))/200 - (29*dq2*dqr1*sin(2*q2)*cos(q4)*cos(q5)*sin(q3)*sin(q6))/100 - (29*dq2*dqr1*sin(2*q2)*cos(q4)*cos(q6)*sin(q3)*sin(q5))/200 - (29*dq2*dqr1*sin(2*q2)*cos(q5)*cos(q6)*sin(q3)*sin(q4))/400 - (29*dq3*dqr1*cos(2*q2)*cos(q3)*sin(q4)*sin(q5)*sin(q6))/400 + (29*dq3*dqr1*sin(2*q2)*cos(q4)*cos(q5)*sin(q3)*sin(q6))/200 + (29*dq3*dqr1*sin(2*q2)*cos(q4)*cos(q6)*sin(q3)*sin(q5))/400 + (29*dq3*dqr1*sin(2*q2)*cos(q5)*cos(q6)*sin(q3)*sin(q4))/800 - (29*dq4*dqr1*cos(2*q2)*cos(q4)*sin(q3)*sin(q5)*sin(q6))/400 - (29*dq4*dqr1*cos(2*q2)*cos(q5)*sin(q3)*sin(q4)*sin(q6))/200 - (29*dq4*dqr1*cos(2*q2)*cos(q6)*sin(q3)*sin(q4)*sin(q5))/400 + (29*dq4*dqr1*sin(2*q2)*cos(q3)*cos(q5)*sin(q4)*sin(q6))/200 + (29*dq4*dqr1*sin(2*q2)*cos(q3)*cos(q6)*sin(q4)*sin(q5))/400 - (29*dq5*dqr1*cos(2*q2)*cos(q4)*sin(q3)*sin(q5)*sin(q6))/200 - (29*dq5*dqr1*cos(2*q2)*cos(q5)*sin(q3)*sin(q4)*sin(q6))/400 - (29*dq5*dqr1*cos(2*q2)*cos(q6)*sin(q3)*sin(q4)*sin(q5))/800 + (29*dq5*dqr1*sin(2*q2)*cos(q3)*cos(q5)*sin(q4)*sin(q6))/400 + (29*dq5*dqr1*sin(2*q2)*cos(q3)*cos(q6)*sin(q4)*sin(q5))/800 - (29*dq6*dqr1*cos(2*q2)*cos(q4)*sin(q3)*sin(q5)*sin(q6))/400 - (29*dq6*dqr1*cos(2*q2)*cos(q5)*sin(q3)*sin(q4)*sin(q6))/800 - (29*dq6*dqr1*cos(2*q2)*cos(q6)*sin(q3)*sin(q4)*sin(q5))/400 + (29*dq6*dqr1*sin(2*q2)*cos(q3)*cos(q5)*sin(q4)*sin(q6))/800 + (29*dq6*dqr1*sin(2*q2)*cos(q3)*cos(q6)*sin(q4)*sin(q5))/400 + (29*dq2*dqr1*sin(2*q2)*sin(q3)*sin(q4)*sin(q5)*sin(q6))/200 - (29*dq3*dqr1*sin(2*q2)*sin(q3)*sin(q4)*sin(q5)*sin(q6))/400 - (37*3^(1/2)*dq2*dqr1*sin(2*q2)*sin(2*q3)*sin(2*q5)*sin(q4)*sin(q6))/4000 + (37*3^(1/2)*dq3*dqr1*sin(2*q2)*sin(2*q3)*sin(2*q5)*sin(q4)*sin(q6))/4000 + dq2*dqr1*cos(2*q2)*cos(2*q3)*sin(q4)*sin(q5)*sin(q6)*((37*3^(1/2))/2000 - 1231/20000) - dq3*dqr1*cos(2*q2)*cos(2*q3)*sin(q4)*sin(q5)*sin(q6)*((37*3^(1/2))/2000 - 1231/20000) - dq4*dqr1*cos(2*q2)*sin(2*q3)*cos(q6)*sin(q4)*sin(q5)*((37*3^(1/2))/8000 - 877/16000) + dq4*dqr1*cos(2*q3)*sin(2*q2)*cos(q6)*sin(q4)*sin(q5)*((37*3^(1/2))/8000 - 877/16000) - dq5*dqr1*cos(2*q2)*sin(2*q3)*cos(q5)*sin(q4)*sin(q6)*((37*3^(1/2))/4000 - 1231/40000) + dq5*dqr1*cos(2*q3)*sin(2*q2)*cos(q5)*sin(q4)*sin(q6)*((37*3^(1/2))/4000 - 1231/40000) - dq6*dqr1*cos(2*q2)*sin(2*q3)*cos(q6)*sin(q4)*sin(q5)*((37*3^(1/2))/4000 - 1231/40000) + dq6*dqr1*cos(2*q3)*sin(2*q2)*cos(q6)*sin(q4)*sin(q5)*((37*3^(1/2))/4000 - 1231/40000) + dq2*dqr1*sin(2*q2)*sin(2*q3)*sin(q4)*sin(q5)*sin(q6)*((37*3^(1/2))/2000 - 1231/20000) - dq3*dqr1*sin(2*q2)*sin(2*q3)*sin(q4)*sin(q5)*sin(q6)*((37*3^(1/2))/2000 - 1231/20000) - (37*3^(1/2)*dq2*dqr1*cos(2*q2)*cos(2*q3)*sin(2*q5)*sin(q4)*sin(q6))/4000 + (37*3^(1/2)*dq3*dqr1*cos(2*q2)*cos(2*q3)*sin(2*q5)*sin(q4)*sin(q6))/4000 + (37*3^(1/2)*dq4*dqr1*cos(2*q2)*cos(2*q5)*sin(2*q3)*sin(q4)*sin(q6))/4000 - (37*3^(1/2)*dq4*dqr1*cos(2*q3)*cos(2*q5)*sin(2*q2)*sin(q4)*sin(q6))/4000 + (37*3^(1/2)*dq5*dqr1*cos(2*q2)*cos(2*q5)*sin(2*q3)*sin(q4)*sin(q6))/4000 - (37*3^(1/2)*dq5*dqr1*cos(2*q3)*cos(2*q5)*sin(2*q2)*sin(q4)*sin(q6))/4000 + (37*3^(1/2)*dq6*dqr1*cos(2*q2)*cos(2*q5)*sin(2*q3)*sin(q4)*sin(q6))/16000 - (37*3^(1/2)*dq6*dqr1*cos(2*q3)*cos(2*q5)*sin(2*q2)*sin(q4)*sin(q6))/16000;
Y1_10_2=(29*3^(1/2)*dq5*dqr1*cos(q3)*cos(q5)*sin(q6))/400 - (29*3^(1/2)*dq6*dqr1*cos(q3)*sin(q6))/800 - (7*dq4*dqr1*cos(q4)*cos(q5)*sin(q6))/1000 - (7*dq4*dqr1*cos(q4)*cos(q6)*sin(q5))/2000 - (7*dq4*dqr1*cos(q5)*cos(q6)*sin(q4))/4000 - (7*dq5*dqr1*cos(q4)*cos(q5)*sin(q6))/2000 - (7*dq5*dqr1*cos(q4)*cos(q6)*sin(q5))/4000 - (7*dq5*dqr1*cos(q5)*cos(q6)*sin(q4))/2000 - (7*dq6*dqr1*cos(q4)*cos(q5)*sin(q6))/4000 - (7*dq6*dqr1*cos(q4)*cos(q6)*sin(q5))/2000 - (7*dq6*dqr1*cos(q5)*cos(q6)*sin(q4))/1000 - dq6*dqr1*cos(q6)*sin(q5)*((6847*3^(1/2))/160000 - 111/8000) - dq5*dqr1*cos(q6)*sin(q5)*((6847*3^(1/2))/320000 - 111/32000) - (21*dq4*dqr1*cos(q6)*sin(q4))/4000 + (29*3^(1/2)*dq5*dqr1*cos(q3)*cos(q6)*sin(q5))/800 + (29*3^(1/2)*dq6*dqr1*cos(q3)*cos(q5)*sin(q6))/800 + (29*3^(1/2)*dq6*dqr1*cos(q3)*cos(q6)*sin(q5))/400 + dq4*dqr1*cos(2*q4)*cos(q6)*sin(q5)*((641*3^(1/2))/80000 - 37/8000) + dq6*dqr1*cos(2*q4)*cos(q6)*sin(q5)*((641*3^(1/2))/160000 + 37/8000) + dq5*dqr1*cos(2*q4)*cos(q6)*sin(q5)*((641*3^(1/2))/320000 - 37/32000) - dq4*dqr1*sin(2*q4)*sin(q5)*sin(q6)*((641*3^(1/2))/80000 + 37/4000) - dq5*dqr1*sin(2*q4)*sin(q5)*sin(q6)*((641*3^(1/2))/80000 + 37/4000) - dq6*dqr1*sin(2*q4)*sin(q5)*sin(q6)*((641*3^(1/2))/160000 - 37/16000) + (29*3^(1/2)*dq6*dqr1*cos(2*q2)*cos(q3)*sin(q6))/800 - (29*dq3*dqr1*cos(q3)*cos(q4)*cos(q5)*sin(q6))/200 - (29*dq3*dqr1*cos(q3)*cos(q4)*cos(q6)*sin(q5))/400 + (877*dq2*dqr1*cos(2*q2)*cos(2*q3)*cos(q4)*cos(q5)*sin(q6))/4000 + (1231*dq2*dqr1*cos(2*q2)*cos(2*q3)*cos(q5)*cos(q6)*sin(q4))/40000 - (877*dq3*dqr1*cos(2*q2)*cos(2*q3)*cos(q4)*cos(q5)*sin(q6))/4000 - (1231*dq3*dqr1*cos(2*q2)*cos(2*q3)*cos(q5)*cos(q6)*sin(q4))/40000 + (877*dq2*dqr1*sin(2*q2)*sin(2*q3)*cos(q4)*cos(q5)*sin(q6))/4000 - (877*dq3*dqr1*sin(2*q2)*sin(2*q3)*cos(q4)*cos(q5)*sin(q6))/4000 - (1231*dq3*dqr1*sin(2*q2)*sin(2*q3)*cos(q5)*cos(q6)*sin(q4))/40000 + (877*dq5*dqr1*cos(2*q2)*sin(2*q3)*cos(q4)*sin(q5)*sin(q6))/8000 - (877*dq5*dqr1*cos(2*q3)*sin(2*q2)*cos(q4)*sin(q5)*sin(q6))/8000 - (29*3^(1/2)*dq5*dqr1*cos(2*q2)*cos(q3)*cos(q5)*sin(q6))/400 - (29*3^(1/2)*dq5*dqr1*cos(2*q2)*cos(q3)*cos(q6)*sin(q5))/800 - (29*3^(1/2)*dq6*dqr1*cos(2*q2)*cos(q3)*cos(q5)*sin(q6))/800 - (29*3^(1/2)*dq6*dqr1*cos(2*q2)*cos(q3)*cos(q6)*sin(q5))/400 + dq2*dqr1*cos(2*q2)*cos(2*q3)*cos(q6)*sin(q4)*((111*3^(1/2))/8000 + 7539/40000) - dq3*dqr1*cos(2*q2)*cos(2*q3)*cos(q6)*sin(q4)*((111*3^(1/2))/8000 + 7539/40000) + dq6*dqr1*cos(2*q2)*cos(2*q3)*cos(q6)*sin(q5)*((9411*3^(1/2))/160000 + 37/8000) + dq5*dqr1*cos(2*q2)*cos(2*q3)*cos(q6)*sin(q5)*((9411*3^(1/2))/320000 - 259/32000) + (29*3^(1/2)*dq2*dqr1*sin(2*q2)*cos(q3)*sin(q5)*sin(q6))/200 - (29*3^(1/2)*dq3*dqr1*sin(2*q2)*cos(q3)*sin(q5)*sin(q6))/400 + dq2*dqr1*sin(2*q2)*sin(2*q3)*cos(q6)*sin(q4)*((111*3^(1/2))/8000 + 7539/40000) - dq3*dqr1*sin(2*q2)*sin(2*q3)*cos(q6)*sin(q4)*((111*3^(1/2))/8000 + 7539/40000) + dq2*dqr1*cos(2*q2)*sin(2*q3)*sin(q5)*sin(q6)*((9411*3^(1/2))/80000 + 37/4000) - dq2*dqr1*cos(2*q3)*sin(2*q2)*sin(q5)*sin(q6)*((9411*3^(1/2))/80000 + 37/4000) - dq3*dqr1*cos(2*q2)*sin(2*q3)*sin(q5)*sin(q6)*((9411*3^(1/2))/80000 + 37/4000) + dq3*dqr1*cos(2*q3)*sin(2*q2)*sin(q5)*sin(q6)*((9411*3^(1/2))/80000 + 37/4000) + dq6*dqr1*sin(2*q2)*sin(2*q3)*cos(q6)*sin(q5)*((9411*3^(1/2))/160000 + 37/8000) + dq5*dqr1*sin(2*q2)*sin(2*q3)*cos(q6)*sin(q5)*((9411*3^(1/2))/320000 - 259/32000) - (29*dq2*dqr1*cos(2*q2)*cos(q3)*cos(q4)*cos(q5)*sin(q6))/100 - (29*dq2*dqr1*cos(2*q2)*cos(q3)*cos(q4)*cos(q6)*sin(q5))/200 + (29*dq3*dqr1*cos(2*q2)*cos(q3)*cos(q4)*cos(q5)*sin(q6))/200 + (29*dq3*dqr1*cos(2*q2)*cos(q3)*cos(q4)*cos(q6)*sin(q5))/400 + (29*dq4*dqr1*sin(2*q2)*cos(q3)*cos(q4)*sin(q5)*sin(q6))/400 + (29*dq5*dqr1*sin(2*q2)*cos(q3)*cos(q4)*sin(q5)*sin(q6))/200 + (29*dq6*dqr1*sin(2*q2)*cos(q3)*cos(q4)*sin(q5)*sin(q6))/400 - dq2*dqr1*cos(2*q2)*cos(2*q3)*cos(q4)*cos(q6)*sin(q5)*((37*3^(1/2))/4000 - 877/8000) + dq3*dqr1*cos(2*q2)*cos(2*q3)*cos(q4)*cos(q6)*sin(q5)*((37*3^(1/2))/4000 - 877/8000) - dq2*dqr1*sin(2*q2)*sin(2*q3)*cos(q4)*cos(q6)*sin(q5)*((37*3^(1/2))/4000 - 877/8000) + dq3*dqr1*sin(2*q2)*sin(2*q3)*cos(q4)*cos(q6)*sin(q5)*((37*3^(1/2))/4000 - 877/8000) - dq6*dqr1*cos(2*q2)*sin(2*q3)*cos(q4)*sin(q5)*sin(q6)*((37*3^(1/2))/8000 - 877/16000) + dq6*dqr1*cos(2*q3)*sin(2*q2)*cos(q4)*sin(q5)*sin(q6)*((37*3^(1/2))/8000 - 877/16000) - dq4*dqr1*cos(2*q2)*sin(2*q3)*cos(q4)*sin(q5)*sin(q6)*((37*3^(1/2))/4000 - 1231/40000) + dq4*dqr1*cos(2*q3)*sin(2*q2)*cos(q4)*sin(q5)*sin(q6)*((37*3^(1/2))/4000 - 1231/40000) - dq4*dqr1*cos(2*q2)*cos(2*q3)*cos(2*q4)*cos(q6)*sin(q5)*((641*3^(1/2))/80000 - 37/8000) - dq6*dqr1*cos(2*q2)*cos(2*q3)*cos(2*q4)*cos(q6)*sin(q5)*((641*3^(1/2))/160000 + 37/8000) - dq5*dqr1*cos(2*q2)*cos(2*q3)*cos(2*q4)*cos(q6)*sin(q5)*((641*3^(1/2))/320000 - 37/32000) - dq2*dqr1*cos(2*q2)*cos(2*q4)*sin(2*q3)*sin(q5)*sin(q6)*((641*3^(1/2))/80000 + 37/4000) + dq2*dqr1*cos(2*q3)*cos(2*q4)*sin(2*q2)*sin(q5)*sin(q6)*((641*3^(1/2))/80000 + 37/4000) + dq3*dqr1*cos(2*q2)*cos(2*q4)*sin(2*q3)*sin(q5)*sin(q6)*((641*3^(1/2))/80000 + 37/4000) - dq3*dqr1*cos(2*q3)*cos(2*q4)*sin(2*q2)*sin(q5)*sin(q6)*((641*3^(1/2))/80000 + 37/4000) + dq4*dqr1*cos(2*q2)*cos(2*q3)*sin(2*q4)*sin(q5)*sin(q6)*((641*3^(1/2))/80000 + 37/4000) + dq5*dqr1*cos(2*q2)*cos(2*q3)*sin(2*q4)*sin(q5)*sin(q6)*((641*3^(1/2))/80000 + 37/4000) - dq2*dqr1*cos(2*q2)*sin(2*q3)*sin(2*q4)*cos(q6)*sin(q5)*((641*3^(1/2))/80000 - 37/8000) + dq2*dqr1*cos(2*q3)*sin(2*q2)*sin(2*q4)*cos(q6)*sin(q5)*((641*3^(1/2))/80000 - 37/8000) + dq3*dqr1*cos(2*q2)*sin(2*q3)*sin(2*q4)*cos(q6)*sin(q5)*((641*3^(1/2))/80000 - 37/8000) - dq3*dqr1*cos(2*q3)*sin(2*q2)*sin(2*q4)*cos(q6)*sin(q5)*((641*3^(1/2))/80000 - 37/8000) - dq4*dqr1*cos(2*q4)*sin(2*q2)*sin(2*q3)*cos(q6)*sin(q5)*((641*3^(1/2))/80000 - 37/8000) - dq6*dqr1*cos(2*q4)*sin(2*q2)*sin(2*q3)*cos(q6)*sin(q5)*((641*3^(1/2))/160000 + 37/8000) + dq6*dqr1*cos(2*q2)*cos(2*q3)*sin(2*q4)*sin(q5)*sin(q6)*((641*3^(1/2))/160000 - 37/16000) - dq5*dqr1*cos(2*q4)*sin(2*q2)*sin(2*q3)*cos(q6)*sin(q5)*((641*3^(1/2))/320000 - 37/32000) + dq4*dqr1*sin(2*q2)*sin(2*q3)*sin(2*q4)*sin(q5)*sin(q6)*((641*3^(1/2))/80000 + 37/4000) + dq5*dqr1*sin(2*q2)*sin(2*q3)*sin(2*q4)*sin(q5)*sin(q6)*((641*3^(1/2))/80000 + 37/4000) + dq6*dqr1*sin(2*q2)*sin(2*q3)*sin(2*q4)*sin(q5)*sin(q6)*((641*3^(1/2))/160000 - 37/16000) + (37*3^(1/2)*dq2*dqr1*cos(2*q2)*cos(2*q3)*cos(2*q5)*cos(q4)*sin(q6))/2000 + (37*3^(1/2)*dq2*dqr1*cos(2*q2)*cos(2*q3)*cos(2*q5)*cos(q6)*sin(q4))/8000 - (37*3^(1/2)*dq3*dqr1*cos(2*q2)*cos(2*q3)*cos(2*q5)*cos(q6)*sin(q4))/8000 + (37*3^(1/2)*dq2*dqr1*cos(2*q5)*sin(2*q2)*sin(2*q3)*cos(q4)*sin(q6))/2000 + (37*3^(1/2)*dq2*dqr1*cos(2*q5)*sin(2*q2)*sin(2*q3)*cos(q6)*sin(q4))/8000 - (37*3^(1/2)*dq3*dqr1*cos(2*q5)*sin(2*q2)*sin(2*q3)*cos(q6)*sin(q4))/8000 + (37*3^(1/2)*dq4*dqr1*cos(2*q2)*sin(2*q3)*sin(2*q5)*cos(q6)*sin(q4))/8000 - (37*3^(1/2)*dq4*dqr1*cos(2*q3)*sin(2*q2)*sin(2*q5)*cos(q6)*sin(q4))/8000 + (37*3^(1/2)*dq5*dqr1*cos(2*q2)*sin(2*q3)*sin(2*q5)*cos(q6)*sin(q4))/8000 - (37*3^(1/2)*dq5*dqr1*cos(2*q3)*sin(2*q2)*sin(2*q5)*cos(q6)*sin(q4))/8000 + (37*3^(1/2)*dq6*dqr1*cos(2*q2)*sin(2*q3)*sin(2*q5)*cos(q6)*sin(q4))/8000 - (37*3^(1/2)*dq6*dqr1*cos(2*q3)*sin(2*q2)*sin(2*q5)*cos(q6)*sin(q4))/8000;
Y1_10_3=dq6*dqr1*sin(q6)*((14539*3^(1/2))/320000 + 111/12800) + (111*dq5*dqr1*cos(2*q5)*sin(q6))/16000 + (111*dq6*dqr1*cos(2*q5)*sin(q6))/64000 - (21*dq6*dqr1*cos(q4)*sin(q6))/4000 + dq6*dqr1*cos(2*q4)*sin(q6)*((1923*3^(1/2))/320000 + 111/12800) - (37*dq4*dqr1*cos(2*q4)*cos(2*q5)*sin(q6))/4000 - (37*dq5*dqr1*cos(2*q4)*cos(2*q5)*sin(q6))/3200 - (37*dq6*dqr1*cos(2*q4)*cos(2*q5)*sin(q6))/12800 + (37*dq4*dqr1*sin(2*q4)*sin(2*q5)*sin(q6))/3200 + (37*dq5*dqr1*sin(2*q4)*sin(2*q5)*sin(q6))/4000 + (37*dq6*dqr1*sin(2*q4)*sin(2*q5)*sin(q6))/16000 - dq5*dqr1*cos(q5)*sin(q6)*((6847*3^(1/2))/160000 - 111/8000) - dq6*dqr1*cos(q5)*sin(q6)*((6847*3^(1/2))/320000 - 111/32000) + dq4*dqr1*cos(2*q4)*cos(q5)*sin(q6)*((641*3^(1/2))/40000 + 37/2000) + dq5*dqr1*cos(2*q4)*cos(q5)*sin(q6)*((641*3^(1/2))/160000 + 37/8000) + dq6*dqr1*cos(2*q4)*cos(q5)*sin(q6)*((641*3^(1/2))/320000 - 37/32000) + (29*3^(1/2)*dq2*dqr1*sin(2*q2)*cos(q3)*cos(q6))/400 - (29*3^(1/2)*dq3*dqr1*sin(2*q2)*cos(q3)*cos(q6))/800 - dq6*dqr1*cos(2*q2)*cos(2*q3)*sin(q6)*((6847*3^(1/2))/320000 - 481/64000) + (333*dq5*dqr1*cos(2*q2)*cos(2*q3)*cos(2*q5)*sin(q6))/16000 + (333*dq6*dqr1*cos(2*q2)*cos(2*q3)*cos(2*q5)*sin(q6))/64000 - dq6*dqr1*sin(2*q2)*sin(2*q3)*sin(q6)*((6847*3^(1/2))/320000 - 481/64000) + (333*dq2*dqr1*cos(2*q2)*sin(2*q3)*sin(2*q5)*sin(q6))/16000 - (333*dq2*dqr1*cos(2*q3)*sin(2*q2)*sin(2*q5)*sin(q6))/16000 - (333*dq3*dqr1*cos(2*q2)*sin(2*q3)*sin(2*q5)*sin(q6))/16000 + (333*dq3*dqr1*cos(2*q3)*sin(2*q2)*sin(2*q5)*sin(q6))/16000 + (333*dq5*dqr1*cos(2*q5)*sin(2*q2)*sin(2*q3)*sin(q6))/16000 + (333*dq6*dqr1*cos(2*q5)*sin(2*q2)*sin(2*q3)*sin(q6))/64000 - (87*dq4*dqr1*sin(2*q2)*cos(q3)*cos(q4)*cos(q6))/800 - (37*dq4*dqr1*sin(2*q2)*sin(2*q3)*sin(2*q4)*sin(2*q5)*sin(q6))/3200 - (37*dq5*dqr1*sin(2*q2)*sin(2*q3)*sin(2*q4)*sin(2*q5)*sin(q6))/4000 - (37*dq6*dqr1*sin(2*q2)*sin(2*q3)*sin(2*q4)*sin(2*q5)*sin(q6))/16000 - (1231*dq4*dqr1*cos(2*q2)*sin(2*q3)*cos(q4)*cos(q5)*cos(q6))/80000 + (1231*dq4*dqr1*cos(2*q3)*sin(2*q2)*cos(q4)*cos(q5)*cos(q6))/80000 - (877*dq6*dqr1*cos(2*q2)*sin(2*q3)*cos(q4)*cos(q5)*cos(q6))/8000 + (877*dq6*dqr1*cos(2*q3)*sin(2*q2)*cos(q4)*cos(q5)*cos(q6))/8000 - (29*3^(1/2)*dq2*dqr1*sin(2*q2)*cos(q3)*cos(q5)*cos(q6))/400 + (29*3^(1/2)*dq3*dqr1*sin(2*q2)*cos(q3)*cos(q5)*cos(q6))/800 - dq4*dqr1*cos(2*q2)*sin(2*q3)*cos(q4)*cos(q6)*((111*3^(1/2))/16000 + 7539/80000) + dq4*dqr1*cos(2*q3)*sin(2*q2)*cos(q4)*cos(q6)*((111*3^(1/2))/16000 + 7539/80000) + dq5*dqr1*cos(2*q2)*cos(2*q3)*cos(q5)*sin(q6)*((9411*3^(1/2))/160000 + 37/8000) - dq2*dqr1*cos(2*q2)*sin(2*q3)*cos(q5)*cos(q6)*((9411*3^(1/2))/160000 - 259/16000) + dq2*dqr1*cos(2*q3)*sin(2*q2)*cos(q5)*cos(q6)*((9411*3^(1/2))/160000 - 259/16000) + dq6*dqr1*cos(2*q2)*cos(2*q3)*cos(q5)*sin(q6)*((9411*3^(1/2))/320000 - 259/32000) + dq5*dqr1*sin(2*q2)*sin(2*q3)*cos(q5)*sin(q6)*((9411*3^(1/2))/160000 + 37/8000) + dq6*dqr1*sin(2*q2)*sin(2*q3)*cos(q5)*sin(q6)*((9411*3^(1/2))/320000 - 259/32000) - (29*dq4*dqr1*sin(2*q2)*cos(q3)*cos(q4)*cos(q5)*cos(q6))/800 - (29*dq5*dqr1*sin(2*q2)*cos(q3)*cos(q4)*cos(q5)*cos(q6))/400 - (29*dq6*dqr1*sin(2*q2)*cos(q3)*cos(q4)*cos(q5)*cos(q6))/200 - dq6*dqr1*cos(2*q2)*cos(2*q3)*cos(2*q4)*sin(q6)*((1923*3^(1/2))/320000 + 111/12800) + (37*dq4*dqr1*cos(2*q2)*cos(2*q3)*cos(2*q4)*cos(2*q5)*sin(q6))/4000 + (37*dq5*dqr1*cos(2*q2)*cos(2*q3)*cos(2*q4)*cos(2*q5)*sin(q6))/3200 + (37*dq6*dqr1*cos(2*q2)*cos(2*q3)*cos(2*q4)*cos(2*q5)*sin(q6))/12800 - dq6*dqr1*cos(2*q4)*sin(2*q2)*sin(2*q3)*sin(q6)*((1923*3^(1/2))/320000 + 111/12800) + (37*dq2*dqr1*cos(2*q2)*cos(2*q4)*sin(2*q3)*sin(2*q5)*sin(q6))/3200 + (37*dq2*dqr1*cos(2*q2)*cos(2*q5)*sin(2*q3)*sin(2*q4)*sin(q6))/4000 - (37*dq2*dqr1*cos(2*q3)*cos(2*q4)*sin(2*q2)*sin(2*q5)*sin(q6))/3200 - (37*dq2*dqr1*cos(2*q3)*cos(2*q5)*sin(2*q2)*sin(2*q4)*sin(q6))/4000 - (37*dq3*dqr1*cos(2*q2)*cos(2*q4)*sin(2*q3)*sin(2*q5)*sin(q6))/3200 - (37*dq3*dqr1*cos(2*q2)*cos(2*q5)*sin(2*q3)*sin(2*q4)*sin(q6))/4000 + (37*dq3*dqr1*cos(2*q3)*cos(2*q4)*sin(2*q2)*sin(2*q5)*sin(q6))/3200 + (37*dq3*dqr1*cos(2*q3)*cos(2*q5)*sin(2*q2)*sin(2*q4)*sin(q6))/4000 - (37*dq4*dqr1*cos(2*q2)*cos(2*q3)*sin(2*q4)*sin(2*q5)*sin(q6))/3200 + (37*dq4*dqr1*cos(2*q4)*cos(2*q5)*sin(2*q2)*sin(2*q3)*sin(q6))/4000 - (37*dq5*dqr1*cos(2*q2)*cos(2*q3)*sin(2*q4)*sin(2*q5)*sin(q6))/4000 + (37*dq5*dqr1*cos(2*q4)*cos(2*q5)*sin(2*q2)*sin(2*q3)*sin(q6))/3200 - (37*dq6*dqr1*cos(2*q2)*cos(2*q3)*sin(2*q4)*sin(2*q5)*sin(q6))/16000 + (37*dq6*dqr1*cos(2*q4)*cos(2*q5)*sin(2*q2)*sin(2*q3)*sin(q6))/12800 + dq5*dqr1*cos(2*q2)*sin(2*q3)*cos(q4)*cos(q5)*cos(q6)*((37*3^(1/2))/8000 - 877/16000) - dq5*dqr1*cos(2*q3)*sin(2*q2)*cos(q4)*cos(q5)*cos(q6)*((37*3^(1/2))/8000 - 877/16000) - dq4*dqr1*cos(2*q2)*cos(2*q3)*cos(2*q4)*cos(q5)*sin(q6)*((641*3^(1/2))/40000 + 37/2000) - dq5*dqr1*cos(2*q2)*cos(2*q3)*cos(2*q4)*cos(q5)*sin(q6)*((641*3^(1/2))/160000 + 37/8000) + dq2*dqr1*cos(2*q2)*cos(2*q4)*sin(2*q3)*cos(q5)*cos(q6)*((641*3^(1/2))/160000 - 37/16000) - dq2*dqr1*cos(2*q3)*cos(2*q4)*sin(2*q2)*cos(q5)*cos(q6)*((641*3^(1/2))/160000 - 37/16000) - dq6*dqr1*cos(2*q2)*cos(2*q3)*cos(2*q4)*cos(q5)*sin(q6)*((641*3^(1/2))/320000 - 37/32000) - dq2*dqr1*cos(2*q2)*sin(2*q3)*sin(2*q4)*cos(q5)*sin(q6)*((641*3^(1/2))/40000 + 37/2000) + dq2*dqr1*cos(2*q3)*sin(2*q2)*sin(2*q4)*cos(q5)*sin(q6)*((641*3^(1/2))/40000 + 37/2000) + dq3*dqr1*cos(2*q2)*sin(2*q3)*sin(2*q4)*cos(q5)*sin(q6)*((641*3^(1/2))/40000 + 37/2000) - dq3*dqr1*cos(2*q3)*sin(2*q2)*sin(2*q4)*cos(q5)*sin(q6)*((641*3^(1/2))/40000 + 37/2000) - dq4*dqr1*cos(2*q4)*sin(2*q2)*sin(2*q3)*cos(q5)*sin(q6)*((641*3^(1/2))/40000 + 37/2000) - dq5*dqr1*cos(2*q4)*sin(2*q2)*sin(2*q3)*cos(q5)*sin(q6)*((641*3^(1/2))/160000 + 37/8000) - dq6*dqr1*cos(2*q4)*sin(2*q2)*sin(2*q3)*cos(q5)*sin(q6)*((641*3^(1/2))/320000 - 37/32000) + (37*3^(1/2)*dq2*dqr1*cos(2*q2)*cos(2*q3)*sin(2*q5)*cos(q4)*cos(q6))/4000 - (37*3^(1/2)*dq3*dqr1*cos(2*q2)*cos(2*q3)*cos(2*q5)*cos(q4)*sin(q6))/2000 - (37*3^(1/2)*dq3*dqr1*cos(2*q2)*cos(2*q3)*sin(2*q5)*cos(q4)*cos(q6))/4000 - (37*3^(1/2)*dq4*dqr1*cos(2*q2)*cos(2*q5)*sin(2*q3)*cos(q4)*cos(q6))/16000 + (37*3^(1/2)*dq4*dqr1*cos(2*q3)*cos(2*q5)*sin(2*q2)*cos(q4)*cos(q6))/16000 - (37*3^(1/2)*dq5*dqr1*cos(2*q2)*cos(2*q5)*sin(2*q3)*cos(q4)*cos(q6))/4000 + (37*3^(1/2)*dq5*dqr1*cos(2*q3)*cos(2*q5)*sin(2*q2)*cos(q4)*cos(q6))/4000 - (37*3^(1/2)*dq6*dqr1*cos(2*q2)*cos(2*q5)*sin(2*q3)*cos(q4)*cos(q6))/4000 + (37*3^(1/2)*dq6*dqr1*cos(2*q3)*cos(2*q5)*sin(2*q2)*cos(q4)*cos(q6))/4000 + (37*3^(1/2)*dq2*dqr1*sin(2*q2)*sin(2*q3)*sin(2*q5)*cos(q4)*cos(q6))/4000 - (37*3^(1/2)*dq3*dqr1*cos(2*q5)*sin(2*q2)*sin(2*q3)*cos(q4)*sin(q6))/2000 - (37*3^(1/2)*dq3*dqr1*sin(2*q2)*sin(2*q3)*sin(2*q5)*cos(q4)*cos(q6))/4000 + (37*3^(1/2)*dq4*dqr1*cos(2*q2)*sin(2*q3)*sin(2*q5)*cos(q4)*sin(q6))/8000 - (37*3^(1/2)*dq4*dqr1*cos(2*q3)*sin(2*q2)*sin(2*q5)*cos(q4)*sin(q6))/8000 + (37*3^(1/2)*dq5*dqr1*cos(2*q2)*sin(2*q3)*sin(2*q5)*cos(q4)*sin(q6))/2000 - (37*3^(1/2)*dq5*dqr1*cos(2*q3)*sin(2*q2)*sin(2*q5)*cos(q4)*sin(q6))/2000 + (37*3^(1/2)*dq6*dqr1*cos(2*q2)*sin(2*q3)*sin(2*q5)*cos(q4)*sin(q6))/8000 - (37*3^(1/2)*dq6*dqr1*cos(2*q3)*sin(2*q2)*sin(2*q5)*cos(q4)*sin(q6))/8000;
Y1_10_4=(111*dq5*dqr1*sin(2*q5)*cos(q6))/32000 + (111*dq6*dqr1*sin(2*q5)*cos(q6))/32000 + dq4*dqr1*sin(2*q4)*cos(q6)*((1923*3^(1/2))/160000 + 111/6400) - (37*dq4*dqr1*cos(2*q4)*sin(2*q5)*cos(q6))/8000 - (37*dq4*dqr1*cos(2*q5)*sin(2*q4)*cos(q6))/6400 - (37*dq5*dqr1*cos(2*q4)*sin(2*q5)*cos(q6))/6400 - (37*dq5*dqr1*cos(2*q5)*sin(2*q4)*cos(q6))/8000 - (37*dq6*dqr1*cos(2*q4)*sin(2*q5)*cos(q6))/6400 - (37*dq6*dqr1*cos(2*q5)*sin(2*q4)*cos(q6))/8000 + dq6*dqr1*sin(2*q4)*cos(q5)*cos(q6)*((641*3^(1/2))/80000 + 37/4000) + dq4*dqr1*sin(2*q4)*cos(q5)*cos(q6)*((641*3^(1/2))/160000 - 37/16000) + dq5*dqr1*sin(2*q4)*cos(q5)*cos(q6)*((641*3^(1/2))/160000 - 37/16000) + (7*3^(1/2)*dq6*dqr2*sin(q2)*sin(q3)*sin(q6))/4000 + dq2*dqr1*cos(2*q2)*sin(2*q3)*cos(q6)*((6847*3^(1/2))/160000 - 481/32000) - dq2*dqr1*cos(2*q3)*sin(2*q2)*cos(q6)*((6847*3^(1/2))/160000 - 481/32000) - dq3*dqr1*cos(2*q2)*sin(2*q3)*cos(q6)*((6847*3^(1/2))/160000 - 481/32000) + dq3*dqr1*cos(2*q3)*sin(2*q2)*cos(q6)*((6847*3^(1/2))/160000 - 481/32000) - (333*dq2*dqr1*cos(2*q2)*cos(2*q5)*sin(2*q3)*cos(q6))/32000 + (333*dq2*dqr1*cos(2*q3)*cos(2*q5)*sin(2*q2)*cos(q6))/32000 + (333*dq3*dqr1*cos(2*q2)*cos(2*q5)*sin(2*q3)*cos(q6))/32000 - (333*dq3*dqr1*cos(2*q3)*cos(2*q5)*sin(2*q2)*cos(q6))/32000 + (333*dq5*dqr1*cos(2*q2)*cos(2*q3)*sin(2*q5)*cos(q6))/32000 + (333*dq6*dqr1*cos(2*q2)*cos(2*q3)*sin(2*q5)*cos(q6))/32000 - (21*dq2*dqr2*cos(q6)*sin(q2)*sin(q3)*sin(q4))/4000 + (21*dq3*dqr2*cos(q6)*sin(q2)*sin(q3)*sin(q4))/4000 + (333*dq5*dqr1*sin(2*q2)*sin(2*q3)*sin(2*q5)*cos(q6))/32000 + (333*dq6*dqr1*sin(2*q2)*sin(2*q3)*sin(2*q5)*cos(q6))/32000 + (37*3^(1/2)*dq5*dqr2*cos(q6)*sin(q2)*sin(q3)*sin(q4))/4000 - (7*3^(1/2)*dq5*dqr2*cos(q5)*sin(q2)*sin(q3)*sin(q6))/2000 - (7*3^(1/2)*dq5*dqr2*cos(q6)*sin(q2)*sin(q3)*sin(q5))/4000 + (37*3^(1/2)*dq6*dqr2*cos(q6)*sin(q2)*sin(q3)*sin(q4))/4000 - (7*3^(1/2)*dq6*dqr2*cos(q5)*sin(q2)*sin(q3)*sin(q6))/4000 - (7*3^(1/2)*dq6*dqr2*cos(q6)*sin(q2)*sin(q3)*sin(q5))/2000 - (37*dq2*dqr2*cos(2*q4)*cos(2*q5)*sin(q2)*sin(q3)*sin(q6))/2000 + (37*dq3*dqr2*cos(2*q4)*cos(2*q5)*sin(q2)*sin(q3)*sin(q6))/2000 + (37*dq2*dqr2*sin(2*q4)*sin(2*q5)*sin(q2)*sin(q3)*sin(q6))/1600 - (37*dq3*dqr2*sin(2*q4)*sin(2*q5)*sin(q2)*sin(q3)*sin(q6))/1600 + dq3*dqr1*cos(2*q2)*sin(2*q3)*cos(q5)*cos(q6)*((9411*3^(1/2))/160000 - 259/16000) - dq3*dqr1*cos(2*q3)*sin(2*q2)*cos(q5)*cos(q6)*((9411*3^(1/2))/160000 - 259/16000) - (7*dq2*dqr2*cos(q4)*cos(q5)*sin(q2)*sin(q3)*sin(q6))/1000 - (7*dq2*dqr2*cos(q4)*cos(q6)*sin(q2)*sin(q3)*sin(q5))/2000 - (7*dq2*dqr2*cos(q5)*cos(q6)*sin(q2)*sin(q3)*sin(q4))/4000 + (7*dq3*dqr2*cos(q4)*cos(q5)*sin(q2)*sin(q3)*sin(q6))/1000 + (7*dq3*dqr2*cos(q4)*cos(q6)*sin(q2)*sin(q3)*sin(q5))/2000 + (7*dq3*dqr2*cos(q5)*cos(q6)*sin(q2)*sin(q3)*sin(q4))/4000 + (7*dq2*dqr2*sin(q2)*sin(q3)*sin(q4)*sin(q5)*sin(q6))/2000 - (7*dq3*dqr2*sin(q2)*sin(q3)*sin(q4)*sin(q5)*sin(q6))/2000 + dq2*dqr1*cos(2*q2)*cos(2*q4)*sin(2*q3)*cos(q6)*((1923*3^(1/2))/160000 + 111/6400) - dq2*dqr1*cos(2*q3)*cos(2*q4)*sin(2*q2)*cos(q6)*((1923*3^(1/2))/160000 + 111/6400) - dq3*dqr1*cos(2*q2)*cos(2*q4)*sin(2*q3)*cos(q6)*((1923*3^(1/2))/160000 + 111/6400) + dq3*dqr1*cos(2*q3)*cos(2*q4)*sin(2*q2)*cos(q6)*((1923*3^(1/2))/160000 + 111/6400) - dq4*dqr1*cos(2*q2)*cos(2*q3)*sin(2*q4)*cos(q6)*((1923*3^(1/2))/160000 + 111/6400) - dq6*dqr2*cos(q4)*sin(q2)*sin(q3)*sin(q6)*((37*3^(1/2))/3200 + 1923/80000) - (37*dq2*dqr1*cos(2*q2)*cos(2*q4)*cos(2*q5)*sin(2*q3)*cos(q6))/6400 + (37*dq2*dqr1*cos(2*q3)*cos(2*q4)*cos(2*q5)*sin(2*q2)*cos(q6))/6400 + (37*dq3*dqr1*cos(2*q2)*cos(2*q4)*cos(2*q5)*sin(2*q3)*cos(q6))/6400 - (37*dq3*dqr1*cos(2*q3)*cos(2*q4)*cos(2*q5)*sin(2*q2)*cos(q6))/6400 + (37*dq4*dqr1*cos(2*q2)*cos(2*q3)*cos(2*q4)*sin(2*q5)*cos(q6))/8000 + (37*dq4*dqr1*cos(2*q2)*cos(2*q3)*cos(2*q5)*sin(2*q4)*cos(q6))/6400 + (37*dq5*dqr1*cos(2*q2)*cos(2*q3)*cos(2*q4)*sin(2*q5)*cos(q6))/6400 + (37*dq5*dqr1*cos(2*q2)*cos(2*q3)*cos(2*q5)*sin(2*q4)*cos(q6))/8000 + (37*dq6*dqr1*cos(2*q2)*cos(2*q3)*cos(2*q4)*sin(2*q5)*cos(q6))/6400 + (37*dq6*dqr1*cos(2*q2)*cos(2*q3)*cos(2*q5)*sin(2*q4)*cos(q6))/8000 - dq4*dqr1*sin(2*q2)*sin(2*q3)*sin(2*q4)*cos(q6)*((1923*3^(1/2))/160000 + 111/6400) + (37*dq2*dqr1*cos(2*q2)*sin(2*q3)*sin(2*q4)*sin(2*q5)*cos(q6))/8000 - (37*dq2*dqr1*cos(2*q3)*sin(2*q2)*sin(2*q4)*sin(2*q5)*cos(q6))/8000 - (37*dq3*dqr1*cos(2*q2)*sin(2*q3)*sin(2*q4)*sin(2*q5)*cos(q6))/8000 + (37*dq3*dqr1*cos(2*q3)*sin(2*q2)*sin(2*q4)*sin(2*q5)*cos(q6))/8000 + (37*dq4*dqr1*cos(2*q4)*sin(2*q2)*sin(2*q3)*sin(2*q5)*cos(q6))/8000 + (37*dq4*dqr1*cos(2*q5)*sin(2*q2)*sin(2*q3)*sin(2*q4)*cos(q6))/6400 + (37*dq5*dqr1*cos(2*q4)*sin(2*q2)*sin(2*q3)*sin(2*q5)*cos(q6))/6400 + (37*dq5*dqr1*cos(2*q5)*sin(2*q2)*sin(2*q3)*sin(2*q4)*cos(q6))/8000 + (37*dq6*dqr1*cos(2*q4)*sin(2*q2)*sin(2*q3)*sin(2*q5)*cos(q6))/6400 + (37*dq6*dqr1*cos(2*q5)*sin(2*q2)*sin(2*q3)*sin(2*q4)*cos(q6))/8000 - dq2*dqr2*sin(2*q4)*sin(q2)*sin(q3)*sin(q5)*sin(q6)*((641*3^(1/2))/40000 + 37/2000) + dq3*dqr2*sin(2*q4)*sin(q2)*sin(q3)*sin(q5)*sin(q6)*((641*3^(1/2))/40000 + 37/2000) - (37*3^(1/2)*dq5*dqr2*cos(2*q5)*cos(q4)*sin(q2)*sin(q3)*sin(q6))/4000 - (37*3^(1/2)*dq5*dqr2*cos(2*q5)*cos(q6)*sin(q2)*sin(q3)*sin(q4))/4000 - (37*3^(1/2)*dq5*dqr2*sin(2*q5)*cos(q4)*cos(q6)*sin(q2)*sin(q3))/8000 - (37*3^(1/2)*dq6*dqr2*cos(2*q5)*cos(q4)*sin(q2)*sin(q3)*sin(q6))/16000 - (37*3^(1/2)*dq6*dqr2*cos(2*q5)*cos(q6)*sin(q2)*sin(q3)*sin(q4))/4000 + (37*3^(1/2)*dq5*dqr2*sin(2*q5)*sin(q2)*sin(q3)*sin(q4)*sin(q6))/2000 + (37*3^(1/2)*dq6*dqr2*sin(2*q5)*sin(q2)*sin(q3)*sin(q4)*sin(q6))/8000 - dq6*dqr1*cos(2*q2)*cos(2*q3)*sin(2*q4)*cos(q5)*cos(q6)*((641*3^(1/2))/80000 + 37/4000) - dq3*dqr1*cos(2*q2)*cos(2*q4)*sin(2*q3)*cos(q5)*cos(q6)*((641*3^(1/2))/160000 - 37/16000) + dq3*dqr1*cos(2*q3)*cos(2*q4)*sin(2*q2)*cos(q5)*cos(q6)*((641*3^(1/2))/160000 - 37/16000) - dq4*dqr1*cos(2*q2)*cos(2*q3)*sin(2*q4)*cos(q5)*cos(q6)*((641*3^(1/2))/160000 - 37/16000) - dq5*dqr1*cos(2*q2)*cos(2*q3)*sin(2*q4)*cos(q5)*cos(q6)*((641*3^(1/2))/160000 - 37/16000) + dq5*dqr2*cos(q4)*cos(q5)*sin(q2)*sin(q3)*sin(q6)*((37*3^(1/2))/2000 + 1923/40000) + dq6*dqr2*cos(q4)*cos(q6)*sin(q2)*sin(q3)*sin(q5)*((37*3^(1/2))/2000 + 1923/40000) - dq5*dqr2*cos(q4)*cos(q6)*sin(q2)*sin(q3)*sin(q5)*((37*3^(1/2))/8000 - 1923/80000) + dq6*dqr2*cos(q4)*cos(q5)*sin(q2)*sin(q3)*sin(q6)*((111*3^(1/2))/8000 + 1923/80000) - dq6*dqr1*sin(2*q2)*sin(2*q3)*sin(2*q4)*cos(q5)*cos(q6)*((641*3^(1/2))/80000 + 37/4000) - dq4*dqr1*sin(2*q2)*sin(2*q3)*sin(2*q4)*cos(q5)*cos(q6)*((641*3^(1/2))/160000 - 37/16000) - dq5*dqr1*sin(2*q2)*sin(2*q3)*sin(2*q4)*cos(q5)*cos(q6)*((641*3^(1/2))/160000 - 37/16000) + dq2*dqr2*cos(2*q4)*cos(q5)*sin(q2)*sin(q3)*sin(q6)*((641*3^(1/2))/20000 + 37/1000) - dq3*dqr2*cos(2*q4)*cos(q5)*sin(q2)*sin(q3)*sin(q6)*((641*3^(1/2))/20000 + 37/1000) + dq2*dqr2*cos(2*q4)*cos(q6)*sin(q2)*sin(q3)*sin(q5)*((641*3^(1/2))/40000 - 37/4000) - dq3*dqr2*cos(2*q4)*cos(q6)*sin(q2)*sin(q3)*sin(q5)*((641*3^(1/2))/40000 - 37/4000) - (37*3^(1/2)*dq6*dqr2*sin(q2)*sin(q3)*sin(q4)*sin(q5)*sin(q6))/4000;
Y1_10_5=(87*dq2*dqr2*cos(q4)*cos(q6)*sin(q2))/400 - (37*dq5*dqr2*cos(q3)*cos(q6)*sin(q2))/4000 - (37*dq6*dqr2*cos(q3)*cos(q6)*sin(q2))/4000 - (111*dq4*dqr2*sin(2*q5)*cos(q3)*sin(q2)*sin(q6))/8000 + (7*3^(1/2)*dq2*dqr2*cos(q3)*cos(q6)*sin(q2))/4000 - (7*3^(1/2)*dq3*dqr2*cos(q3)*cos(q6)*sin(q2))/4000 + (29*dq2*dqr2*cos(q4)*cos(q5)*cos(q6)*sin(q2))/400 - (21*dq4*dqr2*cos(q3)*cos(q4)*cos(q6)*sin(q2))/4000 - (29*dq2*dqr2*cos(q4)*sin(q2)*sin(q5)*sin(q6))/200 - (29*dq2*dqr2*cos(q5)*sin(q2)*sin(q4)*sin(q6))/100 - (29*dq2*dqr2*cos(q6)*sin(q2)*sin(q4)*sin(q5))/200 + (21*dq6*dqr2*cos(q3)*sin(q2)*sin(q4)*sin(q6))/4000 + dq4*dqr2*cos(q3)*cos(q6)*sin(q2)*((1923*3^(1/2))/80000 + 259/16000) + (111*dq4*dqr2*cos(2*q5)*cos(q3)*cos(q6)*sin(q2))/16000 + dq4*dqr2*cos(2*q4)*cos(q3)*cos(q6)*sin(q2)*((1923*3^(1/2))/80000 + 111/3200) + (7*3^(1/2)*dq2*dqr2*cos(q3)*sin(q2)*sin(q5)*sin(q6))/2000 - (7*3^(1/2)*dq3*dqr2*cos(q3)*sin(q2)*sin(q5)*sin(q6))/2000 - (37*dq4*dqr2*cos(2*q4)*cos(2*q5)*cos(q3)*cos(q6)*sin(q2))/3200 - (37*dq5*dqr2*cos(2*q4)*cos(2*q5)*cos(q3)*cos(q6)*sin(q2))/4000 - (37*dq6*dqr2*cos(2*q4)*cos(2*q5)*cos(q3)*cos(q6)*sin(q2))/4000 + dq2*dqr2*sin(2*q4)*cos(q6)*sin(q2)*sin(q3)*((1923*3^(1/2))/80000 + 111/3200) - dq3*dqr2*sin(2*q4)*cos(q6)*sin(q2)*sin(q3)*((1923*3^(1/2))/80000 + 111/3200) - dq6*dqr2*sin(2*q4)*cos(q3)*sin(q2)*sin(q6)*((1923*3^(1/2))/160000 + 111/6400) - (37*dq2*dqr2*cos(2*q4)*sin(2*q5)*cos(q6)*sin(q2)*sin(q3))/4000 - (37*dq2*dqr2*cos(2*q5)*sin(2*q4)*cos(q6)*sin(q2)*sin(q3))/3200 + (37*dq3*dqr2*cos(2*q4)*sin(2*q5)*cos(q6)*sin(q2)*sin(q3))/4000 + (37*dq3*dqr2*cos(2*q5)*sin(2*q4)*cos(q6)*sin(q2)*sin(q3))/3200 + (37*dq4*dqr2*cos(2*q4)*sin(2*q5)*cos(q3)*sin(q2)*sin(q6))/1600 + (37*dq4*dqr2*cos(2*q5)*sin(2*q4)*cos(q3)*sin(q2)*sin(q6))/2000 + (37*dq4*dqr2*sin(2*q4)*sin(2*q5)*cos(q3)*cos(q6)*sin(q2))/4000 + (37*dq5*dqr2*cos(2*q4)*sin(2*q5)*cos(q3)*sin(q2)*sin(q6))/2000 + (37*dq5*dqr2*cos(2*q5)*sin(2*q4)*cos(q3)*sin(q2)*sin(q6))/1600 + (37*dq5*dqr2*sin(2*q4)*sin(2*q5)*cos(q3)*cos(q6)*sin(q2))/3200 + (37*dq6*dqr2*cos(2*q4)*sin(2*q5)*cos(q3)*sin(q2)*sin(q6))/8000 + (37*dq6*dqr2*cos(2*q5)*sin(2*q4)*cos(q3)*sin(q2)*sin(q6))/6400 + (37*dq6*dqr2*sin(2*q4)*sin(2*q5)*cos(q3)*cos(q6)*sin(q2))/3200 - (1231*dq2*dqr2*cos(q3)*cos(q4)*cos(q5)*cos(q6)*sin(q2))/40000 + (1231*dq3*dqr2*cos(q3)*cos(q4)*cos(q5)*cos(q6)*sin(q2))/40000 - (7*dq4*dqr2*cos(q3)*cos(q4)*cos(q5)*cos(q6)*sin(q2))/4000 - (7*dq5*dqr2*cos(q3)*cos(q4)*cos(q5)*cos(q6)*sin(q2))/2000 - (7*dq6*dqr2*cos(q3)*cos(q4)*cos(q5)*cos(q6)*sin(q2))/1000 - (877*dq2*dqr2*cos(q2)*cos(q5)*sin(q3)*sin(q4)*sin(q6))/4000 + (877*dq2*dqr2*cos(q3)*cos(q5)*sin(q2)*sin(q4)*sin(q6))/4000 + (877*dq3*dqr2*cos(q2)*cos(q5)*sin(q3)*sin(q4)*sin(q6))/4000 - (877*dq3*dqr2*cos(q3)*cos(q5)*sin(q2)*sin(q4)*sin(q6))/4000 - (7*dq4*dqr2*cos(q2)*cos(q5)*sin(q3)*sin(q4)*sin(q6))/1000 - (7*dq4*dqr2*cos(q2)*cos(q6)*sin(q3)*sin(q4)*sin(q5))/2000 + (7*dq4*dqr2*cos(q3)*cos(q4)*sin(q2)*sin(q5)*sin(q6))/2000 + (7*dq4*dqr2*cos(q3)*cos(q5)*sin(q2)*sin(q4)*sin(q6))/1000 + (7*dq4*dqr2*cos(q3)*cos(q6)*sin(q2)*sin(q4)*sin(q5))/2000 - (7*dq5*dqr2*cos(q2)*cos(q5)*sin(q3)*sin(q4)*sin(q6))/2000 - (7*dq5*dqr2*cos(q2)*cos(q6)*sin(q3)*sin(q4)*sin(q5))/4000 + (7*dq5*dqr2*cos(q3)*cos(q4)*sin(q2)*sin(q5)*sin(q6))/1000 + (7*dq5*dqr2*cos(q3)*cos(q5)*sin(q2)*sin(q4)*sin(q6))/2000 + (7*dq5*dqr2*cos(q3)*cos(q6)*sin(q2)*sin(q4)*sin(q5))/4000 - (7*dq6*dqr2*cos(q2)*cos(q5)*sin(q3)*sin(q4)*sin(q6))/4000 - (7*dq6*dqr2*cos(q2)*cos(q6)*sin(q3)*sin(q4)*sin(q5))/2000 + (7*dq6*dqr2*cos(q3)*cos(q4)*sin(q2)*sin(q5)*sin(q6))/2000 + (7*dq6*dqr2*cos(q3)*cos(q5)*sin(q2)*sin(q4)*sin(q6))/4000 + (7*dq6*dqr2*cos(q3)*cos(q6)*sin(q2)*sin(q4)*sin(q5))/2000 + dq6*dqr2*cos(q3)*cos(q5)*cos(q6)*sin(q2)*((641*3^(1/2))/40000 + 37/2000) - dq2*dqr2*cos(q3)*cos(q4)*cos(q6)*sin(q2)*((111*3^(1/2))/8000 + 7539/40000) + dq3*dqr2*cos(q3)*cos(q4)*cos(q6)*sin(q2)*((111*3^(1/2))/8000 + 7539/40000) + dq4*dqr2*cos(q3)*cos(q5)*cos(q6)*sin(q2)*((641*3^(1/2))/80000 - 37/8000) + dq5*dqr2*cos(q3)*cos(q5)*cos(q6)*sin(q2)*((641*3^(1/2))/80000 - 37/8000) - dq4*dqr2*cos(q3)*sin(q2)*sin(q5)*sin(q6)*((641*3^(1/2))/40000 + 37/2000) - dq5*dqr2*cos(q3)*sin(q2)*sin(q5)*sin(q6)*((641*3^(1/2))/40000 + 37/2000) - dq6*dqr2*cos(q3)*sin(q2)*sin(q5)*sin(q6)*((641*3^(1/2))/80000 + 37/1600) - (7*3^(1/2)*dq2*dqr2*cos(q3)*cos(q5)*cos(q6)*sin(q2))/4000 + (7*3^(1/2)*dq3*dqr2*cos(q3)*cos(q5)*cos(q6)*sin(q2))/4000 + (29*dq1*dqr2*sin(2*q2)*sin(q3)*sin(q4)*sin(q5)*sin(q6))/200 - (37*3^(1/2)*dq2*dqr2*cos(2*q5)*cos(q3)*cos(q4)*cos(q6)*sin(q2))/8000 + (37*3^(1/2)*dq3*dqr2*cos(2*q5)*cos(q3)*cos(q4)*cos(q6)*sin(q2))/8000 + (37*3^(1/2)*dq2*dqr2*cos(2*q5)*cos(q3)*sin(q2)*sin(q4)*sin(q6))/2000 + (37*3^(1/2)*dq2*dqr2*sin(2*q5)*cos(q3)*cos(q4)*sin(q2)*sin(q6))/4000 + (37*3^(1/2)*dq2*dqr2*sin(2*q5)*cos(q3)*cos(q6)*sin(q2)*sin(q4))/4000 - (37*3^(1/2)*dq3*dqr2*cos(2*q5)*cos(q3)*sin(q2)*sin(q4)*sin(q6))/2000 - (37*3^(1/2)*dq3*dqr2*sin(2*q5)*cos(q3)*cos(q4)*sin(q2)*sin(q6))/4000 - (37*3^(1/2)*dq3*dqr2*sin(2*q5)*cos(q3)*cos(q6)*sin(q2)*sin(q4))/4000 - (37*3^(1/2)*dq6*dqr2*sin(2*q5)*cos(q4)*cos(q6)*sin(q2)*sin(q3))/8000 + dq2*dqr2*cos(q2)*cos(q6)*sin(q3)*sin(q4)*sin(q5)*((37*3^(1/2))/4000 - 877/8000) - dq2*dqr2*cos(q3)*cos(q6)*sin(q2)*sin(q4)*sin(q5)*((37*3^(1/2))/4000 - 877/8000) - dq3*dqr2*cos(q2)*cos(q6)*sin(q3)*sin(q4)*sin(q5)*((37*3^(1/2))/4000 - 877/8000) + dq3*dqr2*cos(q3)*cos(q6)*sin(q2)*sin(q4)*sin(q5)*((37*3^(1/2))/4000 - 877/8000) - dq2*dqr2*cos(q3)*cos(q4)*sin(q2)*sin(q5)*sin(q6)*((37*3^(1/2))/2000 - 1231/20000) + dq3*dqr2*cos(q3)*cos(q4)*sin(q2)*sin(q5)*sin(q6)*((37*3^(1/2))/2000 - 1231/20000) + dq6*dqr2*cos(2*q4)*cos(q3)*cos(q5)*cos(q6)*sin(q2)*((641*3^(1/2))/40000 + 37/2000) + dq4*dqr2*cos(2*q4)*cos(q3)*cos(q5)*cos(q6)*sin(q2)*((641*3^(1/2))/80000 - 37/8000) + dq5*dqr2*cos(2*q4)*cos(q3)*cos(q5)*cos(q6)*sin(q2)*((641*3^(1/2))/80000 - 37/8000) - dq4*dqr2*sin(2*q4)*cos(q3)*cos(q5)*sin(q2)*sin(q6)*((641*3^(1/2))/20000 + 37/1000) - dq4*dqr2*cos(2*q4)*cos(q3)*sin(q2)*sin(q5)*sin(q6)*((641*3^(1/2))/40000 + 37/2000) - dq5*dqr2*cos(2*q4)*cos(q3)*sin(q2)*sin(q5)*sin(q6)*((641*3^(1/2))/40000 + 37/2000) - dq4*dqr2*sin(2*q4)*cos(q3)*cos(q6)*sin(q2)*sin(q5)*((641*3^(1/2))/40000 - 37/4000) - dq5*dqr2*sin(2*q4)*cos(q3)*cos(q5)*sin(q2)*sin(q6)*((641*3^(1/2))/80000 + 37/4000) - dq6*dqr2*sin(2*q4)*cos(q3)*cos(q6)*sin(q2)*sin(q5)*((641*3^(1/2))/80000 + 37/4000) + dq2*dqr2*sin(2*q4)*cos(q5)*cos(q6)*sin(q2)*sin(q3)*((641*3^(1/2))/80000 - 37/8000) - dq3*dqr2*sin(2*q4)*cos(q5)*cos(q6)*sin(q2)*sin(q3)*((641*3^(1/2))/80000 - 37/8000) - dq6*dqr2*cos(2*q4)*cos(q3)*sin(q2)*sin(q5)*sin(q6)*((641*3^(1/2))/80000 - 37/8000) - dq5*dqr2*sin(2*q4)*cos(q3)*cos(q6)*sin(q2)*sin(q5)*((641*3^(1/2))/160000 - 37/16000) - dq6*dqr2*sin(2*q4)*cos(q3)*cos(q5)*sin(q2)*sin(q6)*((641*3^(1/2))/160000 - 37/16000);
Y1_10_6=(37*dq5*dqr2*cos(q2)*cos(q6)*sin(q3))/4000 + (37*dq6*dqr2*cos(q2)*cos(q6)*sin(q3))/4000 - (87*dq1*dqr2*sin(2*q2)*cos(q6)*sin(q3)*sin(q4))/400 + (111*dq4*dqr2*sin(2*q5)*cos(q2)*sin(q3)*sin(q6))/8000 - (7*3^(1/2)*dq2*dqr2*cos(q2)*cos(q6)*sin(q3))/4000 + (7*3^(1/2)*dq3*dqr2*cos(q2)*cos(q6)*sin(q3))/4000 - (29*3^(1/2)*dq1*dqr2*cos(2*q2)*cos(q6)*sin(q3))/400 - (21*dq2*dqr2*cos(q2)*cos(q3)*cos(q6)*sin(q4))/4000 + (21*dq3*dqr2*cos(q2)*cos(q3)*cos(q6)*sin(q4))/4000 + (21*dq4*dqr2*cos(q2)*cos(q4)*cos(q6)*sin(q3))/4000 - (21*dq6*dqr2*cos(q2)*sin(q3)*sin(q4)*sin(q6))/4000 - dq4*dqr2*cos(q2)*cos(q6)*sin(q3)*((1923*3^(1/2))/80000 + 259/16000) - (87*dq1*dqr2*cos(2*q2)*cos(q3)*cos(q6)*sin(q4))/400 - (111*dq4*dqr2*cos(2*q5)*cos(q2)*cos(q6)*sin(q3))/16000 - dq4*dqr2*cos(2*q4)*cos(q2)*cos(q6)*sin(q3)*((1923*3^(1/2))/80000 + 111/3200) - (7*3^(1/2)*dq2*dqr2*cos(q2)*sin(q3)*sin(q5)*sin(q6))/2000 + (7*3^(1/2)*dq3*dqr2*cos(q2)*sin(q3)*sin(q5)*sin(q6))/2000 + (1231*dq1*dqr2*cos(2*q2)*cos(2*q3)*cos(q5)*cos(q6)*sin(q4))/40000 + (37*dq4*dqr2*cos(2*q4)*cos(2*q5)*cos(q2)*cos(q6)*sin(q3))/3200 + (37*dq5*dqr2*cos(2*q4)*cos(2*q5)*cos(q2)*cos(q6)*sin(q3))/4000 + (37*dq6*dqr2*cos(2*q4)*cos(2*q5)*cos(q2)*cos(q6)*sin(q3))/4000 + dq6*dqr2*sin(2*q4)*cos(q2)*sin(q3)*sin(q6)*((1923*3^(1/2))/160000 + 111/6400) + (1231*dq1*dqr2*sin(2*q2)*sin(2*q3)*cos(q5)*cos(q6)*sin(q4))/40000 - (37*dq4*dqr2*cos(2*q4)*sin(2*q5)*cos(q2)*sin(q3)*sin(q6))/1600 - (37*dq4*dqr2*cos(2*q5)*sin(2*q4)*cos(q2)*sin(q3)*sin(q6))/2000 - (37*dq4*dqr2*sin(2*q4)*sin(2*q5)*cos(q2)*cos(q6)*sin(q3))/4000 - (37*dq5*dqr2*cos(2*q4)*sin(2*q5)*cos(q2)*sin(q3)*sin(q6))/2000 - (37*dq5*dqr2*cos(2*q5)*sin(2*q4)*cos(q2)*sin(q3)*sin(q6))/1600 - (37*dq5*dqr2*sin(2*q4)*sin(2*q5)*cos(q2)*cos(q6)*sin(q3))/3200 - (37*dq6*dqr2*cos(2*q4)*sin(2*q5)*cos(q2)*sin(q3)*sin(q6))/8000 - (37*dq6*dqr2*cos(2*q5)*sin(2*q4)*cos(q2)*sin(q3)*sin(q6))/6400 - (37*dq6*dqr2*sin(2*q4)*sin(2*q5)*cos(q2)*cos(q6)*sin(q3))/3200 + (29*3^(1/2)*dq1*dqr2*cos(2*q2)*cos(q5)*cos(q6)*sin(q3))/400 - (7*dq2*dqr2*cos(q2)*cos(q3)*cos(q5)*cos(q6)*sin(q4))/4000 + (1231*dq2*dqr2*cos(q2)*cos(q4)*cos(q5)*cos(q6)*sin(q3))/40000 + (7*dq3*dqr2*cos(q2)*cos(q3)*cos(q5)*cos(q6)*sin(q4))/4000 - (1231*dq3*dqr2*cos(q2)*cos(q4)*cos(q5)*cos(q6)*sin(q3))/40000 + (7*dq4*dqr2*cos(q2)*cos(q4)*cos(q5)*cos(q6)*sin(q3))/4000 + (7*dq5*dqr2*cos(q2)*cos(q4)*cos(q5)*cos(q6)*sin(q3))/2000 + (7*dq6*dqr2*cos(q2)*cos(q4)*cos(q5)*cos(q6)*sin(q3))/1000 + dq1*dqr2*cos(2*q2)*cos(2*q3)*cos(q6)*sin(q4)*((111*3^(1/2))/8000 + 7539/40000) - (29*3^(1/2)*dq1*dqr2*cos(2*q2)*sin(q3)*sin(q5)*sin(q6))/200 + (7*dq2*dqr2*cos(q2)*cos(q3)*sin(q4)*sin(q5)*sin(q6))/2000 - (7*dq3*dqr2*cos(q2)*cos(q3)*sin(q4)*sin(q5)*sin(q6))/2000 - (7*dq4*dqr2*cos(q2)*cos(q4)*sin(q3)*sin(q5)*sin(q6))/2000 - (7*dq5*dqr2*cos(q2)*cos(q4)*sin(q3)*sin(q5)*sin(q6))/1000 - (7*dq6*dqr2*cos(q2)*cos(q4)*sin(q3)*sin(q5)*sin(q6))/2000 + dq1*dqr2*sin(2*q2)*sin(2*q3)*cos(q6)*sin(q4)*((111*3^(1/2))/8000 + 7539/40000) - dq6*dqr2*cos(q2)*cos(q5)*cos(q6)*sin(q3)*((641*3^(1/2))/40000 + 37/2000) + dq2*dqr2*cos(q2)*cos(q4)*cos(q6)*sin(q3)*((111*3^(1/2))/8000 + 7539/40000) - dq3*dqr2*cos(q2)*cos(q4)*cos(q6)*sin(q3)*((111*3^(1/2))/8000 + 7539/40000) - dq4*dqr2*cos(q2)*cos(q5)*cos(q6)*sin(q3)*((641*3^(1/2))/80000 - 37/8000) - dq5*dqr2*cos(q2)*cos(q5)*cos(q6)*sin(q3)*((641*3^(1/2))/80000 - 37/8000) - (29*dq1*dqr2*cos(2*q2)*cos(q3)*cos(q5)*cos(q6)*sin(q4))/400 + dq4*dqr2*cos(q2)*sin(q3)*sin(q5)*sin(q6)*((641*3^(1/2))/40000 + 37/2000) + dq5*dqr2*cos(q2)*sin(q3)*sin(q5)*sin(q6)*((641*3^(1/2))/40000 + 37/2000) + dq6*dqr2*cos(q2)*sin(q3)*sin(q5)*sin(q6)*((641*3^(1/2))/80000 + 37/1600) + (29*dq1*dqr2*cos(2*q2)*cos(q3)*sin(q4)*sin(q5)*sin(q6))/200 - (29*dq1*dqr2*sin(2*q2)*cos(q4)*cos(q5)*sin(q3)*sin(q6))/100 - (29*dq1*dqr2*sin(2*q2)*cos(q4)*cos(q6)*sin(q3)*sin(q5))/200 - (29*dq1*dqr2*sin(2*q2)*cos(q5)*cos(q6)*sin(q3)*sin(q4))/400 + (7*3^(1/2)*dq2*dqr2*cos(q2)*cos(q5)*cos(q6)*sin(q3))/4000 - (7*3^(1/2)*dq3*dqr2*cos(q2)*cos(q5)*cos(q6)*sin(q3))/4000 + (37*3^(1/2)*dq5*dqr2*cos(q2)*cos(q3)*cos(q6)*sin(q4))/4000 + (37*3^(1/2)*dq6*dqr2*cos(q2)*cos(q3)*cos(q6)*sin(q4))/4000 - (37*3^(1/2)*dq1*dqr2*sin(2*q2)*sin(2*q3)*sin(2*q5)*sin(q4)*sin(q6))/4000 + (37*3^(1/2)*dq2*dqr2*cos(2*q5)*cos(q2)*cos(q4)*cos(q6)*sin(q3))/8000 - (37*3^(1/2)*dq3*dqr2*cos(2*q5)*cos(q2)*cos(q4)*cos(q6)*sin(q3))/8000 - (37*3^(1/2)*dq5*dqr2*cos(2*q5)*cos(q2)*cos(q3)*cos(q6)*sin(q4))/4000 - (37*3^(1/2)*dq6*dqr2*cos(2*q5)*cos(q2)*cos(q3)*cos(q6)*sin(q4))/4000 - (37*3^(1/2)*dq2*dqr2*cos(2*q5)*cos(q2)*sin(q3)*sin(q4)*sin(q6))/2000 - (37*3^(1/2)*dq2*dqr2*sin(2*q5)*cos(q2)*cos(q4)*sin(q3)*sin(q6))/4000 - (37*3^(1/2)*dq2*dqr2*sin(2*q5)*cos(q2)*cos(q6)*sin(q3)*sin(q4))/4000 + (37*3^(1/2)*dq3*dqr2*cos(2*q5)*cos(q2)*sin(q3)*sin(q4)*sin(q6))/2000 + (37*3^(1/2)*dq3*dqr2*sin(2*q5)*cos(q2)*cos(q4)*sin(q3)*sin(q6))/4000 + (37*3^(1/2)*dq3*dqr2*sin(2*q5)*cos(q2)*cos(q6)*sin(q3)*sin(q4))/4000 + (37*3^(1/2)*dq5*dqr2*sin(2*q5)*cos(q2)*cos(q3)*sin(q4)*sin(q6))/2000 + (37*3^(1/2)*dq6*dqr2*sin(2*q5)*cos(q2)*cos(q3)*sin(q4)*sin(q6))/8000 + dq1*dqr2*cos(2*q2)*cos(2*q3)*sin(q4)*sin(q5)*sin(q6)*((37*3^(1/2))/2000 - 1231/20000) + dq1*dqr2*sin(2*q2)*sin(2*q3)*sin(q4)*sin(q5)*sin(q6)*((37*3^(1/2))/2000 - 1231/20000) + dq2*dqr2*cos(q2)*cos(q4)*sin(q3)*sin(q5)*sin(q6)*((37*3^(1/2))/2000 - 1231/20000) - dq3*dqr2*cos(q2)*cos(q4)*sin(q3)*sin(q5)*sin(q6)*((37*3^(1/2))/2000 - 1231/20000) + (37*3^(1/2)*dq1*dqr2*cos(2*q2)*cos(2*q3)*cos(2*q5)*cos(q6)*sin(q4))/8000 - dq6*dqr2*cos(2*q4)*cos(q2)*cos(q5)*cos(q6)*sin(q3)*((641*3^(1/2))/40000 + 37/2000) - dq4*dqr2*cos(2*q4)*cos(q2)*cos(q5)*cos(q6)*sin(q3)*((641*3^(1/2))/80000 - 37/8000) - dq5*dqr2*cos(2*q4)*cos(q2)*cos(q5)*cos(q6)*sin(q3)*((641*3^(1/2))/80000 - 37/8000) - (37*3^(1/2)*dq6*dqr2*cos(q2)*cos(q3)*sin(q4)*sin(q5)*sin(q6))/4000 - (37*3^(1/2)*dq1*dqr2*cos(2*q2)*cos(2*q3)*sin(2*q5)*sin(q4)*sin(q6))/4000 + (37*3^(1/2)*dq1*dqr2*cos(2*q5)*sin(2*q2)*sin(2*q3)*cos(q6)*sin(q4))/8000 + dq4*dqr2*sin(2*q4)*cos(q2)*cos(q5)*sin(q3)*sin(q6)*((641*3^(1/2))/20000 + 37/1000) - dq2*dqr2*sin(2*q4)*cos(q2)*cos(q3)*sin(q5)*sin(q6)*((641*3^(1/2))/40000 + 37/2000) + dq3*dqr2*sin(2*q4)*cos(q2)*cos(q3)*sin(q5)*sin(q6)*((641*3^(1/2))/40000 + 37/2000) + dq4*dqr2*cos(2*q4)*cos(q2)*sin(q3)*sin(q5)*sin(q6)*((641*3^(1/2))/40000 + 37/2000) + dq5*dqr2*cos(2*q4)*cos(q2)*sin(q3)*sin(q5)*sin(q6)*((641*3^(1/2))/40000 + 37/2000) + dq4*dqr2*sin(2*q4)*cos(q2)*cos(q6)*sin(q3)*sin(q5)*((641*3^(1/2))/40000 - 37/4000) + dq5*dqr2*sin(2*q4)*cos(q2)*cos(q5)*sin(q3)*sin(q6)*((641*3^(1/2))/80000 + 37/4000) + dq6*dqr2*sin(2*q4)*cos(q2)*cos(q6)*sin(q3)*sin(q5)*((641*3^(1/2))/80000 + 37/4000) + dq6*dqr2*cos(2*q4)*cos(q2)*sin(q3)*sin(q5)*sin(q6)*((641*3^(1/2))/80000 - 37/8000) + dq5*dqr2*sin(2*q4)*cos(q2)*cos(q6)*sin(q3)*sin(q5)*((641*3^(1/2))/160000 - 37/16000) + dq6*dqr2*sin(2*q4)*cos(q2)*cos(q5)*sin(q3)*sin(q6)*((641*3^(1/2))/160000 - 37/16000);
